simulink library "outp"  (R2021b)
(part 9 of 11)

      link override Signal_Limit/_maxval: Value=KOUTP_CalibratedAccX_G_maxval
      link override Signal_Limit/_minval: Value=KOUTP_CalibratedAccX_G_minval
      link override Signal_Override/_ovrdflg: Value=KOUTP_CalibratedAccX_G_ovrdflg
      link override Signal_Override/_ovrdval: Value=KOUTP_CalibratedAccX_G_ovrdval
  VVMC_CalibratedAccY_G_Inproc : FVT_lib/outp/OverrideAndLimit  SystemSampleTime=-1  VariantActivationTime=update diagram  Latency=0  AutoFrameSizeCalculation=off
      link override Signal_Limit/_maxval: Value=KOUTP_CalibratedAccY_G_maxval
      link override Signal_Limit/_minval: Value=KOUTP_CalibratedAccY_G_minval
      link override Signal_Override/_ovrdflg: Value=KOUTP_CalibratedAccY_G_ovrdflg
      link override Signal_Override/_ovrdval: Value=KOUTP_CalibratedAccY_G_ovrdval
  VVMC_CalibratedAccZ_G_Inproc : FVT_lib/outp/OverrideAndLimit  SystemSampleTime=-1  VariantActivationTime=update diagram  Latency=0  AutoFrameSizeCalculation=off
      link override Signal_Limit/_maxval: Value=KOUTP_CalibratedAccZ_G_maxval
      link override Signal_Limit/_minval: Value=KOUTP_CalibratedAccZ_G_minval
      link override Signal_Override/_ovrdflg: Value=KOUTP_CalibratedAccZ_G_ovrdflg
      link override Signal_Override/_ovrdval: Value=KOUTP_CalibratedAccZ_G_ovrdval
  VVMC_CalibratedGyroX_Dps_Inproc : FVT_lib/outp/OverrideAndLimit  SystemSampleTime=-1  VariantActivationTime=update diagram  Latency=0  AutoFrameSizeCalculation=off
      link override Signal_Limit/_maxval: Value=KOUTP_CalibratedGyroX_Dps_maxval
      link override Signal_Limit/_minval: Value=KOUTP_CalibratedGyroX_Dps_minval
      link override Signal_Override/_ovrdflg: Value=KOUTP_CalibratedGyroX_Dps_ovrdflg
      link override Signal_Override/_ovrdval: Value=KOUTP_CalibratedGyroX_Dps_ovrdval
  VVMC_CalibratedGyroY_Dps_Inproc : FVT_lib/outp/OverrideAndLimit  SystemSampleTime=-1  VariantActivationTime=update diagram  Latency=0  AutoFrameSizeCalculation=off
      link override Signal_Limit/_maxval: Value=KOUTP_CalibratedGyroY_Dps_maxval
      link override Signal_Limit/_minval: Value=KOUTP_CalibratedGyroY_Dps_minval
      link override Signal_Override/_ovrdflg: Value=KOUTP_CalibratedGyroY_Dps_ovrdflg
      link override Signal_Override/_ovrdval: Value=KOUTP_CalibratedGyroY_Dps_ovrdval
  VVMC_CalibratedGyroZ_Dps_Inproc : FVT_lib/outp/OverrideAndLimit  SystemSampleTime=-1  VariantActivationTime=update diagram  Latency=0  AutoFrameSizeCalculation=off
      link override Signal_Limit/_maxval: Value=KOUTP_CalibratedGyroZ_Dps_maxval
      link override Signal_Limit/_minval: Value=KOUTP_CalibratedGyroZ_Dps_minval
      link override Signal_Override/_ovrdflg: Value=KOUTP_CalibratedGyroZ_Dps_ovrdflg
      link override Signal_Override/_ovrdval: Value=KOUTP_CalibratedGyroZ_Dps_ovrdval
  VVMC_DISCReqAcc_mps2_Inproc : FVT_lib/outp/OverrideAndLimit  SystemSampleTime=-1  VariantActivationTime=update diagram  Latency=0  AutoFrameSizeCalculation=off
      link override Signal_Limit/_maxval: Value=KOUTP_DISCReqAcc_mps2_maxval
      link override Signal_Limit/_minval: Value=KOUTP_DISCReqAcc_mps2_minval
      link override Signal_Override/_ovrdflg: Value=KOUTP_DISCReqAcc_mps2_ovrdflg
      link override Signal_Override/_ovrdval: Value=KOUTP_DISCReqAcc_mps2_ovrdval
  VVMC_ExtraMSACtrlSta_enum_Inproc : FVT_lib/outp/OverrideAndLimit  SystemSampleTime=-1  VariantActivationTime=update diagram  Latency=0  AutoFrameSizeCalculation=off
      link override Signal_Limit/_maxval: Value=KOUTP_ExtraMSACtrlSta_enum_maxval
      link override Signal_Limit/_minval: Value=KOUTP_ExtraMSACtrlSta_enum_minval
      link override Signal_Override/_ovrdflg: Value=KOUTP_ExtraMSACtrlSta_enum_ovrdflg
      link override Signal_Override/_ovrdval: Value=KOUTP_ExtraMSACtrlSta_enum_ovrdval
  VVMC_FCMACCmode_enum_Inproc : FVT_lib/outp/OverrideAndLimit  SystemSampleTime=-1  VariantActivationTime=update diagram  Latency=0  AutoFrameSizeCalculation=off
      link override Signal_Limit/_maxval: Value=KOUTP_FCMACCmode_enum_maxval
      link override Signal_Limit/_minval: Value=KOUTP_FCMACCmode_enum_minval
      link override Signal_Override/_ovrdflg: Value=KOUTP_FCMACCmode_enum_ovrdflg
      link override Signal_Override/_ovrdval: Value=KOUTP_FCMACCmode_enum_ovrdval
  VVMC_FCMLDWFault_flg_Inproc : FVT_lib/outp/OverrideAndLimit  SystemSampleTime=-1  VariantActivationTime=update diagram  Latency=0  AutoFrameSizeCalculation=off
      link override Signal_Limit/_maxval: Value=KOUTP_FCMLDWFault_flg_maxval
      link override Signal_Limit/_minval: Value=KOUTP_FCMLDWFault_flg_minval
      link override Signal_Override/_ovrdflg: Value=KOUTP_FCMLDWFault_flg_ovrdflg
      link override Signal_Override/_ovrdval: Value=KOUTP_FCMLDWFault_flg_ovrdval
  VVMC_FCMLDWRequest_enum_Inproc : FVT_lib/outp/OverrideAndLimit  SystemSampleTime=-1  VariantActivationTime=update diagram  Latency=0  AutoFrameSizeCalculation=off
      link override Signal_Limit/_maxval: Value=KOUTP_FCMLDWRequest_enum_maxval
      link override Signal_Limit/_minval: Value=KOUTP_FCMLDWRequest_enum_minval
      link override Signal_Override/_ovrdflg: Value=KOUTP_FCMLDWRequest_enum_ovrdflg
      link override Signal_Override/_ovrdval: Value=KOUTP_FCMLDWRequest_enum_ovrdval
  VVMC_FDCVMCAPSAngleTarget_deg_Inproc : FVT_lib/outp/OverrideAndLimit  SystemSampleTime=-1  VariantActivationTime=update diagram  Latency=0  AutoFrameSizeCalculation=off
      link override Signal_Limit/_maxval: Value=KOUTP_FDCVMCAPSAngleTarget_deg_maxval
      link override Signal_Limit/_minval: Value=KOUTP_FDCVMCAPSAngleTarget_deg_minval
      link override Signal_Override/_ovrdflg: Value=KOUTP_FDCVMCAPSAngleTarget_deg_ovrdflg
      link override Signal_Override/_ovrdval: Value=KOUTP_FDCVMCAPSAngleTarget_deg_ovrdval
  VVMC_FDCVMCAPSRqEPSCtrl_flg_Inproc : FVT_lib/outp/OverrideAndLimit  SystemSampleTime=-1  VariantActivationTime=update diagram  Latency=0  AutoFrameSizeCalculation=off
      link override Signal_Limit/_maxval: Value=KOUTP_FDCVMCAPSRqEPSCtrl_flg_maxval
      link override Signal_Limit/_minval: Value=KOUTP_FDCVMCAPSRqEPSCtrl_flg_minval
      link override Signal_Override/_ovrdflg: Value=KOUTP_FDCVMCAPSRqEPSCtrl_flg_ovrdflg
      link override Signal_Override/_ovrdval: Value=KOUTP_FDCVMCAPSRqEPSCtrl_flg_ovrdval
  VVMC_FDCVMCAPSVRqEPSCtrl_flg_Inproc : FVT_lib/outp/OverrideAndLimit  SystemSampleTime=-1  VariantActivationTime=update diagram  Latency=0  AutoFrameSizeCalculation=off
      link override Signal_Limit/_maxval: Value=KOUTP_FDCVMCAPSVRqEPSCtrl_flg_maxval
      link override Signal_Limit/_minval: Value=KOUTP_FDCVMCAPSVRqEPSCtrl_flg_minval
      link override Signal_Override/_ovrdflg: Value=KOUTP_FDCVMCAPSVRqEPSCtrl_flg_ovrdflg
      link override Signal_Override/_ovrdval: Value=KOUTP_FDCVMCAPSVRqEPSCtrl_flg_ovrdval
  VVMC_FDCVMCAngCtrlTqWtGn_pct_Inproc : FVT_lib/outp/OverrideAndLimit  SystemSampleTime=-1  VariantActivationTime=update diagram  Latency=0  AutoFrameSizeCalculation=off
      link override Signal_Limit/_maxval: Value=KOUTP_FDCVMCAngCtrlTqWtGn_pct_maxval
      link override Signal_Limit/_minval: Value=KOUTP_FDCVMCAngCtrlTqWtGn_pct_minval
      link override Signal_Override/_ovrdflg: Value=KOUTP_FDCVMCAngCtrlTqWtGn_pct_ovrdflg
      link override Signal_Override/_ovrdval: Value=KOUTP_FDCVMCAngCtrlTqWtGn_pct_ovrdval
  VVMC_FDCVMCDrInpTqBstAct_flg_Inproc : FVT_lib/outp/OverrideAndLimit  SystemSampleTime=-1  VariantActivationTime=update diagram  Latency=0  AutoFrameSizeCalculation=off
      link override Signal_Limit/_maxval: Value=KOUTP_FDCVMCDrInpTqBstAct_flg_maxval
      link override Signal_Limit/_minval: Value=KOUTP_FDCVMCDrInpTqBstAct_flg_minval
      link override Signal_Override/_ovrdflg: Value=KOUTP_FDCVMCDrInpTqBstAct_flg_ovrdflg
      link override Signal_Override/_ovrdval: Value=KOUTP_FDCVMCDrInpTqBstAct_flg_ovrdval
  VVMC_FDCVMCDrInpTqBstGn_pct_Inproc : FVT_lib/outp/OverrideAndLimit  SystemSampleTime=-1  VariantActivationTime=update diagram  Latency=0  AutoFrameSizeCalculation=off
      link override Signal_Limit/_maxval: Value=KOUTP_FDCVMCDrInpTqBstGn_pct_maxval
      link override Signal_Limit/_minval: Value=KOUTP_FDCVMCDrInpTqBstGn_pct_minval
      link override Signal_Override/_ovrdflg: Value=KOUTP_FDCVMCDrInpTqBstGn_pct_ovrdflg
      link override Signal_Override/_ovrdval: Value=KOUTP_FDCVMCDrInpTqBstGn_pct_ovrdval
  VVMC_FDCVMCMaxAngCtrlOutTqLim_Nm_Inproc : FVT_lib/outp/OverrideAndLimit  SystemSampleTime=-1  VariantActivationTime=update diagram  Latency=0  AutoFrameSizeCalculation=off
      link override Signal_Limit/_maxval: Value=KOUTP_FDCVMCMaxAngCtrlOutTqLim_Nm_maxval
      link override Signal_Limit/_minval: Value=KOUTP_FDCVMCMaxAngCtrlOutTqLim_Nm_minval
      link override Signal_Override/_ovrdflg: Value=KOUTP_FDCVMCMaxAngCtrlOutTqLim_Nm_ovrdflg
      link override Signal_Override/_ovrdval: Value=KOUTP_FDCVMCMaxAngCtrlOutTqLim_Nm_ovrdval
  VVMC_FeatArbitrFinal_enum_Inproc : FVT_lib/outp/OverrideAndLimit  SystemSampleTime=-1  VariantActivationTime=update diagram  Latency=0  AutoFrameSizeCalculation=off
      link override Signal_Limit/_maxval: Value=KOUTP_FeatArbitrFinal_enum_maxval
      link override Signal_Limit/_minval: Value=KOUTP_FeatArbitrFinal_enum_minval
      link override Signal_Override/_ovrdflg: Value=KOUTP_FeatArbitrFinal_enum_ovrdflg
      link override Signal_Override/_ovrdval: Value=KOUTP_FeatArbitrFinal_enum_ovrdval
  VVMC_FeatArbitrSta_enum_Inproc : FVT_lib/outp/OverrideAndLimit  SystemSampleTime=-1  VariantActivationTime=update diagram  Latency=0  AutoFrameSizeCalculation=off
      link override Signal_Limit/_maxval: Value=KOUTP_FeatArbitrSta_enum_maxval
      link override Signal_Limit/_minval: Value=KOUTP_FeatArbitrSta_enum_minval
      link override Signal_Override/_ovrdflg: Value=KOUTP_FeatArbitrSta_enum_ovrdflg
      link override Signal_Override/_ovrdval: Value=KOUTP_FeatArbitrSta_enum_ovrdval
  VVMC_FeatReqSpd_kph_Inproc : FVT_lib/outp/OverrideAndLimit  SystemSampleTime=-1  VariantActivationTime=update diagram  Latency=0  AutoFrameSizeCalculation=off
      link override Signal_Limit/_maxval: Value=KOUTP_FeatReqSpd_kph_maxval
      link override Signal_Limit/_minval: Value=KOUTP_FeatReqSpd_kph_minval
      link override Signal_Override/_ovrdflg: Value=KOUTP_FeatReqSpd_kph_ovrdflg
      link override Signal_Override/_ovrdval: Value=KOUTP_FeatReqSpd_kph_ovrdval
  VVMC_FeatSetSpdFinal_raw32_Inproc : FVT_lib/outp/OverrideAndLimit  SystemSampleTime=-1  VariantActivationTime=update diagram  Latency=0  AutoFrameSizeCalculation=off
      link override Signal_Limit/_maxval: Value=KOUTP_FeatSetSpdFinal_raw32_maxval
      link override Signal_Limit/_minval: Value=KOUTP_FeatSetSpdFinal_raw32_minval
      link override Signal_Override/_ovrdflg: Value=KOUTP_FeatSetSpdFinal_raw32_ovrdflg
      link override Signal_Override/_ovrdval: Value=KOUTP_FeatSetSpdFinal_raw32_ovrdval
  VVMC_ForceLowBeam_enum_Inproc : FVT_lib/outp/OverrideAndLimit  SystemSampleTime=-1  VariantActivationTime=update diagram  Latency=0  AutoFrameSizeCalculation=off
      link override Signal_Limit/_maxval: Value=KOUTP_ForceLowBeam_enum_maxval
      link override Signal_Limit/_minval: Value=KOUTP_ForceLowBeam_enum_minval
      link override Signal_Override/_ovrdflg: Value=KOUTP_ForceLowBeam_enum_ovrdflg
      link override Signal_Override/_ovrdval: Value=KOUTP_ForceLowBeam_enum_ovrdval
  VVMC_FrontRearSlipRatioCtrl_flg_Inproc : FVT_lib/outp/OverrideAndLimit  SystemSampleTime=-1  VariantActivationTime=update diagram  Latency=0  AutoFrameSizeCalculation=off
      link override Signal_Limit/_maxval: Value=KOUTP_FrontRearSlipRatioCtrl_flg_maxval
      link override Signal_Limit/_minval: Value=KOUTP_FrontRearSlipRatioCtrl_flg_minval
      link override Signal_Override/_ovrdflg: Value=KOUTP_FrontRearSlipRatioCtrl_flg_ovrdflg
      link override Signal_Override/_ovrdval: Value=KOUTP_FrontRearSlipRatioCtrl_flg_ovrdval
  VVMC_HazardWarningReq_flg_Inproc : FVT_lib/outp/OverrideAndLimit  SystemSampleTime=-1  VariantActivationTime=update diagram  Latency=0  AutoFrameSizeCalculation=off
      link override Signal_Limit/_maxval: Value=KOUTP_HazardWarningReq_flg_maxval
      link override Signal_Limit/_minval: Value=KOUTP_HazardWarningReq_flg_minval
      link override Signal_Override/_ovrdflg: Value=KOUTP_HazardWarningReq_flg_ovrdflg
      link override Signal_Override/_ovrdval: Value=KOUTP_HazardWarningReq_flg_ovrdval
  VVMC_IMUEnaCmd_flg_Inproc : FVT_lib/outp/OverrideAndLimit  SystemSampleTime=-1  VariantActivationTime=update diagram  Latency=0  AutoFrameSizeCalculation=off
      link override Signal_Limit/_maxval: Value=KOUTP_IMUEnaCmd_flg_maxval
      link override Signal_Limit/_minval: Value=KOUTP_IMUEnaCmd_flg_minval
      link override Signal_Override/_ovrdflg: Value=KOUTP_IMUEnaCmd_flg_ovrdflg
      link override Signal_Override/_ovrdval: Value=KOUTP_IMUEnaCmd_flg_ovrdval
  VVMC_ISOAccLimit_mps2_Inproc : FVT_lib/outp/OverrideAndLimit  SystemSampleTime=-1  VariantActivationTime=update diagram  Latency=0  AutoFrameSizeCalculation=off
      link override Signal_Limit/_maxval: Value=KOUTP_ISOAccLimit_mps2_maxval
      link override Signal_Limit/_minval: Value=KOUTP_ISOAccLimit_mps2_minval
      link override Signal_Override/_ovrdflg: Value=KOUTP_ISOAccLimit_mps2_ovrdflg
      link override Signal_Override/_ovrdval: Value=KOUTP_ISOAccLimit_mps2_ovrdval
  VVMC_ISODecLimit_mps2_Inproc : FVT_lib/outp/OverrideAndLimit  SystemSampleTime=-1  VariantActivationTime=update diagram  Latency=0  AutoFrameSizeCalculation=off
      link override Signal_Limit/_maxval: Value=KOUTP_ISODecLimit_mps2_maxval
      link override Signal_Limit/_minval: Value=KOUTP_ISODecLimit_mps2_minval
      link override Signal_Override/_ovrdflg: Value=KOUTP_ISODecLimit_mps2_ovrdflg
      link override Signal_Override/_ovrdval: Value=KOUTP_ISODecLimit_mps2_ovrdval
  VVMC_ISOJerkLimit_mps3_Inproc : FVT_lib/outp/OverrideAndLimit  SystemSampleTime=-1  VariantActivationTime=update diagram  Latency=0  AutoFrameSizeCalculation=off
      link override Signal_Limit/_maxval: Value=KOUTP_ISOJerkLimit_mps3_maxval
      link override Signal_Limit/_minval: Value=KOUTP_ISOJerkLimit_mps3_minval
      link override Signal_Override/_ovrdflg: Value=KOUTP_ISOJerkLimit_mps3_ovrdflg
      link override Signal_Override/_ovrdval: Value=KOUTP_ISOJerkLimit_mps3_ovrdval
  VVMC_JerkPCT_pct_Inproc : FVT_lib/outp/OverrideAndLimit  SystemSampleTime=-1  VariantActivationTime=update diagram  Latency=0  AutoFrameSizeCalculation=off
      link override Signal_Limit/_maxval: Value=KOUTP_JerkPCT_pct_maxval
      link override Signal_Limit/_minval: Value=KOUTP_JerkPCT_pct_minval
      link override Signal_Override/_ovrdflg: Value=KOUTP_JerkPCT_pct_ovrdflg
      link override Signal_Override/_ovrdval: Value=KOUTP_JerkPCT_pct_ovrdval
  VVMC_LKAHODDisplayWarning_flg_Inproc : FVT_lib/outp/OverrideAndLimit  SystemSampleTime=-1  VariantActivationTime=update diagram  Latency=0  AutoFrameSizeCalculation=off
      link override Signal_Limit/_maxval: Value=KOUTP_LKAHODDisplayWarning_flg_maxval
      link override Signal_Limit/_minval: Value=KOUTP_LKAHODDisplayWarning_flg_minval
      link override Signal_Override/_ovrdflg: Value=KOUTP_LKAHODDisplayWarning_flg_ovrdflg
      link override Signal_Override/_ovrdval: Value=KOUTP_LKAHODDisplayWarning_flg_ovrdval
  VVMC_LKAHODSoundWarning_flg_Inproc : FVT_lib/outp/OverrideAndLimit  SystemSampleTime=-1  VariantActivationTime=update diagram  Latency=0  AutoFrameSizeCalculation=off
      link override Signal_Limit/_maxval: Value=KOUTP_LKAHODSoundWarning_flg_maxval
      link override Signal_Limit/_minval: Value=KOUTP_LKAHODSoundWarning_flg_minval
      link override Signal_Override/_ovrdflg: Value=KOUTP_LKAHODSoundWarning_flg_ovrdflg
      link override Signal_Override/_ovrdval: Value=KOUTP_LKAHODSoundWarning_flg_ovrdval
  VVMC_LKAStrToqReq_Nm_Inproc : FVT_lib/outp/OverrideAndLimit  SystemSampleTime=-1  VariantActivationTime=update diagram  Latency=0  AutoFrameSizeCalculation=off
      link override Signal_Limit/_maxval: Value=KOUTP_LKAStrToqReq_Nm_maxval
      link override Signal_Limit/_minval: Value=KOUTP_LKAStrToqReq_Nm_minval
      link override Signal_Override/_ovrdflg: Value=KOUTP_LKAStrToqReq_Nm_ovrdflg
      link override Signal_Override/_ovrdval: Value=KOUTP_LKAStrToqReq_Nm_ovrdval
  VVMC_LKATOIAct_enum_Inproc : FVT_lib/outp/OverrideAndLimit  SystemSampleTime=-1  VariantActivationTime=update diagram  Latency=0  AutoFrameSizeCalculation=off
      link override Signal_Limit/_maxval: Value=KOUTP_LKATOIAct_enum_maxval
      link override Signal_Limit/_minval: Value=KOUTP_LKATOIAct_enum_minval
      link override Signal_Override/_ovrdflg: Value=KOUTP_LKATOIAct_enum_ovrdflg
      link override Signal_Override/_ovrdval: Value=KOUTP_LKATOIAct_enum_ovrdval
  VVMC_LKATOIFault_flg_Inproc : FVT_lib/outp/OverrideAndLimit  SystemSampleTime=-1  VariantActivationTime=update diagram  Latency=0  AutoFrameSizeCalculation=off
      link override Signal_Limit/_maxval: Value=KOUTP_LKATOIFault_flg_maxval
      link override Signal_Limit/_minval: Value=KOUTP_LKATOIFault_flg_minval
      link override Signal_Override/_ovrdflg: Value=KOUTP_LKATOIFault_flg_ovrdflg
      link override Signal_Override/_ovrdval: Value=KOUTP_LKATOIFault_flg_ovrdval
  VVMC_LVDAACCStatusInformation_flg_Inproc : FVT_lib/outp/OverrideAndLimit  SystemSampleTime=-1  VariantActivationTime=update diagram  Latency=0  AutoFrameSizeCalculation=off
      link override Signal_Limit/_maxval: Value=KOUTP_LVDAACCStatusInformation_flg_maxval
      link override Signal_Limit/_minval: Value=KOUTP_LVDAACCStatusInformation_flg_minval
      link override Signal_Override/_ovrdflg: Value=KOUTP_LVDAACCStatusInformation_flg_ovrdflg
      link override Signal_Override/_ovrdval: Value=KOUTP_LVDAACCStatusInformation_flg_ovrdval
  VVMC_LVDADisabled_flg_Inproc : FVT_lib/outp/OverrideAndLimit  SystemSampleTime=-1  VariantActivationTime=update diagram  Latency=0  AutoFrameSizeCalculation=off
      link override Signal_Limit/_maxval: Value=KOUTP_LVDADisabled_flg_maxval
      link override Signal_Limit/_minval: Value=KOUTP_LVDADisabled_flg_minval
      link override Signal_Override/_ovrdflg: Value=KOUTP_LVDADisabled_flg_ovrdflg
      link override Signal_Override/_ovrdval: Value=KOUTP_LVDADisabled_flg_ovrdval
  VVMC_LVDAFailinfo_flg_Inproc : FVT_lib/outp/OverrideAndLimit  SystemSampleTime=-1  VariantActivationTime=update diagram  Latency=0  AutoFrameSizeCalculation=off
      link override Signal_Limit/_maxval: Value=KOUTP_LVDAFailinfo_flg_maxval
      link override Signal_Limit/_minval: Value=KOUTP_LVDAFailinfo_flg_minval
      link override Signal_Override/_ovrdflg: Value=KOUTP_LVDAFailinfo_flg_ovrdflg
      link override Signal_Override/_ovrdval: Value=KOUTP_LVDAFailinfo_flg_ovrdval
  VVMC_LVDAMuteSta_enum_Inproc : FVT_lib/outp/OverrideAndLimit  SystemSampleTime=-1  VariantActivationTime=update diagram  Latency=0  AutoFrameSizeCalculation=off
      link override Signal_Limit/_maxval: Value=KOUTP_LVDAMuteSta_enum_maxval
      link override Signal_Limit/_minval: Value=KOUTP_LVDAMuteSta_enum_minval
      link override Signal_Override/_ovrdflg: Value=KOUTP_LVDAMuteSta_enum_ovrdflg
      link override Signal_Override/_ovrdval: Value=KOUTP_LVDAMuteSta_enum_ovrdval
  VVMC_LVDAWarning_flg_Inproc : FVT_lib/outp/OverrideAndLimit  SystemSampleTime=-1  VariantActivationTime=update diagram  Latency=0  AutoFrameSizeCalculation=off
      link override Signal_Limit/_maxval: Value=KOUTP_LVDAWarning_flg_maxval
      link override Signal_Limit/_minval: Value=KOUTP_LVDAWarning_flg_minval
      link override Signal_Override/_ovrdflg: Value=KOUTP_LVDAWarning_flg_ovrdflg
      link override Signal_Override/_ovrdval: Value=KOUTP_LVDAWarning_flg_ovrdval
  VVMC_LatAccCtrl_flg_Inproc : FVT_lib/outp/OverrideAndLimit  SystemSampleTime=-1  VariantActivationTime=update diagram  Latency=0  AutoFrameSizeCalculation=off
      link override Signal_Limit/_maxval: Value=KOUTP_LatAccCtrl_flg_maxval
      link override Signal_Limit/_minval: Value=KOUTP_LatAccCtrl_flg_minval
      link override Signal_Override/_ovrdflg: Value=KOUTP_LatAccCtrl_flg_ovrdflg
      link override Signal_Override/_ovrdval: Value=KOUTP_LatAccCtrl_flg_ovrdval
  VVMC_LateralCtrl_flg_Inproc : FVT_lib/outp/OverrideAndLimit  SystemSampleTime=-1  VariantActivationTime=update diagram  Latency=0  AutoFrameSizeCalculation=off
      link override Signal_Limit/_maxval: Value=KOUTP_LateralCtrl_flg_maxval
      link override Signal_Limit/_minval: Value=KOUTP_LateralCtrl_flg_minval
      link override Signal_Override/_ovrdflg: Value=KOUTP_LateralCtrl_flg_ovrdflg
      link override Signal_Override/_ovrdval: Value=KOUTP_LateralCtrl_flg_ovrdval
  VVMC_LeftTurnLightReq_flg_Inproc : FVT_lib/outp/OverrideAndLimit  SystemSampleTime=-1  VariantActivationTime=update diagram  Latency=0  AutoFrameSizeCalculation=off
      link override Signal_Limit/_maxval: Value=KOUTP_LeftTurnLightReq_flg_maxval
      link override Signal_Limit/_minval: Value=KOUTP_LeftTurnLightReq_flg_minval
      link override Signal_Override/_ovrdflg: Value=KOUTP_LeftTurnLightReq_flg_ovrdflg
      link override Signal_Override/_ovrdval: Value=KOUTP_LeftTurnLightReq_flg_ovrdval
  VVMC_LimitPCT_pct_Inproc : FVT_lib/outp/OverrideAndLimit  SystemSampleTime=-1  VariantActivationTime=update diagram  Latency=0  AutoFrameSizeCalculation=off
      link override Signal_Limit/_maxval: Value=KOUTP_LimitPCT_pct_maxval
      link override Signal_Limit/_minval: Value=KOUTP_LimitPCT_pct_minval
      link override Signal_Override/_ovrdflg: Value=KOUTP_LimitPCT_pct_ovrdflg
      link override Signal_Override/_ovrdval: Value=KOUTP_LimitPCT_pct_ovrdval
  VVMC_LongAcc_Gps_Inproc : FVT_lib/outp/OverrideAndLimit  SystemSampleTime=-1  VariantActivationTime=update diagram  Latency=0  AutoFrameSizeCalculation=off
      link override Signal_Limit/_maxval: Value=KOUTP_LongAcc_Gps_maxval
      link override Signal_Limit/_minval: Value=KOUTP_LongAcc_Gps_minval
      link override Signal_Override/_ovrdflg: Value=KOUTP_LongAcc_Gps_ovrdflg
      link override Signal_Override/_ovrdval: Value=KOUTP_LongAcc_Gps_ovrdval
  VVMC_MSACtrlSta_enum_Inproc : FVT_lib/outp/OverrideAndLimit  SystemSampleTime=-1  VariantActivationTime=update diagram  Latency=0  AutoFrameSizeCalculation=off
      link override Signal_Limit/_maxval: Value=KOUTP_MSACtrlSta_enum_maxval
      link override Signal_Limit/_minval: Value=KOUTP_MSACtrlSta_enum_minval
      link override Signal_Override/_ovrdflg: Value=KOUTP_MSACtrlSta_enum_ovrdflg
      link override Signal_Override/_ovrdval: Value=KOUTP_MSACtrlSta_enum_ovrdval
  VVMC_MeterIndSpeed_raw32_Inproc : FVT_lib/outp/OverrideAndLimit  SystemSampleTime=-1  VariantActivationTime=update diagram  Latency=0  AutoFrameSizeCalculation=off
      link override Signal_Limit/_maxval: Value=KOUTP_MeterIndSpeed_raw32_maxval
      link override Signal_Limit/_minval: Value=KOUTP_MeterIndSpeed_raw32_minval
      link override Signal_Override/_ovrdflg: Value=KOUTP_MeterIndSpeed_raw32_ovrdflg
      link override Signal_Override/_ovrdval: Value=KOUTP_MeterIndSpeed_raw32_ovrdval
  VVMC_RearWhlSlipRatioCtrl_flg_Inproc : FVT_lib/outp/OverrideAndLimit  SystemSampleTime=-1  VariantActivationTime=update diagram  Latency=0  AutoFrameSizeCalculation=off
      link override Signal_Limit/_maxval: Value=KOUTP_RearWhlSlipRatioCtrl_flg_maxval
      link override Signal_Limit/_minval: Value=KOUTP_RearWhlSlipRatioCtrl_flg_minval
      link override Signal_Override/_ovrdflg: Value=KOUTP_RearWhlSlipRatioCtrl_flg_ovrdflg
      link override Signal_Override/_ovrdval: Value=KOUTP_RearWhlSlipRatioCtrl_flg_ovrdval
  VVMC_RightTurnLightReq_flg_Inproc : FVT_lib/outp/OverrideAndLimit  SystemSampleTime=-1  VariantActivationTime=update diagram  Latency=0  AutoFrameSizeCalculation=off
      link override Signal_Limit/_maxval: Value=KOUTP_RightTurnLightReq_flg_maxval
      link override Signal_Limit/_minval: Value=KOUTP_RightTurnLightReq_flg_minval
      link override Signal_Override/_ovrdflg: Value=KOUTP_RightTurnLightReq_flg_ovrdflg
      link override Signal_Override/_ovrdval: Value=KOUTP_RightTurnLightReq_flg_ovrdval
  VVMC_SPD2ACCAct_flg_Inproc : FVT_lib/outp/OverrideAndLimit  SystemSampleTime=-1  VariantActivationTime=update diagram  Latency=0  AutoFrameSizeCalculation=off
      link override Signal_Limit/_maxval: Value=KOUTP_SPD2ACCAct_flg_maxval
      link override Signal_Limit/_minval: Value=KOUTP_SPD2ACCAct_flg_minval
      link override Signal_Override/_ovrdflg: Value=KOUTP_SPD2ACCAct_flg_ovrdflg
      link override Signal_Override/_ovrdval: Value=KOUTP_SPD2ACCAct_flg_ovrdval
  VVMC_SafetyCtrl_flg_Inproc : FVT_lib/outp/OverrideAndLimit  SystemSampleTime=-1  VariantActivationTime=update diagram  Latency=0  AutoFrameSizeCalculation=off
      link override Signal_Limit/_maxval: Value=KOUTP_SafetyCtrl_flg_maxval
      link override Signal_Limit/_minval: Value=KOUTP_SafetyCtrl_flg_minval
      link override Signal_Override/_ovrdflg: Value=KOUTP_SafetyCtrl_flg_ovrdflg
      link override Signal_Override/_ovrdval: Value=KOUTP_SafetyCtrl_flg_ovrdval
  VVMC_SingleWhlSlipRatioCtrl_flg_Inproc : FVT_lib/outp/OverrideAndLimit  SystemSampleTime=-1  VariantActivationTime=update diagram  Latency=0  AutoFrameSizeCalculation=off
      link override Signal_Limit/_maxval: Value=KOUTP_SingleWhlSlipRatioCtrl_flg_maxval
      link override Signal_Limit/_minval: Value=KOUTP_SingleWhlSlipRatioCtrl_flg_minval
      link override Signal_Override/_ovrdflg: Value=KOUTP_SingleWhlSlipRatioCtrl_flg_ovrdflg
      link override Signal_Override/_ovrdval: Value=KOUTP_SingleWhlSlipRatioCtrl_flg_ovrdval
  VVMC_TargetType_enum_Inproc : FVT_lib/outp/OverrideAndLimit  SystemSampleTime=-1  VariantActivationTime=update diagram  Latency=0  AutoFrameSizeCalculation=off
      link override Signal_Limit/_maxval: Value=KOUTP_TargetType_enum_maxval
      link override Signal_Limit/_minval: Value=KOUTP_TargetType_enum_minval
      link override Signal_Override/_ovrdflg: Value=KOUTP_TargetType_enum_ovrdflg
      link override Signal_Override/_ovrdval: Value=KOUTP_TargetType_enum_ovrdval
  VVMC_TimeGapCalcu_s_Inproc : FVT_lib/outp/OverrideAndLimit  SystemSampleTime=-1  VariantActivationTime=update diagram  Latency=0  AutoFrameSizeCalculation=off
      link override Signal_Limit/_maxval: Value=KOUTP_TimeGapCalcu_s_maxval
      link override Signal_Limit/_minval: Value=KOUTP_TimeGapCalcu_s_minval
      link override Signal_Override/_ovrdflg: Value=KOUTP_TimeGapCalcu_s_ovrdflg
      link override Signal_Override/_ovrdval: Value=KOUTP_TimeGapCalcu_s_ovrdval
  VVMC_TimeGapLevel_enum_Inproc : FVT_lib/outp/OverrideAndLimit  SystemSampleTime=-1  VariantActivationTime=update diagram  Latency=0  AutoFrameSizeCalculation=off
      link override Signal_Limit/_maxval: Value=KOUTP_TimeGapLevel_enum_maxval
      link override Signal_Limit/_minval: Value=KOUTP_TimeGapLevel_enum_minval
      link override Signal_Override/_ovrdflg: Value=KOUTP_TimeGapLevel_enum_ovrdflg
      link override Signal_Override/_ovrdval: Value=KOUTP_TimeGapLevel_enum_ovrdval
  VVMC_VMCACCCtrlAvail_flg_Inproc : FVT_lib/outp/OverrideAndLimit  SystemSampleTime=-1  VariantActivationTime=update diagram  Latency=0  AutoFrameSizeCalculation=off
      link override Signal_Limit/_maxval: Value=KOUTP_VMCACCCtrlAvail_flg_maxval
      link override Signal_Limit/_minval: Value=KOUTP_VMCACCCtrlAvail_flg_minval
      link override Signal_Override/_ovrdflg: Value=KOUTP_VMCACCCtrlAvail_flg_ovrdflg
      link override Signal_Override/_ovrdval: Value=KOUTP_VMCACCCtrlAvail_flg_ovrdval
  VVMC_VMCAEBCtrlAvail_flg_Inproc : FVT_lib/outp/OverrideAndLimit  SystemSampleTime=-1  VariantActivationTime=update diagram  Latency=0  AutoFrameSizeCalculation=off
      link override Signal_Limit/_maxval: Value=KOUTP_VMCAEBCtrlAvail_flg_maxval
      link override Signal_Limit/_minval: Value=KOUTP_VMCAEBCtrlAvail_flg_minval
      link override Signal_Override/_ovrdflg: Value=KOUTP_VMCAEBCtrlAvail_flg_ovrdflg
      link override Signal_Override/_ovrdval: Value=KOUTP_VMCAEBCtrlAvail_flg_ovrdval
  VVMC_VMCCCCtrlAvail_flg_Inproc : FVT_lib/outp/OverrideAndLimit  SystemSampleTime=-1  VariantActivationTime=update diagram  Latency=0  AutoFrameSizeCalculation=off
      link override Signal_Limit/_maxval: Value=KOUTP_VMCCCCtrlAvail_flg_maxval
      link override Signal_Limit/_minval: Value=KOUTP_VMCCCCtrlAvail_flg_minval
      link override Signal_Override/_ovrdflg: Value=KOUTP_VMCCCCtrlAvail_flg_ovrdflg
      link override Signal_Override/_ovrdval: Value=KOUTP_VMCCCCtrlAvail_flg_ovrdval
  VVMC_VMCMSACtrlAvail_flg_Inproc : FVT_lib/outp/OverrideAndLimit  SystemSampleTime=-1  VariantActivationTime=update diagram  Latency=0  AutoFrameSizeCalculation=off
      link override Signal_Limit/_maxval: Value=KOUTP_VMCMSACtrlAvail_flg_maxval
      link override Signal_Limit/_minval: Value=KOUTP_VMCMSACtrlAvail_flg_minval
      link override Signal_Override/_ovrdflg: Value=KOUTP_VMCMSACtrlAvail_flg_ovrdflg
      link override Signal_Override/_ovrdval: Value=KOUTP_VMCMSACtrlAvail_flg_ovrdval
  VVMC_VehicleSpeed_kph_Inproc : FVT_lib/outp/OverrideAndLimit  SystemSampleTime=-1  VariantActivationTime=update diagram  Latency=0  AutoFrameSizeCalculation=off
      link override Signal_Limit/_maxval: Value=KOUTP_VehicleSpeed_kph_maxval
      link override Signal_Limit/_minval: Value=KOUTP_VehicleSpeed_kph_minval
      link override Signal_Override/_ovrdflg: Value=KOUTP_VehicleSpeed_kph_ovrdflg
      link override Signal_Override/_ovrdval: Value=KOUTP_VehicleSpeed_kph_ovrdval
  VVMC_VehicleSpeed_mph_Inproc : FVT_lib/outp/OverrideAndLimit  SystemSampleTime=-1  VariantActivationTime=update diagram  Latency=0  AutoFrameSizeCalculation=off
      link override Signal_Limit/_maxval: Value=KOUTP_VehicleSpeed_mph_maxval
      link override Signal_Limit/_minval: Value=KOUTP_VehicleSpeed_mph_minval
      link override Signal_Override/_ovrdflg: Value=KOUTP_VehicleSpeed_mph_ovrdflg
      link override Signal_Override/_ovrdval: Value=KOUTP_VehicleSpeed_mph_ovrdval
  VOUTP_HVTHCMSysAvail_enum : Outport
  VOUTP_LVBattVoltSta_enum : Outport  Port=2
  VOUTP_VehHVPwrAvail4THCM_W : Outport  Port=3
  VOUTP_VehSpeed_kph : Outport  Port=4
  VOUTP_VehSpeedTimeOut_flg : Outport  Port=5
  VOUTP_FSOffSw_enum : Outport  Port=6
  VOUTP_FSOffSwTimeOut_flg : Outport  Port=7
  VOUTP_ChrgPlugSta_enum : Outport  Port=8
  VOUTP_PASDRMR_cm : Outport  Port=9
  VOUTP_PASDRML_cm : Outport  Port=10
  VOUTP_PASDRCR_cm : Outport  Port=11
  VOUTP_PASDRCL_cm : Outport  Port=12
  VOUTP_PASDFMR_cm : Outport  Port=13
  VOUTP_PASDFML_cm : Outport  Port=14
  VOUTP_PASDFCR_cm : Outport  Port=15
  VOUTP_PASDFCL_cm : Outport  Port=16
  VOUTP_APSDRLR_cm : Outport  Port=17
  VOUTP_APSDRLL_cm : Outport  Port=18
  VOUTP_APSDFLR_cm : Outport  Port=19
  VOUTP_APSDFLL_cm : Outport  Port=20
  VOUTP_PASAFCL_enum : Outport  Port=21
  VOUTP_PASARMR_enum : Outport  Port=22
  VOUTP_PASARML_enum : Outport  Port=23
  VOUTP_PASARCR_enum : Outport  Port=24
  VOUTP_PASARCL_enum : Outport  Port=25
  VOUTP_PASAFMR_enum : Outport  Port=26
  VOUTP_PASAFML_enum : Outport  Port=27
  VOUTP_PASAFCR_enum : Outport  Port=28
  VOUTP_USSStaRMR_flg : Outport  Port=29
  VOUTP_USSStaRML_flg : Outport  Port=30
  VOUTP_USSStaRLR_flg : Outport  Port=31
  VOUTP_USSStaRLL_flg : Outport  Port=32
  VOUTP_USSStaRCR_flg : Outport  Port=33
  VOUTP_USSStaRCL_flg : Outport  Port=34
  VOUTP_USSStaFMR_flg : Outport  Port=35
  VOUTP_USSStaFML_flg : Outport  Port=36
  VOUTP_USSStaFLR_flg : Outport  Port=37
  VOUTP_USSStaFLL_flg : Outport  Port=38
  VOUTP_USSStaFCR_flg : Outport  Port=39
  VOUTP_USSStaFCL_flg : Outport  Port=40
  VOUTP_Chime_enum : Outport  Port=41
  VOUTP_SNSRLayout_enum : Outport  Port=42
  VOUTP_StaFSya_flg : Outport  Port=43
  VOUTP_ModOperation_enum : Outport  Port=44
  VOUTP_BrkPedalPos_pct : Outport  Port=45
  VOUTP_BrkPedalPosTimeOut_flg : Outport  Port=46
  VOUTP_LFRawWhlSpeed_kph : Outport  Port=47
  VOUTP_LFRawWhlSpeedTimeOut_flg : Outport  Port=48
  VOUTP_RFRawWhlSpeed_kph : Outport  Port=49
  VOUTP_RFRawWhlSpeedTimeOut_flg : Outport  Port=50
  VOUTP_LRRawWhlSpeed_kph : Outport  Port=51
  VOUTP_LRRawWhlSpeedTimeOut_flg : Outport  Port=52
  VOUTP_RRRawWhlSpeed_kph : Outport  Port=53
  VOUTP_RRRawWhlSpeedTimeOut_flg : Outport  Port=54
  VOUTP_LFRawWhlSpeedV_flg : Outport  Port=55
  VOUTP_LFRawWhlSpeedVTimeOut_flg : Outport  Port=56
  VOUTP_RFRawWhlSpeedV_flg : Outport  Port=57
  VOUTP_RFRawWhlSpeedVTimeOut_flg : Outport  Port=58
  VOUTP_LRRawWhlSpeedV_flg : Outport  Port=59
  VOUTP_LRRawWhlSpeedVTimeOut_flg : Outport  Port=60
  VOUTP_RRRawWhlSpeedV_flg : Outport  Port=61
  VOUTP_RRRawWhlSpeedVTimeOut_flg : Outport  Port=62
  VOUTP_LFWhlRotDir_enum : Outport  Port=63
  VOUTP_LFWhlRotDirTimeOut_flg : Outport  Port=64
  VOUTP_RFWhlRotDir_enum : Outport  Port=65
  VOUTP_RFWhlRotDirTimeOut_flg : Outport  Port=66
  VOUTP_LRWhlRotDir_enum : Outport  Port=67
  VOUTP_LRWhlRotDirTimeOut_flg : Outport  Port=68
  VOUTP_RRWhlRotDir_enum : Outport  Port=69
  VOUTP_RRWhlRotDirTimeOut_flg : Outport  Port=70
  VOUTP_LFPulseCountV_flg : Outport  Port=71
  VOUTP_LFPulseCountVTimeOut_flg : Outport  Port=72
  VOUTP_RFPulseCountV_flg : Outport  Port=73
  VOUTP_RFPulseCountVTimeOut_flg : Outport  Port=74
  VOUTP_LRPulseCountV_flg : Outport  Port=75
  VOUTP_LRPulseCountVTimeOut_flg : Outport  Port=76
  VOUTP_RRPulseCountV_flg : Outport  Port=77
  VOUTP_RRPulseCountVTimeOut_flg : Outport  Port=78
  VOUTP_LFPulseCount_enum : Outport  Port=79
  VOUTP_LFPulseCountTimeOut_flg : Outport  Port=80
  VOUTP_RFPulseCount_enum : Outport  Port=81
  VOUTP_RFPulseCountTimeOut_flg : Outport  Port=82
  VOUTP_LRPulseCount_enum : Outport  Port=83
  VOUTP_LRPulseCountTimeOut_flg : Outport  Port=84
  VOUTP_RRPulseCount_enum : Outport  Port=85
  VOUTP_RRPulseCountTimeOut_flg : Outport  Port=86
  VOUTP_ShifterHandleCmd_enum : Outport  Port=87
  VOUTP_ShifterHandleCmdTimeOut_flg : Outport  Port=88
  VOUTP_DriIntend_enum : Outport  Port=89
  VOUTP_DriIntendTimeOut_flg : Outport  Port=90
  VOUTP_EPSAOIControl_enum : Outport  Port=91
  VOUTP_EPSAOIControlTimeOut_flg : Outport  Port=92
  VOUTP_SASAngle_Deg : Outport  Port=93
  VOUTP_SASAngleTimeOut_flg : Outport  Port=94
  VOUTP_SASSpeed_degps : Outport  Port=95
  VOUTP_SASSpeedTimeOut_flg : Outport  Port=96
  VOUTP_SASSpeedValid_flg : Outport  Port=97
  VOUTP_SASSpeedValidTimeOut_flg : Outport  Port=98
  VOUTP_SASCAL_flg : Outport  Port=99
  VOUTP_SASCALTimeOut_flg : Outport  Port=100
  VOUTP_SASV_flg : Outport  Port=101
  VOUTP_SASVTimeOut_flg : Outport  Port=102
  VOUTP_GRADE_Deg : Outport  Port=103
  VOUTP_GRADETimeOut_flg : Outport  Port=104
  VOUTP_YawRate_degps : Outport  Port=105
  VOUTP_YawRateTimeOut_flg : Outport  Port=106
  VOUTP_LatAccel_Gps : Outport  Port=107
  VOUTP_LatAccelTimeOut_flg : Outport  Port=108
  VOUTP_LongAccel_Gps : Outport  Port=109
  VOUTP_LongAccelTimeOut_flg : Outport  Port=110
  VOUTP_MCPressure_bar : Outport  Port=111
  VOUTP_MCPressureTimeOut_flg : Outport  Port=112
  VOUTP_YawRateV_flg : Outport  Port=113
  VOUTP_YawRateVTimeOut_flg : Outport  Port=114
  VOUTP_LatAccelV_flg : Outport  Port=115
  VOUTP_LatAccelVTimeOut_flg : Outport  Port=116
  VOUTP_LongAccelV_flg : Outport  Port=117
  VOUTP_LongAccelVTimeOut_flg : Outport  Port=118
  VOUTP_MCPressureV_bar : Outport  Port=119
  VOUTP_MCPressureVTimeOut_flg : Outport  Port=120
  VOUTP_BrkSwSta_flg : Outport  Port=121
  VOUTP_BrkSwStaTimeOut_flg : Outport  Port=122
  VOUTP_BrkSwV_flg : Outport  Port=123
  VOUTP_BrkSwVTimeOut_flg : Outport  Port=124
  VOUTP_ESCStandstill_flg : Outport  Port=125
  VOUTP_ESCStandstillTimeOut_flg : Outport  Port=126
  VOUTP_ESCAPSSta_enum : Outport  Port=127
  VOUTP_ESCAPSStaTimeOut_flg : Outport  Port=128
  VOUTP_EPBExtReleaseAvail_flg : Outport  Port=129
  VOUTP_EPBExtReleaseAvailTimeOut_flg : Outport  Port=130
  VOUTP_EPBExtApplyAvail_flg : Outport  Port=131
  VOUTP_EPBExtApplyAvailTimeOut_flg : Outport  Port=132
  VOUTP_EPBErrSta_enum : Outport  Port=133
  VOUTP_EPBErrStaTimeOut_flg : Outport  Port=134
  VOUTP_EPBSta_enum : Outport  Port=135
  VOUTP_EPBStaTimeOut_flg : Outport  Port=136
  VOUTP_AVMparkingcancel_enum : Outport  Port=137
  VOUTP_AVMparkingcancelTimeOut_flg : Outport  Port=138
  VOUTP_AVMparkingexcute_enum : Outport  Port=139
  VOUTP_AVMparkingexcuteTimeOut_flg : Outport  Port=140
  VOUTP_AVMParkingmode_enum : Outport  Port=141
  VOUTP_AVMParkingmodeTimeOut_flg : Outport  Port=142
  VOUTP_AVMErrSTA_flg : Outport  Port=143
  VOUTP_AVMErrSTATimeOut_flg : Outport  Port=144
  VOUTP_IVIStatus_flg : Outport  Port=145
  VOUTP_IVIStatusTimeOut_flg : Outport  Port=146
  VOUTP_CAASSw_enum : Outport  Port=147
  VOUTP_CAASSwTimeOut_flg : Outport  Port=148
  VOUTP_IVIScreen_enum : Outport  Port=149
  VOUTP_IVIScreenTimeOut_flg : Outport  Port=150
  VOUTP_ABSActive_flg : Outport  Port=151
  VOUTP_ABSActiveTimeOut_flg : Outport  Port=152
  VOUTP_TCSActive_flg : Outport  Port=153
  VOUTP_TCSActiveTimeOut_flg : Outport  Port=154
  VOUTP_DriverSeatBeltCmd_flg : Outport  Port=155
  VOUTP_DriverSeatBeltCmdTimeOut_flg : Outport  Port=156
  VOUTP_APSProgressPCT_pct : Outport  Port=157
  VOUTP_APSRQDisplay_enum : Outport  Port=158
  VOUTP_APSSWVer_enum : Outport  Port=159
  VOUTP_APSHWVer_enum : Outport  Port=160
  VOUTP_APSExitCondition_enum : Outport  Port=161
  VOUTP_APSAngleTarget_Deg : Outport  Port=162
  VOUTP_APSVRqEPASCtrl_flg : Outport  Port=163
  VOUTP_APSRqEPASCtrl_flg : Outport  Port=164
  VOUTP_CAASSta_enum : Outport  Port=165
  VOUTP_DKCPDkeyAreaRAPSSta_enum : Outport  Port=166
  VOUTP_DKCParkingModeCmd_enum : Outport  Port=167
  VOUTP_PUIDLowPower_flg : Outport  Port=168
  VOUTP_CAASVMCReqA_flg : Outport  Port=169
  VOUTP_APSShiftPosnReq_enum : Outport  Port=170
  VOUTP_APSSpeedCMD_kph : Outport  Port=171
  VOUTP_APSVMCReqA_flg : Outport  Port=172
  VOUTP_RAPSBCMLamp_enum : Outport  Port=173
  VOUTP_RAPSBCMLockReq_flg : Outport  Port=174
  VOUTP_APSPwrReq_enum : Outport  Port=175
  VOUTP_RAPSErrWarnSta_enum : Outport  Port=176
  VOUTP_RAPSErrLv1_flg : Outport  Port=177
  VOUTP_IVIUserTakeOverAPSSta_flg : Outport  Port=178
  VOUTP_AntitheftSta_enum : Outport  Port=179
  VOUTP_TailgateRemote_enum : Outport  Port=180
  VOUTP_HornCtrl_flg : Outport  Port=181
  VOUTP_AllDoorSW_flg : Outport  Port=182
  VOUTP_BCMDoorLockSta_flg : Outport  Port=183
  VOUTP_AntitheftSeatFlod_flg : Outport  Port=184
  VOUTP_HoodSW_flg : Outport  Port=185
  VOUTP_TailgateSW_flg : Outport  Port=186
  VOUTP_DrDoorSW_flg : Outport  Port=187
  VOUTP_PsDoorSW_flg : Outport  Port=188
  VOUTP_RLDoorSW_flg : Outport  Port=189
  VOUTP_RRDoorSW_flg : Outport  Port=190
  VOUTP_LockSetting_flg : Outport  Port=191
  VOUTP_FrChargingDoorCtrl_enum : Outport  Port=192
  VOUTP_RrChargingDoorCtrl_enum : Outport  Port=193
  VOUTP_CrashDetd_flg : Outport  Port=194
  VOUTP_CTDCtrl_enum : Outport  Port=195
  VOUTP_DoorLockIND_flg : Outport  Port=196
  VOUTP_CTDLockSW_flg : Outport  Port=197
  VOUTP_Dimmer_pct : Outport  Port=198
  VOUTP_DimmerEN_flg : Outport  Port=199
  VOUTP_PosLamp_flg : Outport  Port=200
  VOUTP_LBeam_flg : Outport  Port=201
  VOUTP_HBeam_flg : Outport  Port=202
  VOUTP_RrFogLamp_flg : Outport  Port=203
  VOUTP_BrakeLamp_flg : Outport  Port=204
  VOUTP_ReverseLamp_flg : Outport  Port=205
  VOUTP_LDRL_flg : Outport  Port=206
  VOUTP_RDRL_flg : Outport  Port=207
  VOUTP_LBSD_flg : Outport  Port=208
  VOUTP_RBSD_flg : Outport  Port=209
  VOUTP_HazardSW_flg : Outport  Port=210
  VOUTP_LTurnLP_flg : Outport  Port=211
  VOUTP_RTurnLP_flg : Outport  Port=212
  VOUTP_BCMBuzzerReq_flg : Outport  Port=213
  VOUTP_MirrorCtrl_enum : Outport  Port=214
  VOUTP_MirrorDefog_flg : Outport  Port=215
  VOUTP_RrDefog_flg : Outport  Port=216
  VOUTP_RoomLampH_flg : Outport  Port=217
  VOUTP_RoomLampL_flg : Outport  Port=218
  VOUTP_TrunkRel_flg : Outport  Port=219
  VOUTP_TailgateHDSW_flg : Outport  Port=220
  VOUTP_FrWiperL_flg : Outport  Port=221
  VOUTP_FrWiperH_flg : Outport  Port=222
  VOUTP_RrWiper_flg : Outport  Port=223
  VOUTP_WasherCtrl_enum : Outport  Port=224
  VOUTP_WiperFixMode_flg : Outport  Port=225
  VOUTP_AmbLightBreath1_enum : Outport  Port=226
  VOUTP_AmbLightBreath2_enum : Outport  Port=227
  VOUTP_AmbLightBreath3_enum : Outport  Port=228
  VOUTP_AmbLightBreath4_enum : Outport  Port=229
  VOUTP_AmbLightBreath5_enum : Outport  Port=230
  VOUTP_AmbLightBreath6_enum : Outport  Port=231
  VOUTP_AmbLightBrightness1_enum : Outport  Port=232
  VOUTP_AmbLightBrightness2_enum : Outport  Port=233
  VOUTP_AmbLightBrightness3_enum : Outport  Port=234
  VOUTP_AmbLightBrightness4_enum : Outport  Port=235
  VOUTP_AmbLightBrightness5_enum : Outport  Port=236
  VOUTP_AmbLightBrightness6_enum : Outport  Port=237
  VOUTP_AmbLightColor1_enum : Outport  Port=238
  VOUTP_AmbLightColor2_enum : Outport  Port=239
  VOUTP_AmbLightColor3_enum : Outport  Port=240
  VOUTP_AmbLightColor4_enum : Outport  Port=241
  VOUTP_AmbLightColor5_enum : Outport  Port=242
  VOUTP_AmbLightColor6_enum : Outport  Port=243
  VOUTP_LampPwr_flg : Outport  Port=244
  VOUTP_SPTGDet_flg : Outport  Port=245
  VOUTP_APSOpenPTG_flg : Outport  Port=246
  VOUTP_FollowMe_flg : Outport  Port=247
  VOUTP_IVIRST_flg : Outport  Port=248
  VOUTP_CountAlarm_enum : Outport  Port=249
  VOUTP_MFSWTri_flg : Outport  Port=250
  VOUTP_MirrorFlodPos_flg : Outport  Port=251
  VOUTP_FuelDoorPos_flg : Outport  Port=252
  VOUTP_MFRDNBrightReq_pct : Outport  Port=253
  VOUTP_PTGInnerSW2_enum : Outport  Port=254
  VOUTP_DrvWdwCtrlCmd_pct : Outport  Port=255
  VOUTP_PasWdwCtrlCmd_pct : Outport  Port=256
  VOUTP_DrRWdwCtrlCmd_pct : Outport  Port=257
  VOUTP_PsRWdwCtrlCmd_pct : Outport  Port=258
  VOUTP_APMDoorControlSta_flg : Outport  Port=259
  VOUTP_AmbFunEN_flg : Outport  Port=260
  VOUTP_AmbWelEN_flg : Outport  Port=261
  VOUTP_AmbDimEN_flg : Outport  Port=262
  VOUTP_AmbLinkDriSta_flg : Outport  Port=263
  VOUTP_AmbPwrWarnEN_flg : Outport  Port=264
  VOUTP_AmbODAEN_flg : Outport  Port=265
  VOUTP_AmbColorSta_enum : Outport  Port=266
  VOUTP_AmbBrightSta_enum : Outport  Port=267
  VOUTP_LockAlarm_enum : Outport  Port=268
  VOUTP_ATCtrl_enum : Outport  Port=269
  VOUTP_fUnlockSingle_flg : Outport  Port=270
  VOUTP_UserNow_enum : Outport  Port=271
  VOUTP_AmbFunENFlash_enum : Outport  Port=272
  VOUTP_AmbWelENFlash_enum : Outport  Port=273
  VOUTP_AmbDimENFlash_enum : Outport  Port=274
  VOUTP_AmbLinkDriStaFlash_enum : Outport  Port=275
  VOUTP_AmbPwrWarnENFlash_enum : Outport  Port=276
  VOUTP_AmbODAENFlash_enum : Outport  Port=277
  VOUTP_AmbColorSta1_enum : Outport  Port=278
  VOUTP_AmbColorSta2_enum : Outport  Port=279
  VOUTP_AmbColorSta3_enum : Outport  Port=280
  VOUTP_AmbColorSta4_enum : Outport  Port=281
  VOUTP_AmbColorSta5_enum : Outport  Port=282
  VOUTP_AmbColorSta7_enum : Outport  Port=283
  VOUTP_AmbBrightnessSta1_enum : Outport  Port=284
  VOUTP_AmbBrightnessSta2_enum : Outport  Port=285
  VOUTP_AmbBrightnessSta3_enum : Outport  Port=286
  VOUTP_AmbBrightnessSta4_enum : Outport  Port=287
  VOUTP_AmbBrightnessSta5_enum : Outport  Port=288
  VOUTP_AmbBrightnessSta7_enum : Outport  Port=289
  VOUTP_HazardIND_flg : Outport  Port=290
  VOUTP_DimSwSta_flg : Outport  Port=291
  VOUTP_PassSWSta_flg : Outport  Port=292
  VOUTP_FWipSwSta_enum : Outport  Port=293
  VOUTP_FWasSwSta_enum : Outport  Port=294
  VOUTP_TurnSwSta_enum : Outport  Port=295
  VOUTP_TurnSwTSetSta_enum : Outport  Port=296
  VOUTP_SPTGENFun_flg : Outport  Port=297
  VOUTP_SPTGENFunMem_enum : Outport  Port=298
  VOUTP_OutMode_enum : Outport  Port=299
  VOUTP_TurnSwTimeSetSta123_enum : Outport  Port=300
  VOUTP_TurnSwTimeSetSta457_enum : Outport  Port=301
  VOUTP_FDLHandleLampCmd_flg : Outport  Port=302
  VOUTP_FDRHandleLampCmd_flg : Outport  Port=303
  VOUTP_FDHandleCmd_enum : Outport  Port=304
  VOUTP_HBeamADB_flg : Outport  Port=305
  VOUTP_WalkInUnLkENMem_enum : Outport  Port=306
  VOUTP_WalkOutLkENMem_enum : Outport  Port=307
  VOUTP_RmLpModeENMem_enum : Outport  Port=308
  VOUTP_LockSettingStaMem_enum : Outport  Port=309
  VOUTP_FollowMeENMem_enum : Outport  Port=310
  VOUTP_WalkInUnLkENFunSta_flg : Outport  Port=311
  VOUTP_WalkOutLkENFunSta_flg : Outport  Port=312
  VOUTP_RmLpModeENFunSta_flg : Outport  Port=313
  VOUTP_FollowMeENFunSta_flg : Outport  Port=314
  VOUTP_HoodRelCmd_flg : Outport  Port=315
  VOUTP_WelcomeLight_enum : Outport  Port=316
  VOUTP_PTGOpenHeightSta_enum : Outport  Port=317
  VOUTP_UserHeightSet_cnt : Outport  Port=318
  VOUTP_PTGUserHeight1_cnt : Outport  Port=319
  VOUTP_PTGUserHeight2_cnt : Outport  Port=320
  VOUTP_PTGUserHeight3_cnt : Outport  Port=321
  VOUTP_PTGUserHeight4_cnt : Outport  Port=322
  VOUTP_PTGUserHeight5_cnt : Outport  Port=323
  VOUTP_PTGUserHeight7_cnt : Outport  Port=324
  VOUTP_PTGOpenHeight12_enum : Outport  Port=325
  VOUTP_PTGOpenHeight34_enum : Outport  Port=326
  VOUTP_PTGOpenHeight57_enum : Outport  Port=327
  VOUTP_SenstivityPosnCmd_enum : Outport  Port=328
  VOUTP_TimeGapLevelSta_enum : Outport  Port=329
  VOUTP_ACCLevelMem12_enum : Outport  Port=330
  VOUTP_ACCLevelMem34_enum : Outport  Port=331
  VOUTP_ACCLevelMem57_enum : Outport  Port=332
  VOUTP_LRightStaCmd_flg : Outport  Port=333
  VOUTP_LLeftStaCmd_flg : Outport  Port=334
  VOUTP_AutoLockSta_flg : Outport  Port=335
  VOUTP_AutoLockMem_enum : Outport  Port=336
  VOUTP_AutoUnlockSta_flg : Outport  Port=337
  VOUTP_AutoUnlockMem_enum : Outport  Port=338
  VOUTP_HMIKey1FuncSta_enum : Outport  Port=339
  VOUTP_HMIKey2FuncSta_enum : Outport  Port=340
  VOUTP_HMIKey3FuncSta_enum : Outport  Port=341
  VOUTP_HMIKey4FuncSta_enum : Outport  Port=342
  VOUTP_HMIKey5FuncSta_enum : Outport  Port=343
  VOUTP_HMIKey6FuncSta_enum : Outport  Port=344
  VOUTP_HMIKey7FuncSta_enum : Outport  Port=345
  VOUTP_HMIKey8FuncSta_enum : Outport  Port=346
  VOUTP_AutoWipHSpdENSta_flg : Outport  Port=347
  VOUTP_DrvWdwReqAP_enum : Outport  Port=348
  VOUTP_PasWdwReqAP_enum : Outport  Port=349
  VOUTP_DrRWdwReqAP_enum : Outport  Port=350
  VOUTP_PsRWdwReqAP_enum : Outport  Port=351
  VOUTP_CLWinLockDrSta_flg : Outport  Port=352
  VOUTP_CLWinLockDrStaMem_enum : Outport  Port=353
  VOUTP_WinLFOpenedSta_pct : Outport  Port=354
  VOUTP_WinRFOpenedSta_pct : Outport  Port=355
  VOUTP_WinLROpenedSta_pct : Outport  Port=356
  VOUTP_WinRROpenedSta_pct : Outport  Port=357
  VOUTP_C3BMS6RCDTC_raw32 : Outport  Port=358
  VOUTP_C3BMS6CSDTC_raw32 : Outport  Port=359
  VOUTP_C3BMS6LCDTC_raw32 : Outport  Port=360
  VOUTP_C3BMS1RCDTC_raw32 : Outport  Port=361
  VOUTP_C3BMS1CSDTC_raw32 : Outport  Port=362
  VOUTP_C3BMS1LCDTC_raw32 : Outport  Port=363
  VOUTP_C3CCU1RCDTC_raw32 : Outport  Port=364
  VOUTP_C3CCU1CSDTC_raw32 : Outport  Port=365
  VOUTP_C3CCU1LCDTC_raw32 : Outport  Port=366
  VOUTP_C3CCU2RCDTC_raw32 : Outport  Port=367
  VOUTP_C3CCU2CSDTC_raw32 : Outport  Port=368
  VOUTP_C3CCU2LCDTC_raw32 : Outport  Port=369
  VOUTP_C1ABM1RCDTC_raw32 : Outport  Port=370
  VOUTP_C1ABM1CSDTC_raw32 : Outport  Port=371
  VOUTP_C1ABM1LCDTC_raw32 : Outport  Port=372
  VOUTP_Lv1ErrDTC_raw32 : Outport  Port=373
  VOUTP_Lv2ErrDTC_raw32 : Outport  Port=374
  VOUTP_Lv3ErrDTC_raw32 : Outport  Port=375
  VOUTP_Lv4ErrDTC_raw32 : Outport  Port=376
  VOUTP_BrkSWErrDTC_raw32 : Outport  Port=377
  VOUTP_BrkSWNoBacDTC_raw32 : Outport  Port=378
  VOUTP_KeyAuthDTC_raw32 : Outport  Port=379
  VOUTP_ONtoRdyDTC_raw32 : Outport  Port=380
  VOUTP_HVB4PreDTC_raw32 : Outport  Port=381
  VOUTP_MCU4PreDTC_raw32 : Outport  Port=382
  VOUTP_DCDC4PreDTC_raw32 : Outport  Port=383
  VOUTP_HVRlyCloDTC_raw32 : Outport  Port=384
  VOUTP_BMSRdyDTC_raw32 : Outport  Port=385
  VOUTP_DCDCEnaDTC_raw32 : Outport  Port=386
  VOUTP_HiLvSaChkDTC_raw32 : Outport  Port=387
  VOUTP_MidLvSaChkDTC_raw32 : Outport  Port=388
  VOUTP_MCUDisDTC_raw32 : Outport  Port=389
  VOUTP_DCDCDisDTC_raw32 : Outport  Port=390
  VOUTP_HVRlyOpDTC_raw32 : Outport  Port=391
  VOUTP_MCUActDTC_raw32 : Outport  Port=392
  VOUTP_OBC4PreDTC_raw32 : Outport  Port=393
  VOUTP_IniLVLoDTC_raw32 : Outport  Port=394
  VOUTP_LVSupLoDTC_raw32 : Outport  Port=395
  VOUTP_LVSupHiDTC_raw32 : Outport  Port=396
  VOUTP_DrStSWDTC_raw32 : Outport  Port=397
  VOUTP_FLDoorSWDTC_raw32 : Outport  Port=398
  VOUTP_RLDoorSWDTC_raw32 : Outport  Port=399
  VOUTP_FRDoorSWDTC_raw32 : Outport  Port=400
  VOUTP_RRDoorSWDTC_raw32 : Outport  Port=401
  VOUTP_HoodSWDTC_raw32 : Outport  Port=402
  VOUTP_TailgaSWDTC_raw32 : Outport  Port=403
  VOUTP_EDriveSysErrVCUErr_flg : Outport  Port=404
  VOUTP_VehMalfunLevel_enum : Outport  Port=405
  VOUTP_APS1SigOoRDTC_raw32 : Outport  Port=406
  VOUTP_APS2SigOoRDTC_raw32 : Outport  Port=407
  VOUTP_APSCorrErrDTC_raw32 : Outport  Port=408
  VOUTP_MCUF1NoComDTC_raw32 : Outport  Port=409
  VOUTP_MCUR1NoComDTC_raw32 : Outport  Port=410
  VOUTP_Shifter1NoComDTC_raw32 : Outport  Port=411
  VOUTP_ESC7NoComDTC_raw32 : Outport  Port=412
  VOUTP_ESC1NoComDTC_raw32 : Outport  Port=413
  VOUTP_ESC5NoComDTC_raw32 : Outport  Port=414
  VOUTP_EnterNewOperCyc_flg : Outport  Port=415
  VOUTP_DiagHCrashDTC_raw32 : Outport  Port=416
  VOUTP_DiagFLTSDTC_raw32 : Outport  Port=417
  VOUTP_DiagFRTSDTC_raw32 : Outport  Port=418
  VOUTP_DiagRLTSDTC_raw32 : Outport  Port=419
  VOUTP_DiagRRTSDTC_raw32 : Outport  Port=420
  VOUTP_FCLUSSDTC_raw32 : Outport  Port=421
  VOUTP_FMLUSSDTC_raw32 : Outport  Port=422
  VOUTP_FMRUSSDTC_raw32 : Outport  Port=423
  VOUTP_FCRUSSDTC_raw32 : Outport  Port=424
  VOUTP_RCLUSSDTC_raw32 : Outport  Port=425
  VOUTP_RMLUSSDTC_raw32 : Outport  Port=426
  VOUTP_RMRUSSDTC_raw32 : Outport  Port=427
  VOUTP_RCRUSSDTC_raw32 : Outport  Port=428
  VOUTP_FLLUSSDTC_raw32 : Outport  Port=429
  VOUTP_FLRUSSDTC_raw32 : Outport  Port=430
  VOUTP_RLLUSSDTC_raw32 : Outport  Port=431
  VOUTP_RLRUSSDTC_raw32 : Outport  Port=432
  VOUTP_FCM2NoComDTC_raw32 : Outport  Port=433
  VOUTP_FCM2RCErrDTC_raw32 : Outport  Port=434
  VOUTP_FCM2CSErrDTC_raw32 : Outport  Port=435
  VOUTP_FCM3NoComDTC_raw32 : Outport  Port=436
  VOUTP_FCM3RCErrDTC_raw32 : Outport  Port=437
  VOUTP_FCM3CSErrDTC_raw32 : Outport  Port=438
  VOUTP_FCM4NoComDTC_raw32 : Outport  Port=439
  VOUTP_FCM4CSErrDTC_raw32 : Outport  Port=440
  VOUTP_FCM5NoComDTC_raw32 : Outport  Port=441
  VOUTP_FCM5CSErrDTC_raw32 : Outport  Port=442
  VOUTP_ZoneSCPNoComDTC_raw32 : Outport  Port=443
  VOUTP_BMSSigErrDetDTC_raw32 : Outport  Port=444
  VOUTP_FCMACCSigErrDetDTC_raw32 : Outport  Port=445
  VOUTP_FrMCUSigErrDetDTC_raw32 : Outport  Port=446
  VOUTP_RrMCUSigErrDetDTC_raw32 : Outport  Port=447
  VOUTP_CCUSigErrDetDTC_raw32 : Outport  Port=448
  VOUTP_ACCAccelCmdErrDetDTC_raw32 : Outport  Port=449
  VOUTP_ACCMalfuncDetDTC_raw32 : Outport  Port=450
  VOUTP_CCMalfuncDetDTC_raw32 : Outport  Port=451
  VOUTP_MSAMalfuncDetDTC_raw32 : Outport  Port=452
  VOUTP_ISAMalfuncDetDTC_raw32 : Outport  Port=453
  VOUTP_MCUF1RCErrDTC_raw32 : Outport  Port=454
  VOUTP_MCUR1RCErrDTC_raw32 : Outport  Port=455
  VOUTP_MCUF1CSErrDTC_raw32 : Outport  Port=456
  VOUTP_MCUR1CSErrDTC_raw32 : Outport  Port=457
  VOUTP_Shifter1RCErrDTC_raw32 : Outport  Port=458
  VOUTP_Shifter1CSErrDTC_raw32 : Outport  Port=459
  VOUTP_ESC7RCErrDTC_raw32 : Outport  Port=460
  VOUTP_ESC7CSErrDTC_raw32 : Outport  Port=461
  VOUTP_ESC1RCErrDTC_raw32 : Outport  Port=462
  VOUTP_ESC1CSErrDTC_raw32 : Outport  Port=463
  VOUTP_ESC5RCErrDTC_raw32 : Outport  Port=464
  VOUTP_ESC5CSErrDTC_raw32 : Outport  Port=465
  VOUTP_FrMCUTqErrDTC_raw32 : Outport  Port=466
  VOUTP_RrMCUTqErrDTC_raw32 : Outport  Port=467
  VOUTP_LFBatwarnDTC_raw32 : Outport  Port=468
  VOUTP_RFBatwarnDTC_raw32 : Outport  Port=469
  VOUTP_LRBatwarnDTC_raw32 : Outport  Port=470
  VOUTP_RRBatwarnDTC_raw32 : Outport  Port=471
  VOUTP_LFPressIndiDTC_raw32 : Outport  Port=472
  VOUTP_RFPressIndiDTC_raw32 : Outport  Port=473
  VOUTP_LRPressIndiDTC_raw32 : Outport  Port=474
  VOUTP_RRPressIndiDTC_raw32 : Outport  Port=475
  VOUTP_LFWheelTmpHighDTC_raw32 : Outport  Port=476
  VOUTP_RFWheelTmpHighDTC_raw32 : Outport  Port=477
  VOUTP_LRWheelTmpHighDTC_raw32 : Outport  Port=478
  VOUTP_RRWheelTmpHighDTC_raw32 : Outport  Port=479
  VOUTP_LFSensorFailDTC_raw32 : Outport  Port=480
  VOUTP_RFSensorFailDTC_raw32 : Outport  Port=481
  VOUTP_LRSensorFailDTC_raw32 : Outport  Port=482
  VOUTP_RRSensorFailDTC_raw32 : Outport  Port=483
  VOUTP_C1EPAS2LCDTC_raw32 : Outport  Port=484
  VOUTP_5vAPS1PwrErrDTC_raw32 : Outport  Port=485
  VOUTP_5vAPS2PwrErrDTC_raw32 : Outport  Port=486
  VOUTP_EPBLockTODTC_raw32 : Outport  Port=487
  VOUTP_EPBUnlockTODTC_raw32 : Outport  Port=488
  VOUTP_LimpHomeActTmp_flg : Outport  Port=489
  VOUTP_DTCDetect_enum : Outport  Port=490
  VOUTP_EngagePFail_flg : Outport  Port=491
  VOUTP_DisengagePFail_flg : Outport  Port=492
  VOUTP_VCURAPSErrLv2_flg : Outport  Port=493
  VOUTP_VCURAPSErrLv3_flg : Outport  Port=494
  VOUTP_EDriveSysErrShifterErr_flg : Outport  Port=495
  VOUTP_LVSysErrPwrOutErr_flg : Outport  Port=496
  VOUTP_HVRlyOpFail_flg : Outport  Port=497
  VOUTP_MCUActDisFail_flg : Outport  Port=498
  VOUTP_VCUBrkSWSta_enum : Outport  Port=499
  VOUTP_VCUFLDoorSta_flg : Outport  Port=500
  VOUTP_VCUFRDoorSta_flg : Outport  Port=501
  VOUTP_VCURLDoorSta_flg : Outport  Port=502
  VOUTP_VCURRDoorSta_flg : Outport  Port=503
  VOUTP_SysAllowReadySta_flg : Outport  Port=504
  VOUTP_VCUHoodSWSta_flg : Outport  Port=505
  VOUTP_VCUTailgateSWSta_flg : Outport  Port=506
  VOUTP_CAN1BusErrorDTC_raw32 : Outport  Port=507
  VOUTP_CAN2BusErrorDTC_raw32 : Outport  Port=508
  VOUTP_CAN3BusErrorDTC_raw32 : Outport  Port=509
  VOUTP_CAN4BusErrorDTC_raw32 : Outport  Port=510
  VOUTP_CAN5BusErrorDTC_raw32 : Outport  Port=511
  VOUTP_CAN6BusErrorDTC_raw32 : Outport  Port=512
  VOUTP_CAN1BusOffDTC_raw32 : Outport  Port=513
  VOUTP_CAN2BusOffDTC_raw32 : Outport  Port=514
  VOUTP_CAN3BusOffDTC_raw32 : Outport  Port=515
  VOUTP_CAN4BusOffDTC_raw32 : Outport  Port=516
  VOUTP_CAN5BusOffDTC_raw32 : Outport  Port=517
  VOUTP_CAN6BusOffDTC_raw32 : Outport  Port=518
  VOUTP_ActAPSPosn_pct : Outport  Port=519
  VOUTP_EAPS1MIN_pct : Outport  Port=520
  VOUTP_EAPS2MIN_pct : Outport  Port=521
  VOUTP_ResetPedalZeroPosStart_flg : Outport  Port=522
  VOUTP_EAPS1NRM_pct : Outport  Port=523
  VOUTP_EAPS2NRM_pct : Outport  Port=524
  VOUTP_DKCTimeSN_cnt : Outport  Port=525
  VOUTP_DKCAuthSta_enum : Outport  Port=526
  VOUTP_TimeSNDKCFbk_cnt : Outport  Port=527
  VOUTP_KeyMissSta_flg : Outport  Port=528
  VOUTP_KeyModeSta_enum : Outport  Port=529
  VOUTP_DkeyShowIVISta_enum : Outport  Port=530
  VOUTP_KeyAreaPS_enum : Outport  Port=531
  VOUTP_KeyAreaLockUnlock_enum : Outport  Port=532
  VOUTP_PCommandToBCM_enum : Outport  Port=533
  VOUTP_DKeyWelcomeSta_enum : Outport  Port=534
  VOUTP_KeyAreaPTG_enum : Outport  Port=535
  VOUTP_KeyAreaSPTGSta_enum : Outport  Port=536
  VOUTP_UIDLowPowerSta_enum : Outport  Port=537
  VOUTP_DkeyAreaRAPSSta_enum : Outport  Port=538
  VOUTP_ParkingModeCmd_enum : Outport  Port=539
  VOUTP_KeyNumSta_enum : Outport  Port=540
  VOUTP_KeyTypeSta_enum : Outport  Port=541
  VOUTP_FDCDKCAllowSleep_flg : Outport  Port=542
  VOUTP_DISCTurn_flg : Outport  Port=543
  VOUTP_DISCTargetSpd_kph : Outport  Port=544
  VOUTP_DISCSta_enum : Outport  Port=545
  VOUTP_DISCButtSta_flg : Outport  Port=546
  VOUTP_AllCANTxReq_flg : Outport  Port=547
  VOUTP_NMmTxReq_flg : Outport  Port=548
  VOUTP_Awake_enum : Outport  Port=549
  VOUTP_CSB_flg : Outport  Port=550
  VOUTP_ErrorState_enum : Outport  Port=551
  VOUTP_NodeID_enum : Outport  Port=552
  VOUTP_PNI_flg : Outport  Port=553
  VOUTP_RptMsgReq_flg : Outport  Port=554
  VOUTP_WakeUp_enum : Outport  Port=555
  VOUTP_ActiveWU_flg : Outport  Port=556
  VOUTP_SysNMmSta_enum : Outport  Port=557
  VOUTP_NetworkReq_flg : Outport  Port=558
  VOUTP_PowerUpState_enum : Outport  Port=559
  VOUTP_PowerDownState_enum : Outport  Port=560
  VOUTP_PowerUpFault_enum : Outport  Port=561
  VOUTP_PowerDownFault_enum : Outport  Port=562
  VOUTP_ActiveDischargeReq_flg : Outport  Port=563
  VOUTP_DCDCEnaReq_flg : Outport  Port=564
  VOUTP_DCDCVoltSetpoint_V : Outport  Port=565
  VOUTP_HVBatCnctReq_flg : Outport  Port=566
  VOUTP_HVSysReadyToCharge_enum : Outport  Port=567
  VOUTP_PowerSta_enum : Outport  Port=568
  VOUTP_LVPwrSta_flg : Outport  Port=569
  VOUTP_HVPwrSta_flg : Outport  Port=570
  VOUTP_SysPowerMode_enum : Outport  Port=571
  VOUTP_FrMCUEnaReq_flg : Outport  Port=572
  VOUTP_RrMCUEnaReq_flg : Outport  Port=573
  VOUTP_DrivetrainSelect_enum : Outport  Port=574
  VOUTP_DrSeatSta_enum : Outport  Port=575
  VOUTP_PwrStaSelect_enum : Outport  Port=576
  VOUTP_PwrStaConstraint_enum : Outport  Port=577
  VOUTP_TCountSta_enum : Outport  Port=578
  VOUTP_PwrUpReq_enum : Outport  Port=579
  VOUTP_PwrDownReq_enum : Outport  Port=580
  VOUTP_LowSOCWarn_enum : Outport  Port=581
  VOUTP_ReVehThdChkSta_enum : Outport  Port=582
  VOUTP_EvccAplusPwrUpReq_flg : Outport  Port=583
  VOUTP_PwrStaONTOPopReq_flg : Outport  Port=584
  VOUTP_IVIPwrStaONTOPopT_s : Outport  Port=585
  VOUTP_LVChrgHoldTtimer_s : Outport  Port=586
  VOUTP_LVBattChrgTimeCnt_s : Outport  Port=587
  VOUTP_SilentChkAllowSleep_flg : Outport  Port=588
  VOUTP_TimerAllowSleep_flg : Outport  Port=589
  VOUTP_FDADC12VDetAvg_mV : Outport  Port=590
  VOUTP_PMMAllowECUSleep_flg : Outport  Port=591
  VOUTP_LVSilentChrgSta_enum : Outport  Port=592
  VOUTP_LVSilentChrgReq_flg : Outport  Port=593
  VOUTP_LVSilentChrgLv_enum : Outport  Port=594
  VOUTP_CtrlFrPwrStbA1P_flg : Outport  Port=595
  VOUTP_CtrlFrRC1_flg : Outport  Port=596
  VOUTP_CtrlFrBMSCCUCIR_flg : Outport  Port=597
  VOUTP_CtrlFrEDUINVERTER_flg : Outport  Port=598
  VOUTP_HWResetSta_enum : Outport  Port=599
  VOUTP_CtrlDrPwrStbA2_flg : Outport  Port=600
  VOUTP_PwrStaTOSta_enum : Outport  Port=601
  VOUTP_Sched_ChgTOSta_enum : Outport  Port=602
  VOUTP_PwrReq_OTA_enum : Outport  Port=603
  VOUTP_OTAPwrReqOFFChkSta_enum : Outport  Port=604
  VOUTP_OTAPwrReqStdChkSta_enum : Outport  Port=605
  VOUTP_PwrReqRAPSAvail_flg : Outport  Port=606
  VOUTP_HWVer1_cnt : Outport  Port=607
  VOUTP_HWVer2_cnt : Outport  Port=608
  VOUTP_HWVer3_cnt : Outport  Port=609
  VOUTP_CarModel1_cnt : Outport  Port=610
  VOUTP_CarModel2_cnt : Outport  Port=611
  VOUTP_CarModel3_cnt : Outport  Port=612
  VOUTP_ECU1_cnt : Outport  Port=613
  VOUTP_ECU2_cnt : Outport  Port=614
  VOUTP_Major1_cnt : Outport  Port=615
  VOUTP_Major2_cnt : Outport  Port=616
  VOUTP_Minor1_cnt : Outport  Port=617
  VOUTP_Minor2_cnt : Outport  Port=618
  VOUTP_Patch1_cnt : Outport  Port=619
  VOUTP_Patch2_cnt : Outport  Port=620
  VOUTP_Country1_cnt : Outport  Port=621
  VOUTP_Country2_cnt : Outport  Port=622
  VOUTP_Variation_cnt : Outport  Port=623
  VOUTP_Dash1_cnt : Outport  Port=624
  VOUTP_Change1_cnt : Outport  Port=625
  VOUTP_Change2_cnt : Outport  Port=626
  VOUTP_Dash2_cnt : Outport  Port=627
  VOUTP_SHA1_cnt : Outport  Port=628
  VOUTP_SHA2_cnt : Outport  Port=629
  VOUTP_SHA3_cnt : Outport  Port=630
  VOUTP_SHA4_cnt : Outport  Port=631
  VOUTP_SHA5_cnt : Outport  Port=632
  VOUTP_SHA6_cnt : Outport  Port=633
  VOUTP_SHA7_cnt : Outport  Port=634
  VOUTP_SHA8_cnt : Outport  Port=635
  VOUTP_NvWriteReqRisingEdge_flg : Outport  Port=636
  VOUTP_FdcSlpReqRisingEdge_flg : Outport  Port=637
  VOUTP_FdcSlpTime_sec : Outport  Port=638
  VOUTP_PmicBootReason_enum : Outport  Port=639
  VOUTP_WisrBootReason_raw32 : Outport  Port=640
  VOUTP_AcoreRebootCmdACK_flg : Outport  Port=641
  VOUTP_CurrentNmState_enum : Outport  Port=642
  VOUTP_ECUGen1_cnt : Outport  Port=643
  VOUTP_ECUGen2_cnt : Outport  Port=644
  VOUTP_PmicBootPath_raw32 : Outport  Port=645
  VOUTP_DrivingMode_cnt : Outport  Port=646
  VOUTP_ModelYear_cnt : Outport  Port=647
  VOUTP_Var4_cnt : Outport  Port=648
  VOUTP_Var5_cnt : Outport  Port=649
  VOUTP_FDCompCmd_rpm : Outport  Port=650
  VOUTP_FDSOV1Cmd_flg : Outport  Port=651
  VOUTP_FDSOV2Cmd_flg : Outport  Port=652
  VOUTP_FDSOV3Cmd_flg : Outport  Port=653
  VOUTP_FDEXV1Cmd_step : Outport  Port=654
  VOUTP_FDEXV2Cmd_step : Outport  Port=655
  VOUTP_FDSOTXVCmd_flg : Outport  Port=656
  VOUTP_FDFWVCmd_flg : Outport  Port=657
  VOUTP_FDTWVCmd_pct : Outport  Port=658
  VOUTP_FDFrWPTCHeatPwrCmd_W : Outport  Port=659
  VOUTP_CoolgFanActDuty_pct : Outport  Port=660
  VOUTP_FDAGSCmd_enum : Outport  Port=661
  VOUTP_FDEWP1Cmd_enum : Outport  Port=662
  VOUTP_FDEWP2Cmd_enum : Outport  Port=663
  VOUTP_FDEWP3Cmd_enum : Outport  Port=664
  VOUTP_FDFrLeAPTCHeatPwrCmd_W : Outport  Port=665
  VOUTP_FDFrRiAPTCHeatPwrCmd_W : Outport  Port=666
  VOUTP_FDRrAPTCHeatPwrCmd_W : Outport  Port=667
  VOUTP_FDBlowerCmd_pct : Outport  Port=668
  VOUTP_BatteryMode_enum : Outport  Port=669
  VOUTP_EDriveMode_enum : Outport  Port=670
  VOUTP_CabinMode_enum : Outport  Port=671
  VOUTP_CCUACLampSts_flg : Outport  Port=672
  VOUTP_CCUAutoLampSts_flg : Outport  Port=673
  VOUTP_CCUACMaxLampSts_flg : Outport  Port=674
  VOUTP_CCUSyncLampSts_flg : Outport  Port=675
  VOUTP_sigAirIntenZon1St_enum : Outport  Port=676
  VOUTP_sigWindDirZon1St_enum : Outport  Port=677
  VOUTP_sigRecircSt_flg : Outport  Port=678
  VOUTP_sigSetTempZon1St_C : Outport  Port=679
  VOUTP_sigSetTempZon2St_C : Outport  Port=680
  VOUTP_sigClntTHvBattOut_C : Outport  Port=681
  VOUTP_sigCbnSolarLeft_W : Outport  Port=682
  VOUTP_sigClntTHvBattIn_C : Outport  Port=683
  VOUTP_sigCbnSolarRight_W : Outport  Port=684
  VOUTP_sigAmbAirT_C : Outport  Port=685
  VOUTP_sigCbnAirT_C : Outport  Port=686
  VOUTP_ACSubMode_enum : Outport  Port=687
  VOUTP_FDRecyAutoCmd_enum : Outport  Port=688
  VOUTP_ACModeMem_enum : Outport  Port=689
  VOUTP_Face_flg : Outport  Port=690
  VOUTP_Foot_flg : Outport  Port=691
  VOUTP_Frost_flg : Outport  Port=692
  VOUTP_FaceM_flg : Outport  Port=693
  VOUTP_FootM_flg : Outport  Port=694
  VOUTP_CCUSyncSts_flg : Outport  Port=695
  VOUTP_RecAutoFlg_flg : Outport  Port=696
  VOUTP_AirIntenZone1M_enum : Outport  Port=697
  VOUTP_fdefog_flg : Outport  Port=698
  VOUTP_sigSetTempZon2StM_C : Outport  Port=699
  VOUTP_sigDfrstSt_flg : Outport  Port=700
  VOUTP_FDCTHCAirIntZ3Sta_enum : Outport  Port=701
  VOUTP_FDCTHCLEVentModeSta_enum : Outport  Port=702
  VOUTP_FDCTHCREVentModeSta_enum : Outport  Port=703
  VOUTP_FDCTHCLEVentZSta_enum : Outport  Port=704
  VOUTP_FDCTHCCLEVentZSta_enum : Outport  Port=705
  VOUTP_FDCTHCREVentZSta_enum : Outport  Port=706
  VOUTP_FDCTHCCREVentZSta_enum : Outport  Port=707
  VOUTP_FDCTHCLEVentYSta_enum : Outport  Port=708
  VOUTP_FDCTHCLVentENSta_flg : Outport  Port=709
  VOUTP_FDCTHCCLEVentYSta_enum : Outport  Port=710
  VOUTP_FDCTHCCLVentENSta_flg : Outport  Port=711
  VOUTP_FDCTHCREVentYSta_enum : Outport  Port=712
  VOUTP_FDCTHCRVentENSta_flg : Outport  Port=713
  VOUTP_FDCTHCCREVentYSta_enum : Outport  Port=714
  VOUTP_FDCTHCCRVentENSta_flg : Outport  Port=715
  VOUTP_FDCTHCMAPTCForceOFFSta_flg : Outport  Port=716
  VOUTP_FDCFGSAirIntSta_enum : Outport  Port=717
  VOUTP_FDCFGSChSta_enum : Outport  Port=718
  VOUTP_FDCFGSAirIntCmd_enum : Outport  Port=719
  VOUTP_FDCFGSFuncSta_enum : Outport  Port=720
  VOUTP_FDCFGSChCmd_enum : Outport  Port=721
  VOUTP_FDCFGSIONSWSta_flg : Outport  Port=722
  VOUTP_FDCFGSIONCmd_flg : Outport  Port=723
  VOUTP_FDCTHCMPreWPTCHeatSta_enum : Outport  Port=724
  VOUTP_EWPBUflag1_flg : Outport  Port=725
  VOUTP_EWPBUflag2_flg : Outport  Port=726
  VOUTP_EWPBUflag3_flg : Outport  Port=727
  VOUTP_FaceMSet_enum : Outport  Port=728
  VOUTP_FootMSet_enum : Outport  Port=729
  VOUTP_fdefogSet_enum : Outport  Port=730
  VOUTP_CCUSyncStsSet_enum : Outport  Port=731
  VOUTP_sigRecircStSet_enum : Outport  Port=732
  VOUTP_RecyAutoSet_enum : Outport  Port=733
  VOUTP_AirIntenZone1MSet1_enum : Outport  Port=734
  VOUTP_AirIntenZone1MSet2_enum : Outport  Port=735
  VOUTP_AirIntenZone1MSet3_enum : Outport  Port=736
  VOUTP_AirIntenZone1MSet4_enum : Outport  Port=737
  VOUTP_AirIntenZone1MSet5_enum : Outport  Port=738
  VOUTP_AirIntenZone1MSet7_enum : Outport  Port=739
  VOUTP_AirIntenZone3MSet1_enum : Outport  Port=740
  VOUTP_AirIntenZone3MSet2_enum : Outport  Port=741
  VOUTP_AirIntenZone3MSet3_enum : Outport  Port=742
  VOUTP_AirIntenZone3MSet4_enum : Outport  Port=743
  VOUTP_AirIntenZone3MSet5_enum : Outport  Port=744
  VOUTP_AirIntenZone3MSet7_enum : Outport  Port=745
  VOUTP_IONSWStaSet_enum : Outport  Port=746
  VOUTP_FDCFGSChStaSet123_enum : Outport  Port=747
  VOUTP_FDCFGSChStaSet457_enum : Outport  Port=748
  VOUTP_FDCFGSAirIntStaSet123_enum : Outport  Port=749
  VOUTP_FDCFGSAirIntStaSet457_enum : Outport  Port=750
  VOUTP_LVentENSet_enum : Outport  Port=751
  VOUTP_CLVentENSet_enum : Outport  Port=752
  VOUTP_RVentENSet_enum : Outport  Port=753
  VOUTP_CRVentENSet_enum : Outport  Port=754
  VOUTP_LEVentModeStaSet123_enum : Outport  Port=755
  VOUTP_LEVentModeStaSet457_enum : Outport  Port=756
  VOUTP_REVentModeStaSet123_enum : Outport  Port=757
  VOUTP_REVentModeStaSet457_enum : Outport  Port=758
  VOUTP_FDCTHCLEVentZStaSet1_enum : Outport  Port=759
  VOUTP_FDCTHCLEVentZStaSet2_enum : Outport  Port=760
  VOUTP_FDCTHCLEVentZStaSet3_enum : Outport  Port=761
  VOUTP_FDCTHCLEVentZStaSet4_enum : Outport  Port=762
  VOUTP_FDCTHCLEVentZStaSet5_enum : Outport  Port=763
  VOUTP_FDCTHCLEVentZStaSet7_enum : Outport  Port=764
  VOUTP_FDCTHCCLEVentZStaSet1_enum : Outport  Port=765
  VOUTP_FDCTHCCLEVentZStaSet2_enum : Outport  Port=766
  VOUTP_FDCTHCCLEVentZStaSet3_enum : Outport  Port=767
  VOUTP_FDCTHCCLEVentZStaSet4_enum : Outport  Port=768
  VOUTP_FDCTHCCLEVentZStaSet5_enum : Outport  Port=769
  VOUTP_FDCTHCCLEVentZStaSet7_enum : Outport  Port=770
  VOUTP_FDCTHCREVentZStaSet1_enum : Outport  Port=771
  VOUTP_FDCTHCREVentZStaSet2_enum : Outport  Port=772
  VOUTP_FDCTHCREVentZStaSet3_enum : Outport  Port=773
  VOUTP_FDCTHCREVentZStaSet4_enum : Outport  Port=774
  VOUTP_FDCTHCREVentZStaSet5_enum : Outport  Port=775
  VOUTP_FDCTHCREVentZStaSet7_enum : Outport  Port=776
  VOUTP_FDCTHCCREVentZStaSet1_enum : Outport  Port=777
  VOUTP_FDCTHCCREVentZStaSet2_enum : Outport  Port=778
  VOUTP_FDCTHCCREVentZStaSet3_enum : Outport  Port=779
  VOUTP_FDCTHCCREVentZStaSet4_enum : Outport  Port=780
  VOUTP_FDCTHCCREVentZStaSet5_enum : Outport  Port=781
  VOUTP_FDCTHCCREVentZStaSet7_enum : Outport  Port=782
  VOUTP_FDCTHCLEVentYStaSet1_enum : Outport  Port=783
  VOUTP_FDCTHCLEVentYStaSet2_enum : Outport  Port=784
  VOUTP_FDCTHCLEVentYStaSet3_enum : Outport  Port=785
  VOUTP_FDCTHCLEVentYStaSet4_enum : Outport  Port=786
  VOUTP_FDCTHCLEVentYStaSet5_enum : Outport  Port=787
  VOUTP_FDCTHCLEVentYStaSet7_enum : Outport  Port=788
  VOUTP_FDCTHCCLEVentYStaSet1_enum : Outport  Port=789
  VOUTP_FDCTHCCLEVentYStaSet2_enum : Outport  Port=790
  VOUTP_FDCTHCCLEVentYStaSet3_enum : Outport  Port=791
  VOUTP_FDCTHCCLEVentYStaSet4_enum : Outport  Port=792
  VOUTP_FDCTHCCLEVentYStaSet5_enum : Outport  Port=793
  VOUTP_FDCTHCCLEVentYStaSet7_enum : Outport  Port=794
  VOUTP_FDCTHCREVentYStaSet1_enum : Outport  Port=795
  VOUTP_FDCTHCREVentYStaSet2_enum : Outport  Port=796
  VOUTP_FDCTHCREVentYStaSet3_enum : Outport  Port=797
  VOUTP_FDCTHCREVentYStaSet4_enum : Outport  Port=798
  VOUTP_FDCTHCREVentYStaSet5_enum : Outport  Port=799
  VOUTP_FDCTHCREVentYStaSet7_enum : Outport  Port=800
  VOUTP_FDCTHCCREVentYStaSet1_enum : Outport  Port=801
  VOUTP_FDCTHCCREVentYStaSet2_enum : Outport  Port=802
  VOUTP_FDCTHCCREVentYStaSet3_enum : Outport  Port=803
  VOUTP_FDCTHCCREVentYStaSet4_enum : Outport  Port=804
  VOUTP_FDCTHCCREVentYStaSet5_enum : Outport  Port=805
  VOUTP_FDCTHCCREVentYStaSet7_enum : Outport  Port=806
  VOUTP_SettempZon1Set1_enum : Outport  Port=807
  VOUTP_SettempZon1Set2_enum : Outport  Port=808
  VOUTP_SettempZon1Set3_enum : Outport  Port=809
  VOUTP_SettempZon1Set4_enum : Outport  Port=810
  VOUTP_SettempZon1Set5_enum : Outport  Port=811
  VOUTP_SettempZon1Set7_enum : Outport  Port=812
  VOUTP_ACModeSet123_enum : Outport  Port=813
  VOUTP_ACModeSet457_enum : Outport  Port=814
  VOUTP_FACESet_enum : Outport  Port=815
  VOUTP_FOOTSet_enum : Outport  Port=816
  VOUTP_FrostSet_enum : Outport  Port=817
  VOUTP_LVentEN_flg : Outport  Port=818
  VOUTP_CLVentEN_flg : Outport  Port=819
  VOUTP_RVentEN_flg : Outport  Port=820
  VOUTP_CRVentEN_flg : Outport  Port=821
  VOUTP_FDCFGSLearnCmd_enum : Outport  Port=822
  VOUTP_FDCFGSFuncSta_flg : Outport  Port=823
  VOUTP_THSysErrlampReq_flg : Outport  Port=824
  VOUTP_sigCbnPTCPwrAct_W : Outport  Port=825
  VOUTP_LFBatWarn_flg : Outport  Port=826
  VOUTP_RFBatWarn_flg : Outport  Port=827
  VOUTP_LRBatWarn_flg : Outport  Port=828
  VOUTP_RRBatWarn_flg : Outport  Port=829
  VOUTP_LFWheelPress_raw8 : Outport  Port=830
  VOUTP_RFWheelPress_raw8 : Outport  Port=831
  VOUTP_LRWheelPress_raw8 : Outport  Port=832
  VOUTP_RRWheelPress_raw8 : Outport  Port=833
  VOUTP_LFWheelTemp_C : Outport  Port=834
  VOUTP_RFWheelTemp_C : Outport  Port=835
  VOUTP_LRWheelTemp_C : Outport  Port=836
  VOUTP_RRWheelTemp_C : Outport  Port=837
  VOUTP_LFSensorFail_flg : Outport  Port=838
  VOUTP_RFSensorFail_flg : Outport  Port=839
  VOUTP_LRSensorFail_flg : Outport  Port=840
  VOUTP_RRSensorFail_flg : Outport  Port=841
  VOUTP_LFWheelDebug_flg : Outport  Port=842
  VOUTP_LRWheelDebug_flg : Outport  Port=843
  VOUTP_RFWheelDebug_flg : Outport  Port=844
  VOUTP_RRWheelDebug_flg : Outport  Port=845
  VOUTP_TPMSResButtAllow_flg : Outport  Port=846
  VOUTP_TPMSCaliButtAllow_flg : Outport  Port=847
  VOUTP_LFPressIndi_enum : Outport  Port=848
  VOUTP_RFPressIndi_enum : Outport  Port=849
  VOUTP_LRPressIndi_enum : Outport  Port=850
  VOUTP_RRPressIndi_enum : Outport  Port=851
  VOUTP_TPMSWarnIndi_enum : Outport  Port=852
  VOUTP_LFWheelTmpIndi_flg : Outport  Port=853
  VOUTP_RFWheelTmpIndi_flg : Outport  Port=854
  VOUTP_LRWheelTmpIndi_flg : Outport  Port=855
  VOUTP_RRWheelTmpIndi_flg : Outport  Port=856
  VOUTP_LFWheelPSW_raw8 : Outport  Port=857
  VOUTP_LRWheelPSW_raw8 : Outport  Port=858
  VOUTP_RFWheelPSW_raw8 : Outport  Port=859
  VOUTP_RRWheelPSW_raw8 : Outport  Port=860
  VOUTP_CWheelTips_enum : Outport  Port=861
  VOUTP_AutoLTips_enum : Outport  Port=862
  VOUTP_LFSensorMode_flg : Outport  Port=863
  VOUTP_RFSensorMode_flg : Outport  Port=864
  VOUTP_LRSensorMode_flg : Outport  Port=865
  VOUTP_RRSensorMode_flg : Outport  Port=866
  VOUTP_S1ID_raw32 : Outport  Port=867
  VOUTP_S2ID_raw32 : Outport  Port=868
  VOUTP_S3ID_raw32 : Outport  Port=869
  VOUTP_S4ID_raw32 : Outport  Port=870
  VOUTP_S1L_enum : Outport  Port=871
  VOUTP_S2L_enum : Outport  Port=872
  VOUTP_S3L_enum : Outport  Port=873
  VOUTP_S4L_enum : Outport  Port=874
  VOUTP_ALFin_flg : Outport  Port=875
  VOUTP_LFP20_raw8 : Outport  Port=876
  VOUTP_RFP20_raw8 : Outport  Port=877
  VOUTP_LRP20_raw8 : Outport  Port=878
  VOUTP_RRP20_raw8 : Outport  Port=879
  VOUTP_FAT_flg : Outport  Port=880
  VOUTP_IDin_raw32 : Outport  Port=881
  VOUTP_S1WheelDebugALTU_pct : Outport  Port=882
  VOUTP_S2WheelDebugALTU_pct : Outport  Port=883
  VOUTP_S3WheelDebugALTU_pct : Outport  Port=884
  VOUTP_S4WheelDebugALTU_pct : Outport  Port=885
  VOUTP_ID1messageALTU_raw8 : Outport  Port=886
  VOUTP_ID2messageALTU_raw8 : Outport  Port=887
  VOUTP_ID3messageALTU_raw8 : Outport  Port=888
  VOUTP_ID4messageALTU_raw8 : Outport  Port=889
  VOUTP_Chkfin_flg : Outport  Port=890
  VOUTP_SetIDLoc_flg : Outport  Port=891
  VOUTP_TPMSStorge_flg : Outport  Port=892
  VOUTP_ChkStorge_flg : Outport  Port=893
  VOUTP_TPMSResButt_flg : Outport  Port=894
  VOUTP_LFPindi_enum : Outport  Port=895
  VOUTP_RFPind_enum : Outport  Port=896
  VOUTP_LRPindi_enum : Outport  Port=897
  VOUTP_RRPindi_enum : Outport  Port=898
  VOUTP_WriteChkLFID_raw : Outport  Port=899
  VOUTP_WriteChkRFID_raw : Outport  Port=900
  VOUTP_WriteChkLRID_raw : Outport  Port=901
  VOUTP_WriteChkRRID_raw : Outport  Port=902
  VOUTP_WriteChkfinLFID_raw : Outport  Port=903
  VOUTP_WriteChkfinRFID_raw : Outport  Port=904
  VOUTP_WriteChkfinLRID_raw : Outport  Port=905
  VOUTP_WriteChkfinRRID_raw : Outport  Port=906
  VOUTP_Flashchkdatavalid_enum : Outport  Port=907
  VOUTP_Flashdatavalid_enum : Outport  Port=908
  VOUTP_unlearnSfali_flg : Outport  Port=909
  VOUTP_unlearnSfailvalid_enum : Outport  Port=910
  VOUTP_Prepresstempvalid_enum : Outport  Port=911
  VOUTP_FlashS1ID_raw : Outport  Port=912
  VOUTP_FlashS2ID_raw : Outport  Port=913
  VOUTP_FlashS3ID_raw : Outport  Port=914
  VOUTP_FlashS4ID_raw : Outport  Port=915
  VOUTP_FlashIDvalid_enum : Outport  Port=916
  VOUTP_WritingCnt_enum : Outport  Port=917
  VOUTP_TPMSTLCmd_flg : Outport  Port=918
  VOUTP_LProgress_enum : Outport  Port=919
  VOUTP_TPMSSensorIDRegStart_flg : Outport  Port=920
  VOUTP_ModelVersion_raw : Outport  Port=921
  VOUTP_ModelVersionChksum_raw : Outport  Port=922
  VOUTP_ParkRequest_flg : Outport  Port=923
  VOUTP_TqSourceFr_enum : Outport  Port=924
  VOUTP_TqSourceRr_enum : Outport  Port=925
  VOUTP_FrEDUAvailBrkRgnTq_Nm : Outport  Port=926
  VOUTP_RrEDUAvailBrkRgnTq_Nm : Outport  Port=927
  VOUTP_EVDriveMode_enum : Outport  Port=928
  VOUTP_ShiftGearPosn_enum : Outport  Port=929
  VOUTP_PButtonSta_enum : Outport  Port=930
  VOUTP_FrActvDmpDisabReq_flg : Outport  Port=931
  VOUTP_RrActvDmpDisabReq_flg : Outport  Port=932
  VOUTP_FrRgnDecrSta_flg : Outport  Port=933
  VOUTP_RrRgnDecrSta_flg : Outport  Port=934
  VOUTP_DriverWhlTqDemFr_Nm : Outport  Port=935
  VOUTP_DriverWhlTqDemRr_Nm : Outport  Port=936
  VOUTP_FrEDUActTq_Nm : Outport  Port=937
  VOUTP_RrEDUActTq_Nm : Outport  Port=938
  VOUTP_FrEDURolRgnTq_Nm : Outport  Port=939
  VOUTP_RrEDURolRgnTq_Nm : Outport  Port=940
  VOUTP_FrEDUSpd_rpm : Outport  Port=941
  VOUTP_RrEDUSpd_rpm : Outport  Port=942
  VOUTP_FrEDUSpdValid_flg : Outport  Port=943
  VOUTP_FrEDUAvailBrkRgnTqV_flg : Outport  Port=944
  VOUTP_RrEDUSpdValid_flg : Outport  Port=945
  VOUTP_RrEDUAvailBrkRgnTqV_flg : Outport  Port=946
  VOUTP_RgnAbnorSta_flg : Outport  Port=947
  VOUTP_PTCSPermSta_flg : Outport  Port=948
  VOUTP_FrRgnPermSta_flg : Outport  Port=949
  VOUTP_RrRgnPermSta_flg : Outport  Port=950
  VOUTP_FrIdcMin_A : Outport  Port=951
  VOUTP_FrIdcMax_A : Outport  Port=952
  VOUTP_FrUdcMin_V : Outport  Port=953
  VOUTP_FrUdcMax_V : Outport  Port=954
  VOUTP_RrIdcMin_A : Outport  Port=955
  VOUTP_RrIdcMax_A : Outport  Port=956
  VOUTP_RrUdcMin_V : Outport  Port=957
  VOUTP_RrUdcMax_V : Outport  Port=958
  VOUTP_ReBrakeLPReq_flg : Outport  Port=959
  VOUTP_CreepON_flg : Outport  Port=960
  VOUTP_EquivAccPedalSWSta_flg : Outport  Port=961
  VOUTP_DriveProtEn_flg : Outport  Port=962
  VOUTP_ActParkRequest_flg : Outport  Port=963
  VOUTP_IVIPwrLockSta_enum : Outport  Port=964
  VOUTP_OPDHoldLamp_flg : Outport  Port=965
  VOUTP_SaveRegenMode_enum : Outport  Port=966
  VOUTP_FDCVCURegenMode_enum : Outport  Port=967
  VOUTP_SpdCtrlMode_enum : Outport  Port=968
  VOUTP_SpdCtrlSta_flg : Outport  Port=969
  VOUTP_SetSpd_kph : Outport  Port=970
  VOUTP_VehActSpd_kph : Outport  Port=971
  VOUTP_RegenLimIndSta_flg : Outport  Port=972
  VOUTP_SetSpdLimWarn_flg : Outport  Port=973
  VOUTP_FrTMTqReq_Nm : Outport  Port=974
  VOUTP_RrTMTqReq_Nm : Outport  Port=975
  VOUTP_ReqOBCV2LEna_enum : Outport  Port=976
  VOUTP_ReqV2LIVIPopup_enum : Outport  Port=977
  VOUTP_ReqV2LIVIDisChrg_enum : Outport  Port=978
  VOUTP_ReqOBCExtrV2LEna_enum : Outport  Port=979
  VOUTP_ReqOBCIntrV2LEna_enum : Outport  Port=980
  VOUTP_HVPO120VGrpALDSt_enum : Outport  Port=981
  VOUTP_HVPO120VGrpBLDSt_enum : Outport  Port=982
  VOUTP_FeatSetSpdFinal_raw32 : Outport  Port=983
  VOUTP_VehicleSpeed_mph : Outport  Port=984
  VOUTP_VehicleSpeed_kph : Outport  Port=985
  VOUTP_MeterIndSpeed_raw32 : Outport  Port=986
  VOUTP_VMCAEBCtrlAvail_flg : Outport  Port=987
  VOUTP_VMCACCCtrlAvail_flg : Outport  Port=988
  VOUTP_VMCCCCtrlAvail_flg : Outport  Port=989
  VOUTP_VMCMSACtrlAvail_flg : Outport  Port=990
  VOUTP_FeatArbitrSta_enum : Outport  Port=991
  VOUTP_FeatReqSpd_kph : Outport  Port=992
  VOUTP_JerkPCT_pct : Outport  Port=993
  VOUTP_LimitPCT_pct : Outport  Port=994
  VOUTP_FrontRearSlipRatioCtrl_flg : Outport  Port=995
  VOUTP_RearWhlSlipRatioCtrl_flg : Outport  Port=996
  VOUTP_SingleWhlSlipRatioCtrl_flg : Outport  Port=997
  VOUTP_LatAccCtrl_flg : Outport  Port=998
  VOUTP_SafetyCtrl_flg : Outport  Port=999
  VOUTP_SPD2ACCAct_flg : Outport  Port=1000
  VOUTP_AccCalcuPID_mps2 : Outport  Port=1001
  VOUTP_ISOAccLimit_mps2 : Outport  Port=1002
  VOUTP_ISODecLimit_mps2 : Outport  Port=1003
  VOUTP_ISOJerkLimit_mps3 : Outport  Port=1004
  VOUTP_ACCRequiredAccel_mps2 : Outport  Port=1005
  VOUTP_DISCReqAcc_mps2 : Outport  Port=1006
  VOUTP_FeatArbitrFinal_enum : Outport  Port=1007
  VOUTP_ActACCRequiredAccel_mps2 : Outport  Port=1008
  VOUTP_LateralCtrl_flg : Outport  Port=1009
  VOUTP_ADASLKASta_enum : Outport  Port=1010
  VOUTP_LKAStrToqReq_Nm : Outport  Port=1011
  VOUTP_LKATOIFault_flg : Outport  Port=1012
  VOUTP_LKATOIAct_enum : Outport  Port=1013
  VOUTP_ADASAEBReq_enum : Outport  Port=1014
  VOUTP_ADASFaultSta_flg : Outport  Port=1015
  VOUTP_AEBVehHoldReq_flg : Outport  Port=1016
  VOUTP_ACCVehHoldReq_flg : Outport  Port=1017
  VOUTP_ADASDBSReq_enum : Outport  Port=1018
  VOUTP_ADASACCSta_enum : Outport  Port=1019
  VOUTP_ACCObjDist_m : Outport  Port=1020
  VOUTP_ACCObjRelSpd_mps : Outport  Port=1021
  VOUTP_TimeGapLevel_enum : Outport  Port=1022
  VOUTP_ACCJerkUpperLimit_mps3 : Outport  Port=1023
  VOUTP_ACCComfortBandUpper_mps2 : Outport  Port=1024
  VOUTP_ACCJerkLowerLimit_mps3 : Outport  Port=1025
  VOUTP_ACCComfortBandLower_mps2 : Outport  Port=1026
  VOUTP_ADASVehSpdLim_raw32 : Outport  Port=1027
  VOUTP_ADASShftPosnReqA_flg : Outport  Port=1028
  VOUTP_ADASShftPosnReq_enum : Outport  Port=1029
  VOUTP_ADASForceIdle_flg : Outport  Port=1030
  VOUTP_HazardWarningReq_flg : Outport  Port=1031
  VOUTP_RightTurnLightReq_flg : Outport  Port=1032
  VOUTP_LeftTurnLightReq_flg : Outport  Port=1033
  VOUTP_ADASFCWSta_enum : Outport  Port=1034
  VOUTP_ADASLDWSta_enum : Outport  Port=1035
  VOUTP_ADASFltWrnReq_flg : Outport  Port=1036
  VOUTP_ACCObjDstLvl_enum : Outport  Port=1037
  VOUTP_ForceLowBeam_enum : Outport  Port=1038
  VOUTP_ACCTakeoverReq_flg : Outport  Port=1039
  VOUTP_ADASWarningMsg_enum : Outport  Port=1040
  VOUTP_ADASCAMSpdLim_enum : Outport  Port=1041
  VOUTP_TargetType_enum : Outport  Port=1042
  VOUTP_ADASSLIFSpdLim_enum : Outport  Port=1043
  VOUTP_LKAHODDisplayWarning_flg : Outport  Port=1044
  VOUTP_LKAHODSoundWarning_flg : Outport  Port=1045
  VOUTP_ADASLFCSta_enum : Outport  Port=1046
  VOUTP_ADASLaneModeL_enum : Outport  Port=1047
  VOUTP_ADASLaneModeR_enum : Outport  Port=1048
  VOUTP_ADASSLIFSta_enum : Outport  Port=1049
  VOUTP_ADASISASta_enum : Outport  Port=1050
  VOUTP_ADASLDWMute_flg : Outport  Port=1051
  VOUTP_ADASFCWMute_flg : Outport  Port=1052
  VOUTP_ADASLFCHandsOffWarning_enum : Outport  Port=1053
  VOUTP_LVDADisabled_flg : Outport  Port=1054
  VOUTP_LVDAMuteSta_enum : Outport  Port=1055
  VOUTP_LVDAFailinfo_flg : Outport  Port=1056
  VOUTP_LVDAWarning_flg : Outport  Port=1057
  VOUTP_LVDAACCStatusInformation_flg : Outport  Port=1058
  VOUTP_ADASLFCWarnSound_enum : Outport  Port=1059
  VOUTP_FCMACCmode_enum : Outport  Port=1060
  VOUTP_ADASLanetypeR_enum : Outport  Port=1061
  VOUTP_ADASLanetypeL_enum : Outport  Port=1062
  VOUTP_ADASLanecurveL_raw32 : Outport  Port=1063
  VOUTP_ADASLanecurveR_raw32 : Outport  Port=1064
  VOUTP_ADASAEBSta_enum : Outport  Port=1065
  VOUTP_FCMLDWRequest_enum : Outport  Port=1066
  VOUTP_FCMLDWFault_flg : Outport  Port=1067
  VOUTP_ACCCtrlAvail_flg : Outport  Port=1068
  VOUTP_ACCPedalOvrd_flg : Outport  Port=1069
  VOUTP_TimeGapCalcu_s : Outport  Port=1070
  VOUTP_CCCtrlSta_enum : Outport  Port=1071
  VOUTP_MSACtrlSta_enum : Outport  Port=1072
  VOUTP_APSCtrlAvail_flg : Outport  Port=1073
  VOUTP_APSActive_flg : Outport  Port=1074
  VOUTP_APSStaSys_enum : Outport  Port=1075
  VOUTP_APSDecReqA_flg : Outport  Port=1076
  VOUTP_APSDecReq_mps2 : Outport  Port=1077
  VOUTP_APSReq_enum : Outport  Port=1078
  VOUTP_LongAcc_Gps : Outport  Port=1079
  VOUTP_CCMSASpdWar_flg : Outport  Port=1080
  VOUTP_IMUEnaCmd_flg : Outport  Port=1081
  VOUTP_CAASCtrlAvail_flg : Outport  Port=1082
  VOUTP_CAASActive_flg : Outport  Port=1083
  VOUTP_ExtraMSACtrlSta_enum : Outport  Port=1084
  VOUTP_CalibratedAccX_G : Outport  Port=1085
  VOUTP_CalibratedAccY_G : Outport  Port=1086
  VOUTP_CalibratedAccZ_G : Outport  Port=1087
  VOUTP_CalibratedGyroX_Dps : Outport  Port=1088
  VOUTP_CalibratedGyroY_Dps : Outport  Port=1089
  VOUTP_CalibratedGyroZ_Dps : Outport  Port=1090
  VOUTP_FDCVMCAPSVRqEPSCtrl_flg : Outport  Port=1091
  VOUTP_FDCVMCAPSAngleTarget_deg : Outport  Port=1092
  VOUTP_FDCVMCAPSRqEPSCtrl_flg : Outport  Port=1093
  VOUTP_FDCVMCAngCtrlTqWtGn_pct : Outport  Port=1094
  VOUTP_FDCVMCDrInpTqBstAct_flg : Outport  Port=1095
  VOUTP_FDCVMCMaxAngCtrlOutTqLim_Nm : Outport  Port=1096
  VOUTP_FDCVMCDrInpTqBstGn_pct : Outport  Port=1097
  wires:
  VACC_HVTHCMSysAvail_enum/1 -> VACC_HVTHCMSysAvail_enum_Inproc/1  "VACC_HVTHCMSysAvail_enum"
  VACC_HVTHCMSysAvail_enum_Inproc/1 -> UnitConverter1/1
  UnitConverter1/1 -> VOUTP_HVTHCMSysAvail_enum/1  "VOUTP_HVTHCMSysAvail_enum"
  VACC_LVBattVoltSta_enum/1 -> VACC_LVBattVoltSta_enum_Inproc/1  "VACC_LVBattVoltSta_enum"
  VACC_LVBattVoltSta_enum_Inproc/1 -> UnitConverter2/1
  UnitConverter2/1 -> VOUTP_LVBattVoltSta_enum/1  "VOUTP_LVBattVoltSta_enum"
  VACC_VehHVPwrAvail4THCM_W/1 -> VACC_VehHVPwrAvail4THCM_W_Inproc/1  "VACC_VehHVPwrAvail4THCM_W"
  VACC_VehHVPwrAvail4THCM_W_Inproc/1 -> UnitConverter3/1
  UnitConverter3/1 -> VOUTP_VehHVPwrAvail4THCM_W/1  "VOUTP_VehHVPwrAvail4THCM_W"
  VAPM_VehSpeed_kph/1 -> VAPM_VehSpeed_kph_Inproc/1  "VAPM_VehSpeed_kph"
  VAPM_VehSpeed_kph_Inproc/1 -> UnitConverter4/1
  UnitConverter4/1 -> VOUTP_VehSpeed_kph/1  "VOUTP_VehSpeed_kph"
  VAPM_VehSpeedTimeOut_flg/1 -> VAPM_VehSpeedTimeOut_flg_Inproc/1  "VAPM_VehSpeedTimeOut_flg"
  VAPM_VehSpeedTimeOut_flg_Inproc/1 -> UnitConverter5/1
  UnitConverter5/1 -> VOUTP_VehSpeedTimeOut_flg/1  "VOUTP_VehSpeedTimeOut_flg"
  VAPM_FSOffSw_enum/1 -> VAPM_FSOffSw_enum_Inproc/1  "VAPM_FSOffSw_enum"
  VAPM_FSOffSw_enum_Inproc/1 -> UnitConverter6/1
  UnitConverter6/1 -> VOUTP_FSOffSw_enum/1  "VOUTP_FSOffSw_enum"
  VAPM_FSOffSwTimeOut_flg/1 -> VAPM_FSOffSwTimeOut_flg_Inproc/1  "VAPM_FSOffSwTimeOut_flg"
  VAPM_FSOffSwTimeOut_flg_Inproc/1 -> UnitConverter7/1
  UnitConverter7/1 -> VOUTP_FSOffSwTimeOut_flg/1  "VOUTP_FSOffSwTimeOut_flg"
  VAPM_ChrgPlugSta_enum/1 -> VAPM_ChrgPlugSta_enum_Inproc/1  "VAPM_ChrgPlugSta_enum"
  VAPM_ChrgPlugSta_enum_Inproc/1 -> UnitConverter8/1
  UnitConverter8/1 -> VOUTP_ChrgPlugSta_enum/1  "VOUTP_ChrgPlugSta_enum"
  VAPM_PASDRMR_cm/1 -> VAPM_PASDRMR_cm_Inproc/1  "VAPM_PASDRMR_cm"
  VAPM_PASDRMR_cm_Inproc/1 -> UnitConverter9/1
  UnitConverter9/1 -> VOUTP_PASDRMR_cm/1  "VOUTP_PASDRMR_cm"
  VAPM_PASDRML_cm/1 -> VAPM_PASDRML_cm_Inproc/1  "VAPM_PASDRML_cm"
  VAPM_PASDRML_cm_Inproc/1 -> UnitConverter10/1
  UnitConverter10/1 -> VOUTP_PASDRML_cm/1  "VOUTP_PASDRML_cm"
  VAPM_PASDRCR_cm/1 -> VAPM_PASDRCR_cm_Inproc/1  "VAPM_PASDRCR_cm"
  VAPM_PASDRCR_cm_Inproc/1 -> UnitConverter11/1
  UnitConverter11/1 -> VOUTP_PASDRCR_cm/1  "VOUTP_PASDRCR_cm"
  VAPM_PASDRCL_cm/1 -> VAPM_PASDRCL_cm_Inproc/1  "VAPM_PASDRCL_cm"
  VAPM_PASDRCL_cm_Inproc/1 -> UnitConverter12/1
  UnitConverter12/1 -> VOUTP_PASDRCL_cm/1  "VOUTP_PASDRCL_cm"
  VAPM_PASDFMR_cm/1 -> VAPM_PASDFMR_cm_Inproc/1  "VAPM_PASDFMR_cm"
  VAPM_PASDFMR_cm_Inproc/1 -> UnitConverter13/1
  UnitConverter13/1 -> VOUTP_PASDFMR_cm/1  "VOUTP_PASDFMR_cm"
  VAPM_PASDFML_cm/1 -> VAPM_PASDFML_cm_Inproc/1  "VAPM_PASDFML_cm"
  VAPM_PASDFML_cm_Inproc/1 -> UnitConverter14/1
  UnitConverter14/1 -> VOUTP_PASDFML_cm/1  "VOUTP_PASDFML_cm"
  VAPM_PASDFCR_cm/1 -> VAPM_PASDFCR_cm_Inproc/1  "VAPM_PASDFCR_cm"
  VAPM_PASDFCR_cm_Inproc/1 -> UnitConverter15/1
  UnitConverter15/1 -> VOUTP_PASDFCR_cm/1  "VOUTP_PASDFCR_cm"
  VAPM_PASDFCL_cm/1 -> VAPM_PASDFCL_cm_Inproc/1  "VAPM_PASDFCL_cm"
  VAPM_PASDFCL_cm_Inproc/1 -> UnitConverter16/1
  UnitConverter16/1 -> VOUTP_PASDFCL_cm/1  "VOUTP_PASDFCL_cm"
  VAPM_APSDRLR_cm/1 -> VAPM_APSDRLR_cm_Inproc/1  "VAPM_APSDRLR_cm"
  VAPM_APSDRLR_cm_Inproc/1 -> UnitConverter17/1
  UnitConverter17/1 -> VOUTP_APSDRLR_cm/1  "VOUTP_APSDRLR_cm"
  VAPM_APSDRLL_cm/1 -> VAPM_APSDRLL_cm_Inproc/1  "VAPM_APSDRLL_cm"
  VAPM_APSDRLL_cm_Inproc/1 -> UnitConverter18/1
  UnitConverter18/1 -> VOUTP_APSDRLL_cm/1  "VOUTP_APSDRLL_cm"
  VAPM_APSDFLR_cm/1 -> VAPM_APSDFLR_cm_Inproc/1  "VAPM_APSDFLR_cm"
  VAPM_APSDFLR_cm_Inproc/1 -> UnitConverter19/1
  UnitConverter19/1 -> VOUTP_APSDFLR_cm/1  "VOUTP_APSDFLR_cm"
  VAPM_APSDFLL_cm/1 -> VAPM_APSDFLL_cm_Inproc/1  "VAPM_APSDFLL_cm"
  VAPM_APSDFLL_cm_Inproc/1 -> UnitConverter20/1
  UnitConverter20/1 -> VOUTP_APSDFLL_cm/1  "VOUTP_APSDFLL_cm"
  VAPM_PASAFCL_enum/1 -> VAPM_PASAFCL_enum_Inproc/1  "VAPM_PASAFCL_enum"
  VAPM_PASAFCL_enum_Inproc/1 -> UnitConverter21/1
  UnitConverter21/1 -> VOUTP_PASAFCL_enum/1  "VOUTP_PASAFCL_enum"
  VAPM_PASARMR_enum/1 -> VAPM_PASARMR_enum_Inproc/1  "VAPM_PASARMR_enum"
  VAPM_PASARMR_enum_Inproc/1 -> UnitConverter22/1
  UnitConverter22/1 -> VOUTP_PASARMR_enum/1  "VOUTP_PASARMR_enum"
  VAPM_PASARML_enum/1 -> VAPM_PASARML_enum_Inproc/1  "VAPM_PASARML_enum"
  VAPM_PASARML_enum_Inproc/1 -> UnitConverter23/1
  UnitConverter23/1 -> VOUTP_PASARML_enum/1  "VOUTP_PASARML_enum"
  VAPM_PASARCR_enum/1 -> VAPM_PASARCR_enum_Inproc/1  "VAPM_PASARCR_enum"
  VAPM_PASARCR_enum_Inproc/1 -> UnitConverter24/1
  UnitConverter24/1 -> VOUTP_PASARCR_enum/1  "VOUTP_PASARCR_enum"
  VAPM_PASARCL_enum/1 -> VAPM_PASARCL_enum_Inproc/1  "VAPM_PASARCL_enum"
  VAPM_PASARCL_enum_Inproc/1 -> UnitConverter25/1
  UnitConverter25/1 -> VOUTP_PASARCL_enum/1  "VOUTP_PASARCL_enum"
  VAPM_PASAFMR_enum/1 -> VAPM_PASAFMR_enum_Inproc/1  "VAPM_PASAFMR_enum"
  VAPM_PASAFMR_enum_Inproc/1 -> UnitConverter26/1
  UnitConverter26/1 -> VOUTP_PASAFMR_enum/1  "VOUTP_PASAFMR_enum"
  VAPM_PASAFML_enum/1 -> VAPM_PASAFML_enum_Inproc/1  "VAPM_PASAFML_enum"
  VAPM_PASAFML_enum_Inproc/1 -> UnitConverter27/1
  UnitConverter27/1 -> VOUTP_PASAFML_enum/1  "VOUTP_PASAFML_enum"
  VAPM_PASAFCR_enum/1 -> VAPM_PASAFCR_enum_Inproc/1  "VAPM_PASAFCR_enum"
  VAPM_PASAFCR_enum_Inproc/1 -> UnitConverter28/1
  UnitConverter28/1 -> VOUTP_PASAFCR_enum/1  "VOUTP_PASAFCR_enum"
  VAPM_USSStaRMR_flg/1 -> VAPM_USSStaRMR_flg_Inproc/1  "VAPM_USSStaRMR_flg"
  VAPM_USSStaRMR_flg_Inproc/1 -> UnitConverter29/1
  UnitConverter29/1 -> VOUTP_USSStaRMR_flg/1  "VOUTP_USSStaRMR_flg"
  VAPM_USSStaRML_flg/1 -> VAPM_USSStaRML_flg_Inproc/1  "VAPM_USSStaRML_flg"
  VAPM_USSStaRML_flg_Inproc/1 -> UnitConverter30/1
  UnitConverter30/1 -> VOUTP_USSStaRML_flg/1  "VOUTP_USSStaRML_flg"
  VAPM_USSStaRLR_flg/1 -> VAPM_USSStaRLR_flg_Inproc/1  "VAPM_USSStaRLR_flg"
  VAPM_USSStaRLR_flg_Inproc/1 -> UnitConverter31/1
  UnitConverter31/1 -> VOUTP_USSStaRLR_flg/1  "VOUTP_USSStaRLR_flg"
  VAPM_USSStaRLL_flg/1 -> VAPM_USSStaRLL_flg_Inproc/1  "VAPM_USSStaRLL_flg"
  VAPM_USSStaRLL_flg_Inproc/1 -> UnitConverter32/1
  UnitConverter32/1 -> VOUTP_USSStaRLL_flg/1  "VOUTP_USSStaRLL_flg"
  VAPM_USSStaRCR_flg/1 -> VAPM_USSStaRCR_flg_Inproc/1  "VAPM_USSStaRCR_flg"
  VAPM_USSStaRCR_flg_Inproc/1 -> UnitConverter33/1
  UnitConverter33/1 -> VOUTP_USSStaRCR_flg/1  "VOUTP_USSStaRCR_flg"
  VAPM_USSStaRCL_flg/1 -> VAPM_USSStaRCL_flg_Inproc/1  "VAPM_USSStaRCL_flg"
  VAPM_USSStaRCL_flg_Inproc/1 -> UnitConverter34/1
  UnitConverter34/1 -> VOUTP_USSStaRCL_flg/1  "VOUTP_USSStaRCL_flg"
  VAPM_USSStaFMR_flg/1 -> VAPM_USSStaFMR_flg_Inproc/1  "VAPM_USSStaFMR_flg"
  VAPM_USSStaFMR_flg_Inproc/1 -> UnitConverter35/1
  UnitConverter35/1 -> VOUTP_USSStaFMR_flg/1  "VOUTP_USSStaFMR_flg"
  VAPM_USSStaFML_flg/1 -> VAPM_USSStaFML_flg_Inproc/1  "VAPM_USSStaFML_flg"
  VAPM_USSStaFML_flg_Inproc/1 -> UnitConverter36/1
  UnitConverter36/1 -> VOUTP_USSStaFML_flg/1  "VOUTP_USSStaFML_flg"
  VAPM_USSStaFLR_flg/1 -> VAPM_USSStaFLR_flg_Inproc/1  "VAPM_USSStaFLR_flg"
  VAPM_USSStaFLR_flg_Inproc/1 -> UnitConverter37/1
  UnitConverter37/1 -> VOUTP_USSStaFLR_flg/1  "VOUTP_USSStaFLR_flg"
  VAPM_USSStaFLL_flg/1 -> VAPM_USSStaFLL_flg_Inproc/1  "VAPM_USSStaFLL_flg"
  VAPM_USSStaFLL_flg_Inproc/1 -> UnitConverter38/1
  UnitConverter38/1 -> VOUTP_USSStaFLL_flg/1  "VOUTP_USSStaFLL_flg"
  VAPM_USSStaFCR_flg/1 -> VAPM_USSStaFCR_flg_Inproc/1  "VAPM_USSStaFCR_flg"
  VAPM_USSStaFCR_flg_Inproc/1 -> UnitConverter39/1
  UnitConverter39/1 -> VOUTP_USSStaFCR_flg/1  "VOUTP_USSStaFCR_flg"
  VAPM_USSStaFCL_flg/1 -> VAPM_USSStaFCL_flg_Inproc/1  "VAPM_USSStaFCL_flg"
  VAPM_USSStaFCL_flg_Inproc/1 -> UnitConverter40/1
  UnitConverter40/1 -> VOUTP_USSStaFCL_flg/1  "VOUTP_USSStaFCL_flg"
  VAPM_Chime_enum/1 -> VAPM_Chime_enum_Inproc/1  "VAPM_Chime_enum"
  VAPM_Chime_enum_Inproc/1 -> UnitConverter41/1
  UnitConverter41/1 -> VOUTP_Chime_enum/1  "VOUTP_Chime_enum"
  VAPM_SNSRLayout_enum/1 -> VAPM_SNSRLayout_enum_Inproc/1  "VAPM_SNSRLayout_enum"
  VAPM_SNSRLayout_enum_Inproc/1 -> UnitConverter42/1
  UnitConverter42/1 -> VOUTP_SNSRLayout_enum/1  "VOUTP_SNSRLayout_enum"
  VAPM_StaFSya_flg/1 -> VAPM_StaFSya_flg_Inproc/1  "VAPM_StaFSya_flg"
  VAPM_StaFSya_flg_Inproc/1 -> UnitConverter43/1
  UnitConverter43/1 -> VOUTP_StaFSya_flg/1  "VOUTP_StaFSya_flg"
  VAPM_ModOperation_enum/1 -> VAPM_ModOperation_enum_Inproc/1  "VAPM_ModOperation_enum"
  VAPM_ModOperation_enum_Inproc/1 -> UnitConverter44/1
  UnitConverter44/1 -> VOUTP_ModOperation_enum/1  "VOUTP_ModOperation_enum"
  VAPM_BrkPedalPos_pct/1 -> VAPM_BrkPedalPos_pct_Inproc/1  "VAPM_BrkPedalPos_pct"
  VAPM_BrkPedalPos_pct_Inproc/1 -> UnitConverter45/1
  UnitConverter45/1 -> VOUTP_BrkPedalPos_pct/1  "VOUTP_BrkPedalPos_pct"
  VAPM_BrkPedalPosTimeOut_flg/1 -> VAPM_BrkPedalPosTimeOut_flg_Inproc/1  "VAPM_BrkPedalPosTimeOut_flg"
  VAPM_BrkPedalPosTimeOut_flg_Inproc/1 -> UnitConverter46/1
  UnitConverter46/1 -> VOUTP_BrkPedalPosTimeOut_flg/1  "VOUTP_BrkPedalPosTimeOut_flg"
  VAPM_LFRawWhlSpeed_kph/1 -> VAPM_LFRawWhlSpeed_kph_Inproc/1  "VAPM_LFRawWhlSpeed_kph"
  VAPM_LFRawWhlSpeed_kph_Inproc/1 -> UnitConverter47/1
  UnitConverter47/1 -> VOUTP_LFRawWhlSpeed_kph/1  "VOUTP_LFRawWhlSpeed_kph"
  VAPM_LFRawWhlSpeedTimeOut_flg/1 -> VAPM_LFRawWhlSpeedTimeOut_flg_Inproc/1  "VAPM_LFRawWhlSpeedTimeOut_flg"
  VAPM_LFRawWhlSpeedTimeOut_flg_Inproc/1 -> UnitConverter48/1
  UnitConverter48/1 -> VOUTP_LFRawWhlSpeedTimeOut_flg/1  "VOUTP_LFRawWhlSpeedTimeOut_flg"
  VAPM_RFRawWhlSpeed_kph/1 -> VAPM_RFRawWhlSpeed_kph_Inproc/1  "VAPM_RFRawWhlSpeed_kph"
  VAPM_RFRawWhlSpeed_kph_Inproc/1 -> UnitConverter49/1
  UnitConverter49/1 -> VOUTP_RFRawWhlSpeed_kph/1  "VOUTP_RFRawWhlSpeed_kph"
  VAPM_RFRawWhlSpeedTimeOut_flg/1 -> VAPM_RFRawWhlSpeedTimeOut_flg_Inproc/1  "VAPM_RFRawWhlSpeedTimeOut_flg"
  VAPM_RFRawWhlSpeedTimeOut_flg_Inproc/1 -> UnitConverter50/1
  UnitConverter50/1 -> VOUTP_RFRawWhlSpeedTimeOut_flg/1  "VOUTP_RFRawWhlSpeedTimeOut_flg"
  VAPM_LRRawWhlSpeed_kph/1 -> VAPM_LRRawWhlSpeed_kph_Inproc/1  "VAPM_LRRawWhlSpeed_kph"
  VAPM_LRRawWhlSpeed_kph_Inproc/1 -> UnitConverter51/1
  UnitConverter51/1 -> VOUTP_LRRawWhlSpeed_kph/1  "VOUTP_LRRawWhlSpeed_kph"
  VAPM_LRRawWhlSpeedTimeOut_flg/1 -> VAPM_LRRawWhlSpeedTimeOut_flg_Inproc/1  "VAPM_LRRawWhlSpeedTimeOut_flg"
  VAPM_LRRawWhlSpeedTimeOut_flg_Inproc/1 -> UnitConverter52/1
  UnitConverter52/1 -> VOUTP_LRRawWhlSpeedTimeOut_flg/1  "VOUTP_LRRawWhlSpeedTimeOut_flg"
  VAPM_RRRawWhlSpeed_kph/1 -> VAPM_RRRawWhlSpeed_kph_Inproc/1  "VAPM_RRRawWhlSpeed_kph"
  VAPM_RRRawWhlSpeed_kph_Inproc/1 -> UnitConverter53/1
  UnitConverter53/1 -> VOUTP_RRRawWhlSpeed_kph/1  "VOUTP_RRRawWhlSpeed_kph"
  VAPM_RRRawWhlSpeedTimeOut_flg/1 -> VAPM_RRRawWhlSpeedTimeOut_flg_Inproc/1  "VAPM_RRRawWhlSpeedTimeOut_flg"
  VAPM_RRRawWhlSpeedTimeOut_flg_Inproc/1 -> UnitConverter54/1
  UnitConverter54/1 -> VOUTP_RRRawWhlSpeedTimeOut_flg/1  "VOUTP_RRRawWhlSpeedTimeOut_flg"
  VAPM_LFRawWhlSpeedV_flg/1 -> VAPM_LFRawWhlSpeedV_flg_Inproc/1  "VAPM_LFRawWhlSpeedV_flg"
  VAPM_LFRawWhlSpeedV_flg_Inproc/1 -> UnitConverter55/1
  UnitConverter55/1 -> VOUTP_LFRawWhlSpeedV_flg/1  "VOUTP_LFRawWhlSpeedV_flg"
  VAPM_LFRawWhlSpeedVTimeOut_flg/1 -> VAPM_LFRawWhlSpeedVTimeOut_flg_Inproc/1  "VAPM_LFRawWhlSpeedVTimeOut_flg"
  VAPM_LFRawWhlSpeedVTimeOut_flg_Inproc/1 -> UnitConverter56/1
  UnitConverter56/1 -> VOUTP_LFRawWhlSpeedVTimeOut_flg/1  "VOUTP_LFRawWhlSpeedVTimeOut_flg"
  VAPM_RFRawWhlSpeedV_flg/1 -> VAPM_RFRawWhlSpeedV_flg_Inproc/1  "VAPM_RFRawWhlSpeedV_flg"
  VAPM_RFRawWhlSpeedV_flg_Inproc/1 -> UnitConverter57/1
  UnitConverter57/1 -> VOUTP_RFRawWhlSpeedV_flg/1  "VOUTP_RFRawWhlSpeedV_flg"
  VAPM_RFRawWhlSpeedVTimeOut_flg/1 -> VAPM_RFRawWhlSpeedVTimeOut_flg_Inproc/1  "VAPM_RFRawWhlSpeedVTimeOut_flg"
  VAPM_RFRawWhlSpeedVTimeOut_flg_Inproc/1 -> UnitConverter58/1
  UnitConverter58/1 -> VOUTP_RFRawWhlSpeedVTimeOut_flg/1  "VOUTP_RFRawWhlSpeedVTimeOut_flg"
  VAPM_LRRawWhlSpeedV_flg/1 -> VAPM_LRRawWhlSpeedV_flg_Inproc/1  "VAPM_LRRawWhlSpeedV_flg"
  VAPM_LRRawWhlSpeedV_flg_Inproc/1 -> UnitConverter59/1
  UnitConverter59/1 -> VOUTP_LRRawWhlSpeedV_flg/1  "VOUTP_LRRawWhlSpeedV_flg"
  VAPM_LRRawWhlSpeedVTimeOut_flg/1 -> VAPM_LRRawWhlSpeedVTimeOut_flg_Inproc/1  "VAPM_LRRawWhlSpeedVTimeOut_flg"
  VAPM_LRRawWhlSpeedVTimeOut_flg_Inproc/1 -> UnitConverter60/1
  UnitConverter60/1 -> VOUTP_LRRawWhlSpeedVTimeOut_flg/1  "VOUTP_LRRawWhlSpeedVTimeOut_flg"
  VAPM_RRRawWhlSpeedV_flg/1 -> VAPM_RRRawWhlSpeedV_flg_Inproc/1  "VAPM_RRRawWhlSpeedV_flg"
  VAPM_RRRawWhlSpeedV_flg_Inproc/1 -> UnitConverter61/1
  UnitConverter61/1 -> VOUTP_RRRawWhlSpeedV_flg/1  "VOUTP_RRRawWhlSpeedV_flg"
  VAPM_RRRawWhlSpeedVTimeOut_flg/1 -> VAPM_RRRawWhlSpeedVTimeOut_flg_Inproc/1  "VAPM_RRRawWhlSpeedVTimeOut_flg"
  VAPM_RRRawWhlSpeedVTimeOut_flg_Inproc/1 -> UnitConverter62/1
  UnitConverter62/1 -> VOUTP_RRRawWhlSpeedVTimeOut_flg/1  "VOUTP_RRRawWhlSpeedVTimeOut_flg"
  VAPM_LFWhlRotDir_enum/1 -> VAPM_LFWhlRotDir_enum_Inproc/1  "VAPM_LFWhlRotDir_enum"
  VAPM_LFWhlRotDir_enum_Inproc/1 -> UnitConverter63/1
  UnitConverter63/1 -> VOUTP_LFWhlRotDir_enum/1  "VOUTP_LFWhlRotDir_enum"
  VAPM_LFWhlRotDirTimeOut_flg/1 -> VAPM_LFWhlRotDirTimeOut_flg_Inproc/1  "VAPM_LFWhlRotDirTimeOut_flg"
  VAPM_LFWhlRotDirTimeOut_flg_Inproc/1 -> UnitConverter64/1
  UnitConverter64/1 -> VOUTP_LFWhlRotDirTimeOut_flg/1  "VOUTP_LFWhlRotDirTimeOut_flg"
  VAPM_RFWhlRotDir_enum/1 -> VAPM_RFWhlRotDir_enum_Inproc/1  "VAPM_RFWhlRotDir_enum"
  VAPM_RFWhlRotDir_enum_Inproc/1 -> UnitConverter65/1
  UnitConverter65/1 -> VOUTP_RFWhlRotDir_enum/1  "VOUTP_RFWhlRotDir_enum"
  VAPM_RFWhlRotDirTimeOut_flg/1 -> VAPM_RFWhlRotDirTimeOut_flg_Inproc/1  "VAPM_RFWhlRotDirTimeOut_flg"
  VAPM_RFWhlRotDirTimeOut_flg_Inproc/1 -> UnitConverter66/1
  UnitConverter66/1 -> VOUTP_RFWhlRotDirTimeOut_flg/1  "VOUTP_RFWhlRotDirTimeOut_flg"
  VAPM_LRWhlRotDir_enum/1 -> VAPM_LRWhlRotDir_enum_Inproc/1  "VAPM_LRWhlRotDir_enum"
  VAPM_LRWhlRotDir_enum_Inproc/1 -> UnitConverter67/1
  UnitConverter67/1 -> VOUTP_LRWhlRotDir_enum/1  "VOUTP_LRWhlRotDir_enum"
  VAPM_LRWhlRotDirTimeOut_flg/1 -> VAPM_LRWhlRotDirTimeOut_flg_Inproc/1  "VAPM_LRWhlRotDirTimeOut_flg"
  VAPM_LRWhlRotDirTimeOut_flg_Inproc/1 -> UnitConverter68/1
  UnitConverter68/1 -> VOUTP_LRWhlRotDirTimeOut_flg/1  "VOUTP_LRWhlRotDirTimeOut_flg"
  VAPM_RRWhlRotDir_enum/1 -> VAPM_RRWhlRotDir_enum_Inproc/1  "VAPM_RRWhlRotDir_enum"
  VAPM_RRWhlRotDir_enum_Inproc/1 -> UnitConverter69/1
  UnitConverter69/1 -> VOUTP_RRWhlRotDir_enum/1  "VOUTP_RRWhlRotDir_enum"
  VAPM_RRWhlRotDirTimeOut_flg/1 -> VAPM_RRWhlRotDirTimeOut_flg_Inproc/1  "VAPM_RRWhlRotDirTimeOut_flg"
  VAPM_RRWhlRotDirTimeOut_flg_Inproc/1 -> UnitConverter70/1
  UnitConverter70/1 -> VOUTP_RRWhlRotDirTimeOut_flg/1  "VOUTP_RRWhlRotDirTimeOut_flg"
  VAPM_LFPulseCountV_flg/1 -> VAPM_LFPulseCountV_flg_Inproc/1  "VAPM_LFPulseCountV_flg"
  VAPM_LFPulseCountV_flg_Inproc/1 -> UnitConverter71/1
  UnitConverter71/1 -> VOUTP_LFPulseCountV_flg/1  "VOUTP_LFPulseCountV_flg"
  VAPM_LFPulseCountVTimeOut_flg/1 -> VAPM_LFPulseCountVTimeOut_flg_Inproc/1  "VAPM_LFPulseCountVTimeOut_flg"
  VAPM_LFPulseCountVTimeOut_flg_Inproc/1 -> UnitConverter72/1
  UnitConverter72/1 -> VOUTP_LFPulseCountVTimeOut_flg/1  "VOUTP_LFPulseCountVTimeOut_flg"
  VAPM_RFPulseCountV_flg/1 -> VAPM_RFPulseCountV_flg_Inproc/1  "VAPM_RFPulseCountV_flg"
  VAPM_RFPulseCountV_flg_Inproc/1 -> UnitConverter73/1
  UnitConverter73/1 -> VOUTP_RFPulseCountV_flg/1  "VOUTP_RFPulseCountV_flg"
  VAPM_RFPulseCountVTimeOut_flg/1 -> VAPM_RFPulseCountVTimeOut_flg_Inproc/1  "VAPM_RFPulseCountVTimeOut_flg"
  VAPM_RFPulseCountVTimeOut_flg_Inproc/1 -> UnitConverter74/1
  UnitConverter74/1 -> VOUTP_RFPulseCountVTimeOut_flg/1  "VOUTP_RFPulseCountVTimeOut_flg"
  VAPM_LRPulseCountV_flg/1 -> VAPM_LRPulseCountV_flg_Inproc/1  "VAPM_LRPulseCountV_flg"
  VAPM_LRPulseCountV_flg_Inproc/1 -> UnitConverter75/1
  UnitConverter75/1 -> VOUTP_LRPulseCountV_flg/1  "VOUTP_LRPulseCountV_flg"
  VAPM_LRPulseCountVTimeOut_flg/1 -> VAPM_LRPulseCountVTimeOut_flg_Inproc/1  "VAPM_LRPulseCountVTimeOut_flg"
  VAPM_LRPulseCountVTimeOut_flg_Inproc/1 -> UnitConverter76/1
  UnitConverter76/1 -> VOUTP_LRPulseCountVTimeOut_flg/1  "VOUTP_LRPulseCountVTimeOut_flg"
  VAPM_RRPulseCountV_flg/1 -> VAPM_RRPulseCountV_flg_Inproc/1  "VAPM_RRPulseCountV_flg"
  VAPM_RRPulseCountV_flg_Inproc/1 -> UnitConverter77/1
  UnitConverter77/1 -> VOUTP_RRPulseCountV_flg/1  "VOUTP_RRPulseCountV_flg"
  VAPM_RRPulseCountVTimeOut_flg/1 -> VAPM_RRPulseCountVTimeOut_flg_Inproc/1  "VAPM_RRPulseCountVTimeOut_flg"
  VAPM_RRPulseCountVTimeOut_flg_Inproc/1 -> UnitConverter78/1
  UnitConverter78/1 -> VOUTP_RRPulseCountVTimeOut_flg/1  "VOUTP_RRPulseCountVTimeOut_flg"
  VAPM_LFPulseCount_enum/1 -> VAPM_LFPulseCount_enum_Inproc/1  "VAPM_LFPulseCount_enum"
  VAPM_LFPulseCount_enum_Inproc/1 -> UnitConverter79/1
  UnitConverter79/1 -> VOUTP_LFPulseCount_enum/1  "VOUTP_LFPulseCount_enum"
  VAPM_LFPulseCountTimeOut_flg/1 -> VAPM_LFPulseCountTimeOut_flg_Inproc/1  "VAPM_LFPulseCountTimeOut_flg"
  VAPM_LFPulseCountTimeOut_flg_Inproc/1 -> UnitConverter80/1
  UnitConverter80/1 -> VOUTP_LFPulseCountTimeOut_flg/1  "VOUTP_LFPulseCountTimeOut_flg"
  VAPM_RFPulseCount_enum/1 -> VAPM_RFPulseCount_enum_Inproc/1  "VAPM_RFPulseCount_enum"
  VAPM_RFPulseCount_enum_Inproc/1 -> UnitConverter81/1
  UnitConverter81/1 -> VOUTP_RFPulseCount_enum/1  "VOUTP_RFPulseCount_enum"
  VAPM_RFPulseCountTimeOut_flg/1 -> VAPM_RFPulseCountTimeOut_flg_Inproc/1  "VAPM_RFPulseCountTimeOut_flg"
  VAPM_RFPulseCountTimeOut_flg_Inproc/1 -> UnitConverter82/1
  UnitConverter82/1 -> VOUTP_RFPulseCountTimeOut_flg/1  "VOUTP_RFPulseCountTimeOut_flg"
  VAPM_LRPulseCount_enum/1 -> VAPM_LRPulseCount_enum_Inproc/1  "VAPM_LRPulseCount_enum"
  VAPM_LRPulseCount_enum_Inproc/1 -> UnitConverter83/1
  UnitConverter83/1 -> VOUTP_LRPulseCount_enum/1  "VOUTP_LRPulseCount_enum"
  VAPM_LRPulseCountTimeOut_flg/1 -> VAPM_LRPulseCountTimeOut_flg_Inproc/1  "VAPM_LRPulseCountTimeOut_flg"
  VAPM_LRPulseCountTimeOut_flg_Inproc/1 -> UnitConverter84/1
  UnitConverter84/1 -> VOUTP_LRPulseCountTimeOut_flg/1  "VOUTP_LRPulseCountTimeOut_flg"
  VAPM_RRPulseCount_enum/1 -> VAPM_RRPulseCount_enum_Inproc/1  "VAPM_RRPulseCount_enum"
  VAPM_RRPulseCount_enum_Inproc/1 -> UnitConverter85/1
  UnitConverter85/1 -> VOUTP_RRPulseCount_enum/1  "VOUTP_RRPulseCount_enum"
  VAPM_RRPulseCountTimeOut_flg/1 -> VAPM_RRPulseCountTimeOut_flg_Inproc/1  "VAPM_RRPulseCountTimeOut_flg"
  VAPM_RRPulseCountTimeOut_flg_Inproc/1 -> UnitConverter86/1
  UnitConverter86/1 -> VOUTP_RRPulseCountTimeOut_flg/1  "VOUTP_RRPulseCountTimeOut_flg"
  VAPM_ShifterHandleCmd_enum/1 -> VAPM_ShifterHandleCmd_enum_Inproc/1  "VAPM_ShifterHandleCmd_enum"
  VAPM_ShifterHandleCmd_enum_Inproc/1 -> UnitConverter87/1
  UnitConverter87/1 -> VOUTP_ShifterHandleCmd_enum/1  "VOUTP_ShifterHandleCmd_enum"
  VAPM_ShifterHandleCmdTimeOut_flg/1 -> VAPM_ShifterHandleCmdTimeOut_flg_Inproc/1  "VAPM_ShifterHandleCmdTimeOut_flg"
  VAPM_ShifterHandleCmdTimeOut_flg_Inproc/1 -> UnitConverter88/1
  UnitConverter88/1 -> VOUTP_ShifterHandleCmdTimeOut_flg/1  "VOUTP_ShifterHandleCmdTimeOut_flg"
  VAPM_DriIntend_enum/1 -> VAPM_DriIntend_enum_Inproc/1  "VAPM_DriIntend_enum"
  VAPM_DriIntend_enum_Inproc/1 -> UnitConverter89/1
  UnitConverter89/1 -> VOUTP_DriIntend_enum/1  "VOUTP_DriIntend_enum"
  VAPM_DriIntendTimeOut_flg/1 -> VAPM_DriIntendTimeOut_flg_Inproc/1  "VAPM_DriIntendTimeOut_flg"
  VAPM_DriIntendTimeOut_flg_Inproc/1 -> UnitConverter90/1
  UnitConverter90/1 -> VOUTP_DriIntendTimeOut_flg/1  "VOUTP_DriIntendTimeOut_flg"
  VAPM_EPSAOIControl_enum/1 -> VAPM_EPSAOIControl_enum_Inproc/1  "VAPM_EPSAOIControl_enum"
  VAPM_EPSAOIControl_enum_Inproc/1 -> UnitConverter91/1
  UnitConverter91/1 -> VOUTP_EPSAOIControl_enum/1  "VOUTP_EPSAOIControl_enum"
  VAPM_EPSAOIControlTimeOut_flg/1 -> VAPM_EPSAOIControlTimeOut_flg_Inproc/1  "VAPM_EPSAOIControlTimeOut_flg"
  VAPM_EPSAOIControlTimeOut_flg_Inproc/1 -> UnitConverter92/1
  UnitConverter92/1 -> VOUTP_EPSAOIControlTimeOut_flg/1  "VOUTP_EPSAOIControlTimeOut_flg"
  VAPM_SASAngle_Deg/1 -> VAPM_SASAngle_Deg_Inproc/1  "VAPM_SASAngle_Deg"
  VAPM_SASAngle_Deg_Inproc/1 -> UnitConverter93/1
  UnitConverter93/1 -> VOUTP_SASAngle_Deg/1  "VOUTP_SASAngle_Deg"
  VAPM_SASAngleTimeOut_flg/1 -> VAPM_SASAngleTimeOut_flg_Inproc/1  "VAPM_SASAngleTimeOut_flg"
  VAPM_SASAngleTimeOut_flg_Inproc/1 -> UnitConverter94/1
  UnitConverter94/1 -> VOUTP_SASAngleTimeOut_flg/1  "VOUTP_SASAngleTimeOut_flg"
  VAPM_SASSpeed_degps/1 -> VAPM_SASSpeed_degps_Inproc/1  "VAPM_SASSpeed_degps"
  VAPM_SASSpeed_degps_Inproc/1 -> UnitConverter95/1
  UnitConverter95/1 -> VOUTP_SASSpeed_degps/1  "VOUTP_SASSpeed_degps"
  VAPM_SASSpeedTimeOut_flg/1 -> VAPM_SASSpeedTimeOut_flg_Inproc/1  "VAPM_SASSpeedTimeOut_flg"
  VAPM_SASSpeedTimeOut_flg_Inproc/1 -> UnitConverter96/1
  UnitConverter96/1 -> VOUTP_SASSpeedTimeOut_flg/1  "VOUTP_SASSpeedTimeOut_flg"
  VAPM_SASSpeedValid_flg/1 -> VAPM_SASSpeedValid_flg_Inproc/1  "VAPM_SASSpeedValid_flg"
  VAPM_SASSpeedValid_flg_Inproc/1 -> UnitConverter97/1
  UnitConverter97/1 -> VOUTP_SASSpeedValid_flg/1  "VOUTP_SASSpeedValid_flg"
  VAPM_SASSpeedValidTimeOut_flg/1 -> VAPM_SASSpeedValidTimeOut_flg_Inproc/1  "VAPM_SASSpeedValidTimeOut_flg"
  VAPM_SASSpeedValidTimeOut_flg_Inproc/1 -> UnitConverter98/1
  UnitConverter98/1 -> VOUTP_SASSpeedValidTimeOut_flg/1  "VOUTP_SASSpeedValidTimeOut_flg"
  VAPM_SASCAL_flg/1 -> VAPM_SASCAL_flg_Inproc/1  "VAPM_SASCAL_flg"
  VAPM_SASCAL_flg_Inproc/1 -> UnitConverter99/1
  UnitConverter99/1 -> VOUTP_SASCAL_flg/1  "VOUTP_SASCAL_flg"
  VAPM_SASCALTimeOut_flg/1 -> VAPM_SASCALTimeOut_flg_Inproc/1  "VAPM_SASCALTimeOut_flg"
  VAPM_SASCALTimeOut_flg_Inproc/1 -> UnitConverter100/1
  UnitConverter100/1 -> VOUTP_SASCALTimeOut_flg/1  "VOUTP_SASCALTimeOut_flg"
  VAPM_SASV_flg/1 -> VAPM_SASV_flg_Inproc/1  "VAPM_SASV_flg"
  VAPM_SASV_flg_Inproc/1 -> UnitConverter101/1
  UnitConverter101/1 -> VOUTP_SASV_flg/1  "VOUTP_SASV_flg"
  VAPM_SASVTimeOut_flg/1 -> VAPM_SASVTimeOut_flg_Inproc/1  "VAPM_SASVTimeOut_flg"
  VAPM_SASVTimeOut_flg_Inproc/1 -> UnitConverter102/1
  UnitConverter102/1 -> VOUTP_SASVTimeOut_flg/1  "VOUTP_SASVTimeOut_flg"
  VAPM_GRADE_Deg/1 -> VAPM_GRADE_Deg_Inproc/1  "VAPM_GRADE_Deg"
  VAPM_GRADE_Deg_Inproc/1 -> UnitConverter103/1
  UnitConverter103/1 -> VOUTP_GRADE_Deg/1  "VOUTP_GRADE_Deg"
  VAPM_GRADETimeOut_flg/1 -> VAPM_GRADETimeOut_flg_Inproc/1  "VAPM_GRADETimeOut_flg"
  VAPM_GRADETimeOut_flg_Inproc/1 -> UnitConverter104/1
  UnitConverter104/1 -> VOUTP_GRADETimeOut_flg/1  "VOUTP_GRADETimeOut_flg"
  VAPM_YawRate_degps/1 -> VAPM_YawRate_degps_Inproc/1  "VAPM_YawRate_degps"
  VAPM_YawRate_degps_Inproc/1 -> UnitConverter105/1
  UnitConverter105/1 -> VOUTP_YawRate_degps/1  "VOUTP_YawRate_degps"
  VAPM_YawRateTimeOut_flg/1 -> VAPM_YawRateTimeOut_flg_Inproc/1  "VAPM_YawRateTimeOut_flg"
  VAPM_YawRateTimeOut_flg_Inproc/1 -> UnitConverter106/1
  UnitConverter106/1 -> VOUTP_YawRateTimeOut_flg/1  "VOUTP_YawRateTimeOut_flg"
  VAPM_LatAccel_Gps/1 -> VAPM_LatAccel_Gps_Inproc/1  "VAPM_LatAccel_Gps"
  VAPM_LatAccel_Gps_Inproc/1 -> UnitConverter107/1
  UnitConverter107/1 -> VOUTP_LatAccel_Gps/1  "VOUTP_LatAccel_Gps"
  VAPM_LatAccelTimeOut_flg/1 -> VAPM_LatAccelTimeOut_flg_Inproc/1  "VAPM_LatAccelTimeOut_flg"
  VAPM_LatAccelTimeOut_flg_Inproc/1 -> UnitConverter108/1
  UnitConverter108/1 -> VOUTP_LatAccelTimeOut_flg/1  "VOUTP_LatAccelTimeOut_flg"
  VAPM_LongAccel_Gps/1 -> VAPM_LongAccel_Gps_Inproc/1  "VAPM_LongAccel_Gps"
  VAPM_LongAccel_Gps_Inproc/1 -> UnitConverter109/1
  UnitConverter109/1 -> VOUTP_LongAccel_Gps/1  "VOUTP_LongAccel_Gps"
  VAPM_LongAccelTimeOut_flg/1 -> VAPM_LongAccelTimeOut_flg_Inproc/1  "VAPM_LongAccelTimeOut_flg"
  VAPM_LongAccelTimeOut_flg_Inproc/1 -> UnitConverter110/1
  UnitConverter110/1 -> VOUTP_LongAccelTimeOut_flg/1  "VOUTP_LongAccelTimeOut_flg"
  VAPM_MCPressure_bar/1 -> VAPM_MCPressure_bar_Inproc/1  "VAPM_MCPressure_bar"
  VAPM_MCPressure_bar_Inproc/1 -> UnitConverter111/1
  UnitConverter111/1 -> VOUTP_MCPressure_bar/1  "VOUTP_MCPressure_bar"
  VAPM_MCPressureTimeOut_flg/1 -> VAPM_MCPressureTimeOut_flg_Inproc/1  "VAPM_MCPressureTimeOut_flg"
  VAPM_MCPressureTimeOut_flg_Inproc/1 -> UnitConverter112/1
  UnitConverter112/1 -> VOUTP_MCPressureTimeOut_flg/1  "VOUTP_MCPressureTimeOut_flg"
  VAPM_YawRateV_flg/1 -> VAPM_YawRateV_flg_Inproc/1  "VAPM_YawRateV_flg"
  VAPM_YawRateV_flg_Inproc/1 -> UnitConverter113/1
  UnitConverter113/1 -> VOUTP_YawRateV_flg/1  "VOUTP_YawRateV_flg"
  VAPM_YawRateVTimeOut_flg/1 -> VAPM_YawRateVTimeOut_flg_Inproc/1  "VAPM_YawRateVTimeOut_flg"
  VAPM_YawRateVTimeOut_flg_Inproc/1 -> UnitConverter114/1
  UnitConverter114/1 -> VOUTP_YawRateVTimeOut_flg/1  "VOUTP_YawRateVTimeOut_flg"
  VAPM_LatAccelV_flg/1 -> VAPM_LatAccelV_flg_Inproc/1  "VAPM_LatAccelV_flg"
  VAPM_LatAccelV_flg_Inproc/1 -> UnitConverter115/1
  UnitConverter115/1 -> VOUTP_LatAccelV_flg/1  "VOUTP_LatAccelV_flg"
  VAPM_LatAccelVTimeOut_flg/1 -> VAPM_LatAccelVTimeOut_flg_Inproc/1  "VAPM_LatAccelVTimeOut_flg"
  VAPM_LatAccelVTimeOut_flg_Inproc/1 -> UnitConverter116/1
  UnitConverter116/1 -> VOUTP_LatAccelVTimeOut_flg/1  "VOUTP_LatAccelVTimeOut_flg"
  VAPM_LongAccelV_flg/1 -> VAPM_LongAccelV_flg_Inproc/1  "VAPM_LongAccelV_flg"
  VAPM_LongAccelV_flg_Inproc/1 -> UnitConverter117/1
  UnitConverter117/1 -> VOUTP_LongAccelV_flg/1  "VOUTP_LongAccelV_flg"
  VAPM_LongAccelVTimeOut_flg/1 -> VAPM_LongAccelVTimeOut_flg_Inproc/1  "VAPM_LongAccelVTimeOut_flg"
  VAPM_LongAccelVTimeOut_flg_Inproc/1 -> UnitConverter118/1
  UnitConverter118/1 -> VOUTP_LongAccelVTimeOut_flg/1  "VOUTP_LongAccelVTimeOut_flg"
  VAPM_MCPressureV_bar/1 -> VAPM_MCPressureV_bar_Inproc/1  "VAPM_MCPressureV_bar"
  VAPM_MCPressureV_bar_Inproc/1 -> UnitConverter119/1
  UnitConverter119/1 -> VOUTP_MCPressureV_bar/1  "VOUTP_MCPressureV_bar"
  VAPM_MCPressureVTimeOut_flg/1 -> VAPM_MCPressureVTimeOut_flg_Inproc/1  "VAPM_MCPressureVTimeOut_flg"
  VAPM_MCPressureVTimeOut_flg_Inproc/1 -> UnitConverter120/1
  UnitConverter120/1 -> VOUTP_MCPressureVTimeOut_flg/1  "VOUTP_MCPressureVTimeOut_flg"
  VAPM_BrkSwSta_flg/1 -> VAPM_BrkSwSta_flg_Inproc/1  "VAPM_BrkSwSta_flg"
  VAPM_BrkSwSta_flg_Inproc/1 -> UnitConverter121/1
  UnitConverter121/1 -> VOUTP_BrkSwSta_flg/1  "VOUTP_BrkSwSta_flg"
  VAPM_BrkSwStaTimeOut_flg/1 -> VAPM_BrkSwStaTimeOut_flg_Inproc/1  "VAPM_BrkSwStaTimeOut_flg"
  VAPM_BrkSwStaTimeOut_flg_Inproc/1 -> UnitConverter122/1
  UnitConverter122/1 -> VOUTP_BrkSwStaTimeOut_flg/1  "VOUTP_BrkSwStaTimeOut_flg"
  VAPM_BrkSwV_flg/1 -> VAPM_BrkSwV_flg_Inproc/1  "VAPM_BrkSwV_flg"
  VAPM_BrkSwV_flg_Inproc/1 -> UnitConverter123/1
  UnitConverter123/1 -> VOUTP_BrkSwV_flg/1  "VOUTP_BrkSwV_flg"
  VAPM_BrkSwVTimeOut_flg/1 -> VAPM_BrkSwVTimeOut_flg_Inproc/1  "VAPM_BrkSwVTimeOut_flg"
  VAPM_BrkSwVTimeOut_flg_Inproc/1 -> UnitConverter124/1
  UnitConverter124/1 -> VOUTP_BrkSwVTimeOut_flg/1  "VOUTP_BrkSwVTimeOut_flg"
  VAPM_ESCStandstill_flg/1 -> VAPM_ESCStandstill_flg_Inproc/1  "VAPM_ESCStandstill_flg"
  VAPM_ESCStandstill_flg_Inproc/1 -> UnitConverter125/1
  UnitConverter125/1 -> VOUTP_ESCStandstill_flg/1  "VOUTP_ESCStandstill_flg"
  VAPM_ESCStandstillTimeOut_flg/1 -> VAPM_ESCStandstillTimeOut_flg_Inproc/1  "VAPM_ESCStandstillTimeOut_flg"
  VAPM_ESCStandstillTimeOut_flg_Inproc/1 -> UnitConverter126/1
  UnitConverter126/1 -> VOUTP_ESCStandstillTimeOut_flg/1  "VOUTP_ESCStandstillTimeOut_flg"
  VAPM_ESCAPSSta_enum/1 -> VAPM_ESCAPSSta_enum_Inproc/1  "VAPM_ESCAPSSta_enum"
  VAPM_ESCAPSSta_enum_Inproc/1 -> UnitConverter127/1
  UnitConverter127/1 -> VOUTP_ESCAPSSta_enum/1  "VOUTP_ESCAPSSta_enum"
  VAPM_ESCAPSStaTimeOut_flg/1 -> VAPM_ESCAPSStaTimeOut_flg_Inproc/1  "VAPM_ESCAPSStaTimeOut_flg"
  VAPM_ESCAPSStaTimeOut_flg_Inproc/1 -> UnitConverter128/1
  UnitConverter128/1 -> VOUTP_ESCAPSStaTimeOut_flg/1  "VOUTP_ESCAPSStaTimeOut_flg"
  VAPM_EPBExtReleaseAvail_flg/1 -> VAPM_EPBExtReleaseAvail_flg_Inproc/1  "VAPM_EPBExtReleaseAvail_flg"
  VAPM_EPBExtReleaseAvail_flg_Inproc/1 -> UnitConverter129/1
  UnitConverter129/1 -> VOUTP_EPBExtReleaseAvail_flg/1  "VOUTP_EPBExtReleaseAvail_flg"
  VAPM_EPBExtReleaseAvailTimeOut_flg/1 -> VAPM_EPBExtReleaseAvailTimeOut_flg_Inproc/1  "VAPM_EPBExtReleaseAvailTimeOut_flg"
  VAPM_EPBExtReleaseAvailTimeOut_flg_Inproc/1 -> UnitConverter130/1
  UnitConverter130/1 -> VOUTP_EPBExtReleaseAvailTimeOut_flg/1  "VOUTP_EPBExtReleaseAvailTimeOut_flg"
  VAPM_EPBExtApplyAvail_flg/1 -> VAPM_EPBExtApplyAvail_flg_Inproc/1  "VAPM_EPBExtApplyAvail_flg"
  VAPM_EPBExtApplyAvail_flg_Inproc/1 -> UnitConverter131/1
  UnitConverter131/1 -> VOUTP_EPBExtApplyAvail_flg/1  "VOUTP_EPBExtApplyAvail_flg"
  VAPM_EPBExtApplyAvailTimeOut_flg/1 -> VAPM_EPBExtApplyAvailTimeOut_flg_Inproc/1  "VAPM_EPBExtApplyAvailTimeOut_flg"
  VAPM_EPBExtApplyAvailTimeOut_flg_Inproc/1 -> UnitConverter132/1
  UnitConverter132/1 -> VOUTP_EPBExtApplyAvailTimeOut_flg/1  "VOUTP_EPBExtApplyAvailTimeOut_flg"
  VAPM_EPBErrSta_enum/1 -> VAPM_EPBErrSta_enum_Inproc/1  "VAPM_EPBErrSta_enum"
  VAPM_EPBErrSta_enum_Inproc/1 -> UnitConverter133/1
  UnitConverter133/1 -> VOUTP_EPBErrSta_enum/1  "VOUTP_EPBErrSta_enum"
  VAPM_EPBErrStaTimeOut_flg/1 -> VAPM_EPBErrStaTimeOut_flg_Inproc/1  "VAPM_EPBErrStaTimeOut_flg"
  VAPM_EPBErrStaTimeOut_flg_Inproc/1 -> UnitConverter134/1
  UnitConverter134/1 -> VOUTP_EPBErrStaTimeOut_flg/1  "VOUTP_EPBErrStaTimeOut_flg"
  VAPM_EPBSta_enum/1 -> VAPM_EPBSta_enum_Inproc/1  "VAPM_EPBSta_enum"
  VAPM_EPBSta_enum_Inproc/1 -> UnitConverter135/1
  UnitConverter135/1 -> VOUTP_EPBSta_enum/1  "VOUTP_EPBSta_enum"
  VAPM_EPBStaTimeOut_flg/1 -> VAPM_EPBStaTimeOut_flg_Inproc/1  "VAPM_EPBStaTimeOut_flg"
  VAPM_EPBStaTimeOut_flg_Inproc/1 -> UnitConverter136/1
  UnitConverter136/1 -> VOUTP_EPBStaTimeOut_flg/1  "VOUTP_EPBStaTimeOut_flg"
  VAPM_AVMparkingcancel_enum/1 -> VAPM_AVMparkingcancel_enum_Inproc/1  "VAPM_AVMparkingcancel_enum"
  VAPM_AVMparkingcancel_enum_Inproc/1 -> UnitConverter137/1
  UnitConverter137/1 -> VOUTP_AVMparkingcancel_enum/1  "VOUTP_AVMparkingcancel_enum"
  VAPM_AVMparkingcancelTimeOut_flg/1 -> VAPM_AVMparkingcancelTimeOut_flg_Inproc/1  "VAPM_AVMparkingcancelTimeOut_flg"
  VAPM_AVMparkingcancelTimeOut_flg_Inproc/1 -> UnitConverter138/1
  UnitConverter138/1 -> VOUTP_AVMparkingcancelTimeOut_flg/1  "VOUTP_AVMparkingcancelTimeOut_flg"
  VAPM_AVMparkingexcute_enum/1 -> VAPM_AVMparkingexcute_enum_Inproc/1  "VAPM_AVMparkingexcute_enum"
  VAPM_AVMparkingexcute_enum_Inproc/1 -> UnitConverter139/1
  UnitConverter139/1 -> VOUTP_AVMparkingexcute_enum/1  "VOUTP_AVMparkingexcute_enum"
  VAPM_AVMparkingexcuteTimeOut_flg/1 -> VAPM_AVMparkingexcuteTimeOut_flg_Inproc/1  "VAPM_AVMparkingexcuteTimeOut_flg"
  VAPM_AVMparkingexcuteTimeOut_flg_Inproc/1 -> UnitConverter140/1
  UnitConverter140/1 -> VOUTP_AVMparkingexcuteTimeOut_flg/1  "VOUTP_AVMparkingexcuteTimeOut_flg"
  VAPM_AVMParkingmode_enum/1 -> VAPM_AVMParkingmode_enum_Inproc/1  "VAPM_AVMParkingmode_enum"
  VAPM_AVMParkingmode_enum_Inproc/1 -> UnitConverter141/1
  UnitConverter141/1 -> VOUTP_AVMParkingmode_enum/1  "VOUTP_AVMParkingmode_enum"
  VAPM_AVMParkingmodeTimeOut_flg/1 -> VAPM_AVMParkingmodeTimeOut_flg_Inproc/1  "VAPM_AVMParkingmodeTimeOut_flg"
  VAPM_AVMParkingmodeTimeOut_flg_Inproc/1 -> UnitConverter142/1
  UnitConverter142/1 -> VOUTP_AVMParkingmodeTimeOut_flg/1  "VOUTP_AVMParkingmodeTimeOut_flg"
  VAPM_AVMErrSTA_flg/1 -> VAPM_AVMErrSTA_flg_Inproc/1  "VAPM_AVMErrSTA_flg"
  VAPM_AVMErrSTA_flg_Inproc/1 -> UnitConverter143/1
  UnitConverter143/1 -> VOUTP_AVMErrSTA_flg/1  "VOUTP_AVMErrSTA_flg"
  VAPM_AVMErrSTATimeOut_flg/1 -> VAPM_AVMErrSTATimeOut_flg_Inproc/1  "VAPM_AVMErrSTATimeOut_flg"
  VAPM_AVMErrSTATimeOut_flg_Inproc/1 -> UnitConverter144/1
  UnitConverter144/1 -> VOUTP_AVMErrSTATimeOut_flg/1  "VOUTP_AVMErrSTATimeOut_flg"
  VAPM_IVIStatus_flg/1 -> VAPM_IVIStatus_flg_Inproc/1  "VAPM_IVIStatus_flg"
  VAPM_IVIStatus_flg_Inproc/1 -> UnitConverter145/1
  UnitConverter145/1 -> VOUTP_IVIStatus_flg/1  "VOUTP_IVIStatus_flg"
  VAPM_IVIStatusTimeOut_flg/1 -> VAPM_IVIStatusTimeOut_flg_Inproc/1  "VAPM_IVIStatusTimeOut_flg"
  VAPM_IVIStatusTimeOut_flg_Inproc/1 -> UnitConverter146/1
  UnitConverter146/1 -> VOUTP_IVIStatusTimeOut_flg/1  "VOUTP_IVIStatusTimeOut_flg"
  VAPM_CAASSw_enum/1 -> VAPM_CAASSw_enum_Inproc/1  "VAPM_CAASSw_enum"
  VAPM_CAASSw_enum_Inproc/1 -> UnitConverter147/1
  UnitConverter147/1 -> VOUTP_CAASSw_enum/1  "VOUTP_CAASSw_enum"
  VAPM_CAASSwTimeOut_flg/1 -> VAPM_CAASSwTimeOut_flg_Inproc/1  "VAPM_CAASSwTimeOut_flg"
  VAPM_CAASSwTimeOut_flg_Inproc/1 -> UnitConverter148/1
  UnitConverter148/1 -> VOUTP_CAASSwTimeOut_flg/1  "VOUTP_CAASSwTimeOut_flg"
  VAPM_IVIScreen_enum/1 -> VAPM_IVIScreen_enum_Inproc/1  "VAPM_IVIScreen_enum"
  VAPM_IVIScreen_enum_Inproc/1 -> UnitConverter149/1
  UnitConverter149/1 -> VOUTP_IVIScreen_enum/1  "VOUTP_IVIScreen_enum"
  VAPM_IVIScreenTimeOut_flg/1 -> VAPM_IVIScreenTimeOut_flg_Inproc/1  "VAPM_IVIScreenTimeOut_flg"
  VAPM_IVIScreenTimeOut_flg_Inproc/1 -> UnitConverter150/1
  UnitConverter150/1 -> VOUTP_IVIScreenTimeOut_flg/1  "VOUTP_IVIScreenTimeOut_flg"
  VAPM_ABSActive_flg/1 -> VAPM_ABSActive_flg_Inproc/1  "VAPM_ABSActive_flg"
  VAPM_ABSActive_flg_Inproc/1 -> UnitConverter151/1
  UnitConverter151/1 -> VOUTP_ABSActive_flg/1  "VOUTP_ABSActive_flg"
  VAPM_ABSActiveTimeOut_flg/1 -> VAPM_ABSActiveTimeOut_flg_Inproc/1  "VAPM_ABSActiveTimeOut_flg"
  VAPM_ABSActiveTimeOut_flg_Inproc/1 -> UnitConverter152/1
  UnitConverter152/1 -> VOUTP_ABSActiveTimeOut_flg/1  "VOUTP_ABSActiveTimeOut_flg"
  VAPM_TCSActive_flg/1 -> VAPM_TCSActive_flg_Inproc/1  "VAPM_TCSActive_flg"
  VAPM_TCSActive_flg_Inproc/1 -> UnitConverter153/1
  UnitConverter153/1 -> VOUTP_TCSActive_flg/1  "VOUTP_TCSActive_flg"
  VAPM_TCSActiveTimeOut_flg/1 -> VAPM_TCSActiveTimeOut_flg_Inproc/1  "VAPM_TCSActiveTimeOut_flg"
  VAPM_TCSActiveTimeOut_flg_Inproc/1 -> UnitConverter154/1
  UnitConverter154/1 -> VOUTP_TCSActiveTimeOut_flg/1  "VOUTP_TCSActiveTimeOut_flg"
  VAPM_DriverSeatBeltCmd_flg/1 -> VAPM_DriverSeatBeltCmd_flg_Inproc/1  "VAPM_DriverSeatBeltCmd_flg"
  VAPM_DriverSeatBeltCmd_flg_Inproc/1 -> UnitConverter155/1
  UnitConverter155/1 -> VOUTP_DriverSeatBeltCmd_flg/1  "VOUTP_DriverSeatBeltCmd_flg"
  VAPM_DriverSeatBeltCmdTimeOut_flg/1 -> VAPM_DriverSeatBeltCmdTimeOut_flg_Inproc/1  "VAPM_DriverSeatBeltCmdTimeOut_flg"
  VAPM_DriverSeatBeltCmdTimeOut_flg_Inproc/1 -> UnitConverter156/1
  UnitConverter156/1 -> VOUTP_DriverSeatBeltCmdTimeOut_flg/1  "VOUTP_DriverSeatBeltCmdTimeOut_flg"
  VAPM_APSProgressPCT_pct/1 -> VAPM_APSProgressPCT_pct_Inproc/1  "VAPM_APSProgressPCT_pct"
  VAPM_APSProgressPCT_pct_Inproc/1 -> UnitConverter157/1
  UnitConverter157/1 -> VOUTP_APSProgressPCT_pct/1  "VOUTP_APSProgressPCT_pct"
  VAPM_APSRQDisplay_enum/1 -> VAPM_APSRQDisplay_enum_Inproc/1  "VAPM_APSRQDisplay_enum"
  VAPM_APSRQDisplay_enum_Inproc/1 -> UnitConverter158/1
  UnitConverter158/1 -> VOUTP_APSRQDisplay_enum/1  "VOUTP_APSRQDisplay_enum"
  VAPM_APSSWVer_enum/1 -> VAPM_APSSWVer_enum_Inproc/1  "VAPM_APSSWVer_enum"
  VAPM_APSSWVer_enum_Inproc/1 -> UnitConverter159/1
  UnitConverter159/1 -> VOUTP_APSSWVer_enum/1  "VOUTP_APSSWVer_enum"
  VAPM_APSHWVer_enum/1 -> VAPM_APSHWVer_enum_Inproc/1  "VAPM_APSHWVer_enum"
  VAPM_APSHWVer_enum_Inproc/1 -> UnitConverter160/1
  UnitConverter160/1 -> VOUTP_APSHWVer_enum/1  "VOUTP_APSHWVer_enum"
  VAPM_APSExitCondition_enum/1 -> VAPM_APSExitCondition_enum_Inproc/1  "VAPM_APSExitCondition_enum"
  VAPM_APSExitCondition_enum_Inproc/1 -> UnitConverter161/1
  UnitConverter161/1 -> VOUTP_APSExitCondition_enum/1  "VOUTP_APSExitCondition_enum"
  VAPM_APSAngleTarget_Deg/1 -> VAPM_APSAngleTarget_Deg_Inproc/1  "VAPM_APSAngleTarget_Deg"
  VAPM_APSAngleTarget_Deg_Inproc/1 -> UnitConverter162/1
  UnitConverter162/1 -> VOUTP_APSAngleTarget_Deg/1  "VOUTP_APSAngleTarget_Deg"
  VAPM_APSVRqEPASCtrl_flg/1 -> VAPM_APSVRqEPASCtrl_flg_Inproc/1  "VAPM_APSVRqEPASCtrl_flg"
  VAPM_APSVRqEPASCtrl_flg_Inproc/1 -> UnitConverter163/1
  UnitConverter163/1 -> VOUTP_APSVRqEPASCtrl_flg/1  "VOUTP_APSVRqEPASCtrl_flg"
  VAPM_APSRqEPASCtrl_flg/1 -> VAPM_APSRqEPASCtrl_flg_Inproc/1  "VAPM_APSRqEPASCtrl_flg"
  VAPM_APSRqEPASCtrl_flg_Inproc/1 -> UnitConverter164/1
  UnitConverter164/1 -> VOUTP_APSRqEPASCtrl_flg/1  "VOUTP_APSRqEPASCtrl_flg"
  VAPM_CAASSta_enum/1 -> VAPM_CAASSta_enum_Inproc/1  "VAPM_CAASSta_enum"
  VAPM_CAASSta_enum_Inproc/1 -> UnitConverter165/1
  UnitConverter165/1 -> VOUTP_CAASSta_enum/1  "VOUTP_CAASSta_enum"
  VAPM_DKCPDkeyAreaRAPSSta_enum/1 -> VAPM_DKCPDkeyAreaRAPSSta_enum_Inproc/1  "VAPM_DKCPDkeyAreaRAPSSta_enum"
  VAPM_DKCPDkeyAreaRAPSSta_enum_Inproc/1 -> UnitConverter166/1
  UnitConverter166/1 -> VOUTP_DKCPDkeyAreaRAPSSta_enum/1  "VOUTP_DKCPDkeyAreaRAPSSta_enum"
  VAPM_DKCParkingModeCmd_enum/1 -> VAPM_DKCParkingModeCmd_enum_Inproc/1  "VAPM_DKCParkingModeCmd_enum"
  VAPM_DKCParkingModeCmd_enum_Inproc/1 -> UnitConverter167/1
  UnitConverter167/1 -> VOUTP_DKCParkingModeCmd_enum/1  "VOUTP_DKCParkingModeCmd_enum"
  VAPM_PUIDLowPower_flg/1 -> VAPM_PUIDLowPower_flg_Inproc/1  "VAPM_PUIDLowPower_flg"
  VAPM_PUIDLowPower_flg_Inproc/1 -> UnitConverter168/1
  UnitConverter168/1 -> VOUTP_PUIDLowPower_flg/1  "VOUTP_PUIDLowPower_flg"
  VAPM_CAASVMCReqA_flg/1 -> VAPM_CAASVMCReqA_flg_Inproc/1  "VAPM_CAASVMCReqA_flg"
  VAPM_CAASVMCReqA_flg_Inproc/1 -> UnitConverter169/1
  UnitConverter169/1 -> VOUTP_CAASVMCReqA_flg/1  "VOUTP_CAASVMCReqA_flg"
  VAPM_APSShiftPosnReq_enum/1 -> VAPM_APSShiftPosnReq_enum_Inproc/1  "VAPM_APSShiftPosnReq_enum"
  VAPM_APSShiftPosnReq_enum_Inproc/1 -> UnitConverter170/1
  UnitConverter170/1 -> VOUTP_APSShiftPosnReq_enum/1  "VOUTP_APSShiftPosnReq_enum"
  VAPM_APSSpeedCMD_kph/1 -> VAPM_APSSpeedCMD_kph_Inproc/1  "VAPM_APSSpeedCMD_kph"
  VAPM_APSSpeedCMD_kph_Inproc/1 -> UnitConverter171/1
  UnitConverter171/1 -> VOUTP_APSSpeedCMD_kph/1  "VOUTP_APSSpeedCMD_kph"
  VAPM_APSVMCReqA_flg/1 -> VAPM_APSVMCReqA_flg_Inproc/1  "VAPM_APSVMCReqA_flg"
  VAPM_APSVMCReqA_flg_Inproc/1 -> UnitConverter172/1
  UnitConverter172/1 -> VOUTP_APSVMCReqA_flg/1  "VOUTP_APSVMCReqA_flg"
  VAPM_RAPSBCMLamp_enum/1 -> VAPM_RAPSBCMLamp_enum_Inproc/1  "VAPM_RAPSBCMLamp_enum"
  VAPM_RAPSBCMLamp_enum_Inproc/1 -> UnitConverter173/1
  UnitConverter173/1 -> VOUTP_RAPSBCMLamp_enum/1  "VOUTP_RAPSBCMLamp_enum"
  VAPM_RAPSBCMLockReq_flg/1 -> VAPM_RAPSBCMLockReq_flg_Inproc/1  "VAPM_RAPSBCMLockReq_flg"
  VAPM_RAPSBCMLockReq_flg_Inproc/1 -> UnitConverter174/1
  UnitConverter174/1 -> VOUTP_RAPSBCMLockReq_flg/1  "VOUTP_RAPSBCMLockReq_flg"
  VAPM_APSPwrReq_enum/1 -> VAPM_APSPwrReq_enum_Inproc/1  "VAPM_APSPwrReq_enum"
  VAPM_APSPwrReq_enum_Inproc/1 -> UnitConverter175/1
  UnitConverter175/1 -> VOUTP_APSPwrReq_enum/1  "VOUTP_APSPwrReq_enum"
  VAPM_RAPSErrWarnSta_enum/1 -> VAPM_RAPSErrWarnSta_enum_Inproc/1  "VAPM_RAPSErrWarnSta_enum"
  VAPM_RAPSErrWarnSta_enum_Inproc/1 -> UnitConverter176/1
  UnitConverter176/1 -> VOUTP_RAPSErrWarnSta_enum/1  "VOUTP_RAPSErrWarnSta_enum"
  VAPM_RAPSErrLv1_flg/1 -> VAPM_RAPSErrLv1_flg_Inproc/1  "VAPM_RAPSErrLv1_flg"
  VAPM_RAPSErrLv1_flg_Inproc/1 -> UnitConverter177/1
  UnitConverter177/1 -> VOUTP_RAPSErrLv1_flg/1  "VOUTP_RAPSErrLv1_flg"
  VAPM_IVIUserTakeOverAPSSta_flg/1 -> VAPM_IVIUserTakeOverAPSSta_flg_Inproc/1  "VAPM_IVIUserTakeOverAPSSta_flg"
  VAPM_IVIUserTakeOverAPSSta_flg_Inproc/1 -> UnitConverter178/1
  UnitConverter178/1 -> VOUTP_IVIUserTakeOverAPSSta_flg/1  "VOUTP_IVIUserTakeOverAPSSta_flg"
  VBCM_AntitheftSta_enum/1 -> VBCM_AntitheftSta_enum_Inproc/1  "VBCM_AntitheftSta_enum"
  VBCM_AntitheftSta_enum_Inproc/1 -> UnitConverter179/1
  UnitConverter179/1 -> VOUTP_AntitheftSta_enum/1  "VOUTP_AntitheftSta_enum"
  VBCM_TailgateRemote_enum/1 -> VBCM_TailgateRemote_enum_Inproc/1  "VBCM_TailgateRemote_enum"
  VBCM_TailgateRemote_enum_Inproc/1 -> UnitConverter180/1
  UnitConverter180/1 -> VOUTP_TailgateRemote_enum/1  "VOUTP_TailgateRemote_enum"
  VBCM_HornCtrl_flg/1 -> VBCM_HornCtrl_flg_Inproc/1  "VBCM_HornCtrl_flg"
  VBCM_HornCtrl_flg_Inproc/1 -> UnitConverter181/1
  UnitConverter181/1 -> VOUTP_HornCtrl_flg/1  "VOUTP_HornCtrl_flg"
  VBCM_AllDoorSW_flg/1 -> VBCM_AllDoorSW_flg_Inproc/1  "VBCM_AllDoorSW_flg"
  VBCM_AllDoorSW_flg_Inproc/1 -> UnitConverter182/1
  UnitConverter182/1 -> VOUTP_AllDoorSW_flg/1  "VOUTP_AllDoorSW_flg"
  VBCM_BCMDoorLockSta_flg/1 -> VBCM_BCMDoorLockSta_flg_Inproc/1  "VBCM_BCMDoorLockSta_flg"
  VBCM_BCMDoorLockSta_flg_Inproc/1 -> UnitConverter183/1
  UnitConverter183/1 -> VOUTP_BCMDoorLockSta_flg/1  "VOUTP_BCMDoorLockSta_flg"
  VBCM_AntitheftSeatFlod_flg/1 -> VBCM_AntitheftSeatFlod_flg_Inproc/1  "VBCM_AntitheftSeatFlod_flg"
  VBCM_AntitheftSeatFlod_flg_Inproc/1 -> UnitConverter184/1
  UnitConverter184/1 -> VOUTP_AntitheftSeatFlod_flg/1  "VOUTP_AntitheftSeatFlod_flg"
  VBCM_HoodSW_flg/1 -> VBCM_HoodSW_flg_Inproc/1  "VBCM_HoodSW_flg"
  VBCM_HoodSW_flg_Inproc/1 -> UnitConverter185/1
  UnitConverter185/1 -> VOUTP_HoodSW_flg/1  "VOUTP_HoodSW_flg"
  VBCM_TailgateSW_flg/1 -> VBCM_TailgateSW_flg_Inproc/1  "VBCM_TailgateSW_flg"
  VBCM_TailgateSW_flg_Inproc/1 -> UnitConverter186/1
  UnitConverter186/1 -> VOUTP_TailgateSW_flg/1  "VOUTP_TailgateSW_flg"
  VBCM_DrDoorSW_flg/1 -> VBCM_DrDoorSW_flg_Inproc/1  "VBCM_DrDoorSW_flg"
  VBCM_DrDoorSW_flg_Inproc/1 -> UnitConverter187/1
  UnitConverter187/1 -> VOUTP_DrDoorSW_flg/1  "VOUTP_DrDoorSW_flg"
  VBCM_PsDoorSW_flg/1 -> VBCM_PsDoorSW_flg_Inproc/1  "VBCM_PsDoorSW_flg"
  VBCM_PsDoorSW_flg_Inproc/1 -> UnitConverter188/1
  UnitConverter188/1 -> VOUTP_PsDoorSW_flg/1  "VOUTP_PsDoorSW_flg"
  VBCM_RLDoorSW_flg/1 -> VBCM_RLDoorSW_flg_Inproc/1  "VBCM_RLDoorSW_flg"
  VBCM_RLDoorSW_flg_Inproc/1 -> UnitConverter189/1
  UnitConverter189/1 -> VOUTP_RLDoorSW_flg/1  "VOUTP_RLDoorSW_flg"
  VBCM_RRDoorSW_flg/1 -> VBCM_RRDoorSW_flg_Inproc/1  "VBCM_RRDoorSW_flg"
  VBCM_RRDoorSW_flg_Inproc/1 -> UnitConverter190/1
  UnitConverter190/1 -> VOUTP_RRDoorSW_flg/1  "VOUTP_RRDoorSW_flg"
  VBCM_LockSetting_flg/1 -> VBCM_LockSetting_flg_Inproc/1  "VBCM_LockSetting_flg"
  VBCM_LockSetting_flg_Inproc/1 -> UnitConverter191/1
  UnitConverter191/1 -> VOUTP_LockSetting_flg/1  "VOUTP_LockSetting_flg"
  VBCM_FrChargingDoorCtrl_enum/1 -> VBCM_FrChargingDoorCtrl_enum_Inproc/1  "VBCM_FrChargingDoorCtrl_enum"
  VBCM_FrChargingDoorCtrl_enum_Inproc/1 -> UnitConverter192/1
  UnitConverter192/1 -> VOUTP_FrChargingDoorCtrl_enum/1  "VOUTP_FrChargingDoorCtrl_enum"
  VBCM_RrChargingDoorCtrl_enum/1 -> VBCM_RrChargingDoorCtrl_enum_Inproc/1  "VBCM_RrChargingDoorCtrl_enum"
  VBCM_RrChargingDoorCtrl_enum_Inproc/1 -> UnitConverter193/1
  UnitConverter193/1 -> VOUTP_RrChargingDoorCtrl_enum/1  "VOUTP_RrChargingDoorCtrl_enum"
  VBCM_CrashDetd_flg/1 -> VBCM_CrashDetd_flg_Inproc/1  "VBCM_CrashDetd_flg"
  VBCM_CrashDetd_flg_Inproc/1 -> UnitConverter194/1
  UnitConverter194/1 -> VOUTP_CrashDetd_flg/1  "VOUTP_CrashDetd_flg"
  VBCM_CTDCtrl_enum/1 -> VBCM_CTDCtrl_enum_Inproc/1  "VBCM_CTDCtrl_enum"
  VBCM_CTDCtrl_enum_Inproc/1 -> UnitConverter195/1
  UnitConverter195/1 -> VOUTP_CTDCtrl_enum/1  "VOUTP_CTDCtrl_enum"
  VBCM_DoorLockIND_flg/1 -> VBCM_DoorLockIND_flg_Inproc/1  "VBCM_DoorLockIND_flg"
  VBCM_DoorLockIND_flg_Inproc/1 -> UnitConverter196/1
  UnitConverter196/1 -> VOUTP_DoorLockIND_flg/1  "VOUTP_DoorLockIND_flg"
  VBCM_CTDLockSW_flg/1 -> VBCM_CTDLockSW_flg_Inproc/1  "VBCM_CTDLockSW_flg"
  VBCM_CTDLockSW_flg_Inproc/1 -> UnitConverter197/1
  UnitConverter197/1 -> VOUTP_CTDLockSW_flg/1  "VOUTP_CTDLockSW_flg"
  VBCM_Dimmer_pct/1 -> VBCM_Dimmer_pct_Inproc/1  "VBCM_Dimmer_pct"
  VBCM_Dimmer_pct_Inproc/1 -> UnitConverter198/1
  UnitConverter198/1 -> VOUTP_Dimmer_pct/1  "VOUTP_Dimmer_pct"
  VBCM_DimmerEN_flg/1 -> VBCM_DimmerEN_flg_Inproc/1  "VBCM_DimmerEN_flg"
  VBCM_DimmerEN_flg_Inproc/1 -> UnitConverter199/1
  UnitConverter199/1 -> VOUTP_DimmerEN_flg/1  "VOUTP_DimmerEN_flg"
  VBCM_PosLamp_flg/1 -> VBCM_PosLamp_flg_Inproc/1  "VBCM_PosLamp_flg"
  VBCM_PosLamp_flg_Inproc/1 -> UnitConverter200/1
  UnitConverter200/1 -> VOUTP_PosLamp_flg/1  "VOUTP_PosLamp_flg"
  VBCM_LBeam_flg/1 -> VBCM_LBeam_flg_Inproc/1  "VBCM_LBeam_flg"
  VBCM_LBeam_flg_Inproc/1 -> UnitConverter201/1
  UnitConverter201/1 -> VOUTP_LBeam_flg/1  "VOUTP_LBeam_flg"
  VBCM_HBeam_flg/1 -> VBCM_HBeam_flg_Inproc/1  "VBCM_HBeam_flg"
  VBCM_HBeam_flg_Inproc/1 -> UnitConverter202/1
  UnitConverter202/1 -> VOUTP_HBeam_flg/1  "VOUTP_HBeam_flg"
  VBCM_RrFogLamp_flg/1 -> VBCM_RrFogLamp_flg_Inproc/1  "VBCM_RrFogLamp_flg"
  VBCM_RrFogLamp_flg_Inproc/1 -> UnitConverter203/1
  UnitConverter203/1 -> VOUTP_RrFogLamp_flg/1  "VOUTP_RrFogLamp_flg"
  VBCM_BrakeLamp_flg/1 -> VBCM_BrakeLamp_flg_Inproc/1  "VBCM_BrakeLamp_flg"
  VBCM_BrakeLamp_flg_Inproc/1 -> UnitConverter204/1
  UnitConverter204/1 -> VOUTP_BrakeLamp_flg/1  "VOUTP_BrakeLamp_flg"
  VBCM_ReverseLamp_flg/1 -> VBCM_ReverseLamp_flg_Inproc/1  "VBCM_ReverseLamp_flg"
  VBCM_ReverseLamp_flg_Inproc/1 -> UnitConverter205/1
  UnitConverter205/1 -> VOUTP_ReverseLamp_flg/1  "VOUTP_ReverseLamp_flg"
  VBCM_LDRL_flg/1 -> VBCM_LDRL_flg_Inproc/1  "VBCM_LDRL_flg"
  VBCM_LDRL_flg_Inproc/1 -> UnitConverter206/1
  UnitConverter206/1 -> VOUTP_LDRL_flg/1  "VOUTP_LDRL_flg"
  VBCM_RDRL_flg/1 -> VBCM_RDRL_flg_Inproc/1  "VBCM_RDRL_flg"
  VBCM_RDRL_flg_Inproc/1 -> UnitConverter207/1
  UnitConverter207/1 -> VOUTP_RDRL_flg/1  "VOUTP_RDRL_flg"
  VBCM_LBSD_flg/1 -> VBCM_LBSD_flg_Inproc/1  "VBCM_LBSD_flg"
  VBCM_LBSD_flg_Inproc/1 -> UnitConverter208/1
  UnitConverter208/1 -> VOUTP_LBSD_flg/1  "VOUTP_LBSD_flg"
  VBCM_RBSD_flg/1 -> VBCM_RBSD_flg_Inproc/1  "VBCM_RBSD_flg"
  VBCM_RBSD_flg_Inproc/1 -> UnitConverter209/1
  UnitConverter209/1 -> VOUTP_RBSD_flg/1  "VOUTP_RBSD_flg"
  VBCM_HazardSW_flg/1 -> VBCM_HazardSW_flg_Inproc/1  "VBCM_HazardSW_flg"
  VBCM_HazardSW_flg_Inproc/1 -> UnitConverter210/1
  UnitConverter210/1 -> VOUTP_HazardSW_flg/1  "VOUTP_HazardSW_flg"
  VBCM_LTurnLP_flg/1 -> VBCM_LTurnLP_flg_Inproc/1  "VBCM_LTurnLP_flg"
  VBCM_LTurnLP_flg_Inproc/1 -> UnitConverter211/1
  UnitConverter211/1 -> VOUTP_LTurnLP_flg/1  "VOUTP_LTurnLP_flg"
  VBCM_RTurnLP_flg/1 -> VBCM_RTurnLP_flg_Inproc/1  "VBCM_RTurnLP_flg"
  VBCM_RTurnLP_flg_Inproc/1 -> UnitConverter212/1
  UnitConverter212/1 -> VOUTP_RTurnLP_flg/1  "VOUTP_RTurnLP_flg"
  VBCM_BCMBuzzerReq_flg/1 -> VBCM_BCMBuzzerReq_flg_Inproc/1  "VBCM_BCMBuzzerReq_flg"
  VBCM_BCMBuzzerReq_flg_Inproc/1 -> UnitConverter213/1
  UnitConverter213/1 -> VOUTP_BCMBuzzerReq_flg/1  "VOUTP_BCMBuzzerReq_flg"
  VBCM_MirrorCtrl_enum/1 -> VBCM_MirrorCtrl_enum_Inproc/1  "VBCM_MirrorCtrl_enum"
  VBCM_MirrorCtrl_enum_Inproc/1 -> UnitConverter214/1
  UnitConverter214/1 -> VOUTP_MirrorCtrl_enum/1  "VOUTP_MirrorCtrl_enum"
  VBCM_MirrorDefog_flg/1 -> VBCM_MirrorDefog_flg_Inproc/1  "VBCM_MirrorDefog_flg"
  VBCM_MirrorDefog_flg_Inproc/1 -> UnitConverter215/1
  UnitConverter215/1 -> VOUTP_MirrorDefog_flg/1  "VOUTP_MirrorDefog_flg"
  VBCM_RrDefog_flg/1 -> VBCM_RrDefog_flg_Inproc/1  "VBCM_RrDefog_flg"
  VBCM_RrDefog_flg_Inproc/1 -> UnitConverter216/1
  UnitConverter216/1 -> VOUTP_RrDefog_flg/1  "VOUTP_RrDefog_flg"
  VBCM_RoomLampH_flg/1 -> VBCM_RoomLampH_flg_Inproc/1  "VBCM_RoomLampH_flg"
  VBCM_RoomLampH_flg_Inproc/1 -> UnitConverter217/1
  UnitConverter217/1 -> VOUTP_RoomLampH_flg/1  "VOUTP_RoomLampH_flg"
  VBCM_RoomLampL_flg/1 -> VBCM_RoomLampL_flg_Inproc/1  "VBCM_RoomLampL_flg"
  VBCM_RoomLampL_flg_Inproc/1 -> UnitConverter218/1
  UnitConverter218/1 -> VOUTP_RoomLampL_flg/1  "VOUTP_RoomLampL_flg"
  VBCM_TrunkRel_flg/1 -> VBCM_TrunkRel_flg_Inproc/1  "VBCM_TrunkRel_flg"
  VBCM_TrunkRel_flg_Inproc/1 -> UnitConverter219/1
  UnitConverter219/1 -> VOUTP_TrunkRel_flg/1  "VOUTP_TrunkRel_flg"
  VBCM_TailgateHDSW_flg/1 -> VBCM_TailgateHDSW_flg_Inproc/1  "VBCM_TailgateHDSW_flg"
  VBCM_TailgateHDSW_flg_Inproc/1 -> UnitConverter220/1
  UnitConverter220/1 -> VOUTP_TailgateHDSW_flg/1  "VOUTP_TailgateHDSW_flg"
  VBCM_FrWiperL_flg/1 -> VBCM_FrWiperL_flg_Inproc/1  "VBCM_FrWiperL_flg"
  VBCM_FrWiperL_flg_Inproc/1 -> UnitConverter221/1
  UnitConverter221/1 -> VOUTP_FrWiperL_flg/1  "VOUTP_FrWiperL_flg"
  VBCM_FrWiperH_flg/1 -> VBCM_FrWiperH_flg_Inproc/1  "VBCM_FrWiperH_flg"
  VBCM_FrWiperH_flg_Inproc/1 -> UnitConverter222/1
  UnitConverter222/1 -> VOUTP_FrWiperH_flg/1  "VOUTP_FrWiperH_flg"
  VBCM_RrWiper_flg/1 -> VBCM_RrWiper_flg_Inproc/1  "VBCM_RrWiper_flg"
  VBCM_RrWiper_flg_Inproc/1 -> UnitConverter223/1
  UnitConverter223/1 -> VOUTP_RrWiper_flg/1  "VOUTP_RrWiper_flg"
  VBCM_WasherCtrl_enum/1 -> VBCM_WasherCtrl_enum_Inproc/1  "VBCM_WasherCtrl_enum"
  VBCM_WasherCtrl_enum_Inproc/1 -> UnitConverter224/1
  UnitConverter224/1 -> VOUTP_WasherCtrl_enum/1  "VOUTP_WasherCtrl_enum"
  VBCM_WiperFixMode_flg/1 -> VBCM_WiperFixMode_flg_Inproc/1  "VBCM_WiperFixMode_flg"
  VBCM_WiperFixMode_flg_Inproc/1 -> UnitConverter225/1
  UnitConverter225/1 -> VOUTP_WiperFixMode_flg/1  "VOUTP_WiperFixMode_flg"
  VBCM_AmbLightBreath1_enum/1 -> VBCM_AmbLightBreath1_enum_Inproc/1  "VBCM_AmbLightBreath1_enum"
  VBCM_AmbLightBreath1_enum_Inproc/1 -> UnitConverter226/1
  UnitConverter226/1 -> VOUTP_AmbLightBreath1_enum/1  "VOUTP_AmbLightBreath1_enum"
  VBCM_AmbLightBreath2_enum/1 -> VBCM_AmbLightBreath2_enum_Inproc/1  "VBCM_AmbLightBreath2_enum"
  VBCM_AmbLightBreath2_enum_Inproc/1 -> UnitConverter227/1
  UnitConverter227/1 -> VOUTP_AmbLightBreath2_enum/1  "VOUTP_AmbLightBreath2_enum"
  VBCM_AmbLightBreath3_enum/1 -> VBCM_AmbLightBreath3_enum_Inproc/1  "VBCM_AmbLightBreath3_enum"
  VBCM_AmbLightBreath3_enum_Inproc/1 -> UnitConverter228/1
  UnitConverter228/1 -> VOUTP_AmbLightBreath3_enum/1  "VOUTP_AmbLightBreath3_enum"
  VBCM_AmbLightBreath4_enum/1 -> VBCM_AmbLightBreath4_enum_Inproc/1  "VBCM_AmbLightBreath4_enum"
  VBCM_AmbLightBreath4_enum_Inproc/1 -> UnitConverter229/1
  UnitConverter229/1 -> VOUTP_AmbLightBreath4_enum/1  "VOUTP_AmbLightBreath4_enum"
  VBCM_AmbLightBreath5_enum/1 -> VBCM_AmbLightBreath5_enum_Inproc/1  "VBCM_AmbLightBreath5_enum"
  VBCM_AmbLightBreath5_enum_Inproc/1 -> UnitConverter230/1
  UnitConverter230/1 -> VOUTP_AmbLightBreath5_enum/1  "VOUTP_AmbLightBreath5_enum"
  VBCM_AmbLightBreath6_enum/1 -> VBCM_AmbLightBreath6_enum_Inproc/1  "VBCM_AmbLightBreath6_enum"
  VBCM_AmbLightBreath6_enum_Inproc/1 -> UnitConverter231/1
  UnitConverter231/1 -> VOUTP_AmbLightBreath6_enum/1  "VOUTP_AmbLightBreath6_enum"
  VBCM_AmbLightBrightness1_enum/1 -> VBCM_AmbLightBrightness1_enum_Inproc/1  "VBCM_AmbLightBrightness1_enum"
  VBCM_AmbLightBrightness1_enum_Inproc/1 -> UnitConverter232/1
  UnitConverter232/1 -> VOUTP_AmbLightBrightness1_enum/1  "VOUTP_AmbLightBrightness1_enum"
  VBCM_AmbLightBrightness2_enum/1 -> VBCM_AmbLightBrightness2_enum_Inproc/1  "VBCM_AmbLightBrightness2_enum"
  VBCM_AmbLightBrightness2_enum_Inproc/1 -> UnitConverter233/1
  UnitConverter233/1 -> VOUTP_AmbLightBrightness2_enum/1  "VOUTP_AmbLightBrightness2_enum"
  VBCM_AmbLightBrightness3_enum/1 -> VBCM_AmbLightBrightness3_enum_Inproc/1  "VBCM_AmbLightBrightness3_enum"
  VBCM_AmbLightBrightness3_enum_Inproc/1 -> UnitConverter234/1
  UnitConverter234/1 -> VOUTP_AmbLightBrightness3_enum/1  "VOUTP_AmbLightBrightness3_enum"
  VBCM_AmbLightBrightness4_enum/1 -> VBCM_AmbLightBrightness4_enum_Inproc/1  "VBCM_AmbLightBrightness4_enum"
  VBCM_AmbLightBrightness4_enum_Inproc/1 -> UnitConverter235/1
  UnitConverter235/1 -> VOUTP_AmbLightBrightness4_enum/1  "VOUTP_AmbLightBrightness4_enum"
  VBCM_AmbLightBrightness5_enum/1 -> VBCM_AmbLightBrightness5_enum_Inproc/1  "VBCM_AmbLightBrightness5_enum"
  VBCM_AmbLightBrightness5_enum_Inproc/1 -> UnitConverter236/1
  UnitConverter236/1 -> VOUTP_AmbLightBrightness5_enum/1  "VOUTP_AmbLightBrightness5_enum"
  VBCM_AmbLightBrightness6_enum/1 -> VBCM_AmbLightBrightness6_enum_Inproc/1  "VBCM_AmbLightBrightness6_enum"
  VBCM_AmbLightBrightness6_enum_Inproc/1 -> UnitConverter237/1
  UnitConverter237/1 -> VOUTP_AmbLightBrightness6_enum/1  "VOUTP_AmbLightBrightness6_enum"
  VBCM_AmbLightColor1_enum/1 -> VBCM_AmbLightColor1_enum_Inproc/1  "VBCM_AmbLightColor1_enum"
  VBCM_AmbLightColor1_enum_Inproc/1 -> UnitConverter238/1
  UnitConverter238/1 -> VOUTP_AmbLightColor1_enum/1  "VOUTP_AmbLightColor1_enum"
  VBCM_AmbLightColor2_enum/1 -> VBCM_AmbLightColor2_enum_Inproc/1  "VBCM_AmbLightColor2_enum"
  VBCM_AmbLightColor2_enum_Inproc/1 -> UnitConverter239/1
  UnitConverter239/1 -> VOUTP_AmbLightColor2_enum/1  "VOUTP_AmbLightColor2_enum"
  VBCM_AmbLightColor3_enum/1 -> VBCM_AmbLightColor3_enum_Inproc/1  "VBCM_AmbLightColor3_enum"
  VBCM_AmbLightColor3_enum_Inproc/1 -> UnitConverter240/1
  UnitConverter240/1 -> VOUTP_AmbLightColor3_enum/1  "VOUTP_AmbLightColor3_enum"
  VBCM_AmbLightColor4_enum/1 -> VBCM_AmbLightColor4_enum_Inproc/1  "VBCM_AmbLightColor4_enum"
  VBCM_AmbLightColor4_enum_Inproc/1 -> UnitConverter241/1
  UnitConverter241/1 -> VOUTP_AmbLightColor4_enum/1  "VOUTP_AmbLightColor4_enum"
  VBCM_AmbLightColor5_enum/1 -> VBCM_AmbLightColor5_enum_Inproc/1  "VBCM_AmbLightColor5_enum"
  VBCM_AmbLightColor5_enum_Inproc/1 -> UnitConverter242/1
  UnitConverter242/1 -> VOUTP_AmbLightColor5_enum/1  "VOUTP_AmbLightColor5_enum"
  VBCM_AmbLightColor6_enum/1 -> VBCM_AmbLightColor6_enum_Inproc/1  "VBCM_AmbLightColor6_enum"
  VBCM_AmbLightColor6_enum_Inproc/1 -> UnitConverter243/1
  UnitConverter243/1 -> VOUTP_AmbLightColor6_enum/1  "VOUTP_AmbLightColor6_enum"
  VBCM_LampPwr_flg/1 -> VBCM_LampPwr_flg_Inproc/1  "VBCM_LampPwr_flg"
  VBCM_LampPwr_flg_Inproc/1 -> UnitConverter244/1
  UnitConverter244/1 -> VOUTP_LampPwr_flg/1  "VOUTP_LampPwr_flg"
  VBCM_SPTGDet_flg/1 -> VBCM_SPTGDet_flg_Inproc/1  "VBCM_SPTGDet_flg"
  VBCM_SPTGDet_flg_Inproc/1 -> UnitConverter245/1
  UnitConverter245/1 -> VOUTP_SPTGDet_flg/1  "VOUTP_SPTGDet_flg"
  VBCM_APSOpenPTG_flg/1 -> VBCM_APSOpenPTG_flg_Inproc/1  "VBCM_APSOpenPTG_flg"
  VBCM_APSOpenPTG_flg_Inproc/1 -> UnitConverter246/1
  UnitConverter246/1 -> VOUTP_APSOpenPTG_flg/1  "VOUTP_APSOpenPTG_flg"
  VBCM_FollowMe_flg/1 -> VBCM_FollowMe_flg_Inproc/1  "VBCM_FollowMe_flg"
  VBCM_FollowMe_flg_Inproc/1 -> UnitConverter247/1
  UnitConverter247/1 -> VOUTP_FollowMe_flg/1  "VOUTP_FollowMe_flg"
  VBCM_IVIRST_flg/1 -> VBCM_IVIRST_flg_Inproc/1  "VBCM_IVIRST_flg"
  VBCM_IVIRST_flg_Inproc/1 -> UnitConverter248/1
  UnitConverter248/1 -> VOUTP_IVIRST_flg/1  "VOUTP_IVIRST_flg"
  VBCM_CountAlarm_enum/1 -> VBCM_CountAlarm_enum_Inproc/1  "VBCM_CountAlarm_enum"
  VBCM_CountAlarm_enum_Inproc/1 -> UnitConverter249/1
  UnitConverter249/1 -> VOUTP_CountAlarm_enum/1  "VOUTP_CountAlarm_enum"
  VBCM_MFSWTri_flg/1 -> VBCM_MFSWTri_flg_Inproc/1  "VBCM_MFSWTri_flg"
  VBCM_MFSWTri_flg_Inproc/1 -> UnitConverter250/1
  UnitConverter250/1 -> VOUTP_MFSWTri_flg/1  "VOUTP_MFSWTri_flg"
  VBCM_MirrorFlodPos_flg/1 -> VBCM_MirrorFlodPos_flg_Inproc/1  "VBCM_MirrorFlodPos_flg"
  VBCM_MirrorFlodPos_flg_Inproc/1 -> UnitConverter251/1
  UnitConverter251/1 -> VOUTP_MirrorFlodPos_flg/1  "VOUTP_MirrorFlodPos_flg"
  VBCM_FuelDoorPos_flg/1 -> VBCM_FuelDoorPos_flg_Inproc/1  "VBCM_FuelDoorPos_flg"
  VBCM_FuelDoorPos_flg_Inproc/1 -> UnitConverter252/1
  UnitConverter252/1 -> VOUTP_FuelDoorPos_flg/1  "VOUTP_FuelDoorPos_flg"
  VBCM_MFRDNBrightReq_pct/1 -> VBCM_MFRDNBrightReq_pct_Inproc/1  "VBCM_MFRDNBrightReq_pct"
  VBCM_MFRDNBrightReq_pct_Inproc/1 -> UnitConverter253/1
  UnitConverter253/1 -> VOUTP_MFRDNBrightReq_pct/1  "VOUTP_MFRDNBrightReq_pct"
  VBCM_PTGInnerSW2_enum/1 -> VBCM_PTGInnerSW2_enum_Inproc/1  "VBCM_PTGInnerSW2_enum"
  VBCM_PTGInnerSW2_enum_Inproc/1 -> UnitConverter254/1
  UnitConverter254/1 -> VOUTP_PTGInnerSW2_enum/1  "VOUTP_PTGInnerSW2_enum"
  VBCM_DrvWdwCtrlCmd_pct/1 -> VBCM_DrvWdwCtrlCmd_pct_Inproc/1  "VBCM_DrvWdwCtrlCmd_pct"
  VBCM_DrvWdwCtrlCmd_pct_Inproc/1 -> UnitConverter255/1
  UnitConverter255/1 -> VOUTP_DrvWdwCtrlCmd_pct/1  "VOUTP_DrvWdwCtrlCmd_pct"
  VBCM_PasWdwCtrlCmd_pct/1 -> VBCM_PasWdwCtrlCmd_pct_Inproc/1  "VBCM_PasWdwCtrlCmd_pct"
  VBCM_PasWdwCtrlCmd_pct_Inproc/1 -> UnitConverter256/1
  UnitConverter256/1 -> VOUTP_PasWdwCtrlCmd_pct/1  "VOUTP_PasWdwCtrlCmd_pct"
  VBCM_DrRWdwCtrlCmd_pct/1 -> VBCM_DrRWdwCtrlCmd_pct_Inproc/1  "VBCM_DrRWdwCtrlCmd_pct"
  VBCM_DrRWdwCtrlCmd_pct_Inproc/1 -> UnitConverter257/1
  UnitConverter257/1 -> VOUTP_DrRWdwCtrlCmd_pct/1  "VOUTP_DrRWdwCtrlCmd_pct"
  VBCM_PsRWdwCtrlCmd_pct/1 -> VBCM_PsRWdwCtrlCmd_pct_Inproc/1  "VBCM_PsRWdwCtrlCmd_pct"
  VBCM_PsRWdwCtrlCmd_pct_Inproc/1 -> UnitConverter258/1
  UnitConverter258/1 -> VOUTP_PsRWdwCtrlCmd_pct/1  "VOUTP_PsRWdwCtrlCmd_pct"
  VBCM_APMDoorControlSta_flg/1 -> VBCM_APMDoorControlSta_flg_Inproc/1  "VBCM_APMDoorControlSta_flg"
  VBCM_APMDoorControlSta_flg_Inproc/1 -> UnitConverter259/1
  UnitConverter259/1 -> VOUTP_APMDoorControlSta_flg/1  "VOUTP_APMDoorControlSta_flg"
  VBCM_AmbFunEN_flg/1 -> VBCM_AmbFunEN_flg_Inproc/1  "VBCM_AmbFunEN_flg"
  VBCM_AmbFunEN_flg_Inproc/1 -> UnitConverter260/1
  UnitConverter260/1 -> VOUTP_AmbFunEN_flg/1  "VOUTP_AmbFunEN_flg"
  VBCM_AmbWelEN_flg/1 -> VBCM_AmbWelEN_flg_Inproc/1  "VBCM_AmbWelEN_flg"
  VBCM_AmbWelEN_flg_Inproc/1 -> UnitConverter261/1
  UnitConverter261/1 -> VOUTP_AmbWelEN_flg/1  "VOUTP_AmbWelEN_flg"
  VBCM_AmbDimEN_flg/1 -> VBCM_AmbDimEN_flg_Inproc/1  "VBCM_AmbDimEN_flg"
  VBCM_AmbDimEN_flg_Inproc/1 -> UnitConverter262/1
  UnitConverter262/1 -> VOUTP_AmbDimEN_flg/1  "VOUTP_AmbDimEN_flg"
  VBCM_AmbLinkDriSta_flg/1 -> VBCM_AmbLinkDriSta_flg_Inproc/1  "VBCM_AmbLinkDriSta_flg"
  VBCM_AmbLinkDriSta_flg_Inproc/1 -> UnitConverter263/1
  UnitConverter263/1 -> VOUTP_AmbLinkDriSta_flg/1  "VOUTP_AmbLinkDriSta_flg"
  VBCM_AmbPwrWarnEN_flg/1 -> VBCM_AmbPwrWarnEN_flg_Inproc/1  "VBCM_AmbPwrWarnEN_flg"
  VBCM_AmbPwrWarnEN_flg_Inproc/1 -> UnitConverter264/1
  UnitConverter264/1 -> VOUTP_AmbPwrWarnEN_flg/1  "VOUTP_AmbPwrWarnEN_flg"
  VBCM_AmbODAEN_flg/1 -> VBCM_AmbODAEN_flg_Inproc/1  "VBCM_AmbODAEN_flg"
  VBCM_AmbODAEN_flg_Inproc/1 -> UnitConverter265/1
  UnitConverter265/1 -> VOUTP_AmbODAEN_flg/1  "VOUTP_AmbODAEN_flg"
  VBCM_AmbColorSta_enum/1 -> VBCM_AmbColorSta_enum_Inproc/1  "VBCM_AmbColorSta_enum"
  VBCM_AmbColorSta_enum_Inproc/1 -> UnitConverter266/1
  UnitConverter266/1 -> VOUTP_AmbColorSta_enum/1  "VOUTP_AmbColorSta_enum"
  VBCM_AmbBrightSta_enum/1 -> VBCM_AmbBrightSta_enum_Inproc/1  "VBCM_AmbBrightSta_enum"
  VBCM_AmbBrightSta_enum_Inproc/1 -> UnitConverter267/1
  UnitConverter267/1 -> VOUTP_AmbBrightSta_enum/1  "VOUTP_AmbBrightSta_enum"
  VBCM_LockAlarm_enum/1 -> VBCM_LockAlarm_enum_Inproc/1  "VBCM_LockAlarm_enum"
  VBCM_LockAlarm_enum_Inproc/1 -> UnitConverter268/1
  UnitConverter268/1 -> VOUTP_LockAlarm_enum/1  "VOUTP_LockAlarm_enum"
  VBCM_ATCtrl_enum/1 -> VBCM_ATCtrl_enum_Inproc/1  "VBCM_ATCtrl_enum"
  VBCM_ATCtrl_enum_Inproc/1 -> UnitConverter269/1
  UnitConverter269/1 -> VOUTP_ATCtrl_enum/1  "VOUTP_ATCtrl_enum"
  VBCM_fUnlockSingle_flg/1 -> VBCM_fUnlockSingle_flg_Inproc/1  "VBCM_fUnlockSingle_flg"
  VBCM_fUnlockSingle_flg_Inproc/1 -> UnitConverter270/1
  UnitConverter270/1 -> VOUTP_fUnlockSingle_flg/1  "VOUTP_fUnlockSingle_flg"
  VBCM_UserNow_enum/1 -> VBCM_UserNow_enum_Inproc/1  "VBCM_UserNow_enum"
  VBCM_UserNow_enum_Inproc/1 -> UnitConverter271/1
  UnitConverter271/1 -> VOUTP_UserNow_enum/1  "VOUTP_UserNow_enum"
  VBCM_AmbFunENFlash_enum/1 -> VBCM_AmbFunENFlash_enum_Inproc/1  "VBCM_AmbFunENFlash_enum"
  VBCM_AmbFunENFlash_enum_Inproc/1 -> UnitConverter272/1
  UnitConverter272/1 -> VOUTP_AmbFunENFlash_enum/1  "VOUTP_AmbFunENFlash_enum"
  VBCM_AmbWelENFlash_enum/1 -> VBCM_AmbWelENFlash_enum_Inproc/1  "VBCM_AmbWelENFlash_enum"
  VBCM_AmbWelENFlash_enum_Inproc/1 -> UnitConverter273/1
  UnitConverter273/1 -> VOUTP_AmbWelENFlash_enum/1  "VOUTP_AmbWelENFlash_enum"
  VBCM_AmbDimENFlash_enum/1 -> VBCM_AmbDimENFlash_enum_Inproc/1  "VBCM_AmbDimENFlash_enum"
  VBCM_AmbDimENFlash_enum_Inproc/1 -> UnitConverter274/1
